simulink model "RB_KAIROS_ImpControl_OpSpace_quat_2020b_safety"  (R2020b)
(part 9 of 17)

C = reshape([0.0,0.0,-q6d.*(-t8850-t8864-t10622+t10627+t11928+t12142-t12808-t12904-t14301-t14305-t14353-t14354+t15516+t15519+t15537+t15539+t15543+t15568+t15569+t15587+t15625+t15626+t15634+t15736+t15867+t15870+t15882+t15885+t15909+t15910+t15967+t15969)-q3d.*(-t5516-t5522-t5589-t5597-t6249-t6602-t7763-t8161+t8844+t8878+t9078+t9084+t9425+t9485+t10324+t10356+t10401+t10512+t10538+t10559+t10594+t10651+t10900+t10919+t10934+t11254+t11258+t11359+t11365+t11539+t11540+t11578+t11596+t11706+t11713+t11715+t11812+t12043+t12084+t12309+t12313+t12340+t12555+t12845+t13109+t13116+t13277+t13286+t13318+t13710+t13918+t13933+t14059+t14102+t14109+t14118+t14133+t14236+t14356+t14358+t14378+t14551+t14817+t14826+t15052+t15058+t15246+t15261+t15399+t15423+t15425+t15433+t15438+t15509+t15510+t15514+t15524+t15613+t15947+t15954+t15988+t15990+t16002+t16003+t16022+t16024)-q4d.*(t5283+t5287+t7042+t7055+t9480+t9626+t10643+t10682+t10838+t10843+t11138+t11325-t12230+t12246+t12314-t12541+t12547-t12593-t12625+t12700+t12876+t12880+t13094+t13095+t13193-t13254-t13453-t13465+t13655+t13721+t13739-t13754-t13765+t13953+t14036+t14149+t14306+t14630+t14634+t14834+t14836-t15211-t15339-t15390-t15410-t15412-t15492-t15493-t15497+t15901+t15949+(t5598.*(t4540+t5.*(t2425-t2468)))./4.0+(t13380.*(t10158+t16.*(t4542-t6448)))./4.0+(t14541.*(t10403+t9.*(t10158+t16.*(t4542-t6448)).*7.35522e-1))./4.0+(t12689.*(t3418-t3879+t4324+t11855+t9.*(t71-t391).*4.5305948634e-2+t17.*(t426-t581).*7.35522e-1+t9.*(t9166-t11658).*7.35522e-1))./4.0+(t2701.*(t5122+t5.*(t2425-t2468).*3.587895))./4.0+(t9830.*(t5124-t6795))./4.0+(t9884.*(t5110-t6808))./4.0+(t10964.*(t4542-t6448))./4.0+(t10936.*(t1589-t2213-t4346+t4355+t9454+t11863+t2772.*(t71-t391)+t2775.*(t71-t391)))./4.0+(t12705.*(t3423+t3845+t3888+t3925+t4339+t9.*(t210+t2107+t7423+t9121).*7.35522e-1+t17.*(t9166-t11658).*7.35522e-1))./4.0+(t12867.*(t10384+t16.*(t4542-t6448).*1.666555))./4.0+(t11340.*(t249-t391.*(1.1e+1./1.25e+2)-t1912.*4.252e-3+t3505+t13496+t693.*(t71-t391)+t784.*(t71-t391)))./4.0+(t14918.*(t10174+t9.*(t10158+t16.*(t4542-t6448))))./4.0+(t12953.*(t2091+t2497+t2579+t2680+t3516+t9.*(t210+t2107+t7423+t9121)+t17.*(t9166-t11658)))./4.0+(t12945.*(t1987-t2621+t3452+t11654+t9.*(t71-t391).*6.1597e-2+t17.*(t426-t581)+t9.*(t9166-t11658)))./4.0+t15.*t12396.*(t4542-t6448).*3.064865e-1+(t15.*t13140.*(t4542-t6448))./4.0)-q2d.*t16467-q1d.*t16482+q7d.*(t10657+t10678+t12523+t12525-t13534-t13699-t16028+t16029+t16034-t16035+t16042+t16061+(t14185.*(t3418-t3879+t4324+t11855+t9.*(t71-t391).*4.5305948634e-2+t17.*(t426-t581).*7.35522e-1+t9.*(t9166-t11658).*7.35522e-1))./4.0+(t14280.*(t1987-t2621+t3452+t11654+t9.*(t71-t391).*6.1597e-2+t17.*(t426-t581)+t9.*(t9166-t11658)))./4.0)-q5d.*(t7290+t7292+t8876+t8913+t10169+t10541+t11057+t11063+t12519+t12522+t12610+t12611+t12793+t12805+t14199+t14202+t14263+t14316+t14319+t14331+t14336+t14432+t14466+t14469+t14484+t14516+t14520+t14593+t14594+t14746+t14978+t14983+t15086+t15091+t15198+t15203+t15213+t15382+t15404+t15405+t15408+t15528+t15929+t15930+t15977+t15979+t15995+t15996+t16015+t16016),q7d.*(t10657+t10678+t12523+t12525-t13534-t13699+t15165+t15166+t15271+t15273+(t10149.*(t10403+t9.*(t10158+t16.*(t4542-t6448)).*7.35522e-1))./4.0+(t14185.*(t3418-t3879+t4324-t5228+t5802+t9.*(t71-t391).*4.5305948634e-2+t17.*(t426-t581).*7.35522e-1))./4.0+(t14280.*(t1987-t2621+t3452-t4730+t5359+t9.*(t71-t391).*6.1597e-2+t17.*(t426-t581)))./4.0+(t11470.*(t10174+t9.*(t10158+t16.*(t4542-t6448))))./4.0)-q6d.*(-t8850-t8864-t10622+t10627+t11928+t12142-t12808-t12904+t13461+t13472+t13649+t13660+t13669+t13797+t13799+t13856+t14045+t14051+t14065+t14233+t14240-t14301-t14305-t14353-t14354+t14371+t14563+t14564+t15034+t15048+t15185+t15192)+phid.*t16482-q5d.*t16367-q2d.*t16419-q3d.*(-t5516-t5522-t5589-t5597-t6249-t6602-t7400-t7763-t7840-t7965-t8161+t8352+t8368+t8386+t8403+t8419+t8474+t8513+t8534+t8844+t8878+t9078+t9084+t9307+t9425+t9449+t9474+t9482+t9485+t9510+t9514+t9905+t9906+t10318+t10531+t11150+t11254+t11258+t11546+t11570+t11578+t11596+t11812+t11825+t11841+t11926+t12132+t12286+t12288+t12303+t12338+t12340+t12586+t12811+t12983+t12985+t13109+t13116+t13277+t13286+t13318+t13370+t13383+t13394+t13601+t13611+t13710+t13890+t13979+t13984+t13992+t14241+t14733+t14737+t14817+t14826+t14987+t14994+t15052+t15058+t15149+t15158+t15380+t15388+t5.*t12.*t6431.*2.01382560198e-1+t5.*t12.*t7224.*6.23745e-2)-q4d.*(t5283+t5287+t7042+t7055+t9480-t9620+t9626+t9629+t9718-t10012+t10034-t10138+t10317-t10448+t10621+t10643+t10682+t10838+t10843+t10972+t11138-t11241+t11325+t11687-t11873-t11885+t12119+t12184-t12231-t12255+t12605+t12876+t12880-t12966+t12968+t13094+t13095+t13193+t13342-t13359-t13425+t13655-t13727-t13850-t14140+t14508+t14630+t14634+t14771+t14834+t14836+t15143+t15378+(t5598.*(t4540+t5.*(t2425-t2468)))./4.0+(t8713.*(t10158+t16.*(t4542-t6448)))./4.0+(t9187.*(t10403+t9.*(t10158+t16.*(t4542-t6448)).*7.35522e-1))./4.0+(t12689.*(t3418-t3879+t4324-t5228+t5802+t9.*(t71-t391).*4.5305948634e-2+t17.*(t426-t581).*7.35522e-1))./4.0+(t12945.*(t1987-t2621+t3452-t4730+t5359+t9.*(t71-t391).*6.1597e-2+t17.*(t426-t581)))./4.0+(t10936.*(t1589-t2213+t3195-t4346+t4355+t4748.*7.35522e-1+t2772.*(t71-t391)+t2775.*(t71-t391)))./4.0+(t2701.*(t5122+t5.*(t2425-t2468).*3.587895))./4.0+(t4557.*(t5124-t6795))./4.0+(t4774.*(t5110-t6808))./4.0+(t6750.*(t4542-t6448))./4.0+(t6744.*(t10384+t16.*(t4542-t6448).*1.666555))./4.0+(t11340.*(t249-t391.*(1.1e+1./1.25e+2)-t1912.*4.252e-3+t3505+t5357+t693.*(t71-t391)+t784.*(t71-t391)))./4.0+(t10753.*(t10174+t9.*(t10158+t16.*(t4542-t6448))))./4.0+t15.*t7039.*(t4542-t6448).*3.064865e-1+(t15.*t9236.*(t4542-t6448))./4.0),phid.*t16467+q7d.*t16209+q6d.*t16303-q4d.*t16360+q1d.*t16419-q5d.*(-t5605-t5612+t7342+t7377+t9411+t9440+t10010+t10405+t10660+t10693+t10828+t10837+t11089+t11096-t11471+t11485+t11690+t11728-t11733-t11939+t11954+t12055-t12061-t12070+t12238-t12244+t12259-t12412-t12612-t12613+t12713+t12851+t12868+t12950+t12967-t13153-t13222-t13424-t13598-t14014+t14410+t14412+t14699+t14703+t14910+t15116+(t7646.*(t10158+t16.*(t4542-t6448)))./4.0+(t7799.*(t10403+t9.*(t10158+t16.*(t4542-t6448)).*7.35522e-1))./4.0+(t6014.*(t10384+t16.*(t4542-t6448).*1.666555))./4.0+(t9537.*(t10174+t9.*(t10158+t16.*(t4542-t6448))))./4.0)+q3d.*(t5536+t5542+t5619+t6200-t6503+t6570+t7339+t7363+t7803+t7804+t7891+t7897+t7957+t7958+t8295+t8304+t8381+t8421+t8977+t8987+t9092+t9339+t9388+t9674+t9678+t9826+t9865+t10056+t10076+t10237+t10273+t10319+t10981+t10986+t11015+t11071+t11440+t11553+t11563+t11669+t11673+t11711+t11741+t11906+t11913+t11989+t12082+t12234+t12245+t12320+t12463+t12632+t12641+t12745+t12977+t13131+t13133+t13480+t13493+t13499+t13528+t13587+t13744+t13889+t13898+t13986+t13989+t14143+t14426+t14427+t14716+t14720+t15084+t15085+t15283+t15284),phid.*(-t5516-t5522-t5589-t5597-t6249-t6602-t7763-t8161+t8844+t8878+t9078+t9084+t9425+t9485+t10324+t10356+t10401+t10512+t10538+t10559+t10594+t10651+t10900+t10919+t10934+t11254+t11258+t11359+t11365+t11539+t11540+t11578+t11596+t11706+t11713+t11715+t11812+t12043+t12084+t12309+t12313+t12340+t12555+t12845+t13109+t13116+t13277+t13286+t13318+t13710+t13918+t13933+t14059+t14102+t14109+t14118+t14133+t14236+t14356+t14358+t14378+t14551+t14817+t14826+t15052+t15058+t15246+t15261+t15399+t15423+t15425+t15433+t15438+t15509+t15510+t15514+t15524+t15613+t15947+t15954+t15988+t15990+t16002+t16003+t16022+t16024)+q7d.*t16201-q6d.*(-t7373-t7381+t9796+t9808+t11549+t11891+t11904+t11999+t12921+t12933+t13020+t13043+t13051+t13087+t13088+t13128+t13247+t13252+t13310+t13330+t13336+t13395+t13403+t13510+t13524+t13701+t13957+t13961+t14653+t14659+t14828+t14833)+q1d.*(-t5516-t5522-t5589-t5597-t6249-t6602-t7400-t7763-t7840-t7965-t8161+t8352+t8368+t8386+t8403+t8419+t8474+t8513+t8534+t8844+t8878+t9078+t9084+t9307+t9425+t9449+t9474+t9482+t9485+t9510+t9514+t9905+t9906+t10318+t10531+t11150+t11254+t11258+t11546+t11570+t11578+t11596+t11812+t11825+t11841+t11926+t12132+t12286+t12288+t12303+t12338+t12340+t12586+t12811+t12983+t12985+t13109+t13116+t13277+t13286+t13318+t13370+t13383+t13394+t13601+t13611+t13710+t13890+t13979+t13984+t13992+t14241+t14733+t14737+t14817+t14826+t14987+t14994+t15052+t15058+t15149+t15158+t15380+t15388+t5.*t12.*t6431.*2.01382560198e-1+t5.*t12.*t7224.*6.23745e-2)-q4d.*(t7036+t7056-t7658+t8022+t8678-t9347+t9360-t9412+t9775+t9813+t10020+t10022+t10025+t10043+t10371+t10528+t10968+t11177-t11186+t11351-t11367+t11698+t11946+t11949+t12105-t12129-t12135+t12144+t12165+t12370-t12408-t12416-t12471+t12830-t12870-t13041-t13200-t13283-t13653-t13873+t13877+t13950+t13951+t14135+t14141+t14176-t14177+t14738+t14995+(t6677.*(t10158+t16.*(t4542-t6448)))./4.0+(t6540.*(t10403+t9.*(t10158+t16.*(t4542-t6448)).*7.35522e-1))./4.0+(t536.*(t5122+t5.*(t2425-t2468).*3.587895))./4.0+((t923-t1076).*(t5110-t6808))./4.0+((t2812-t2860).*(t4542-t6448))./4.0+(t5050.*(t10384+t16.*(t4542-t6448).*1.666555))./4.0+(t9048.*(t10174+t9.*(t10158+t16.*(t4542-t6448))))./4.0+t15.*t4286.*(t4542-t6448).*3.064865e-1+(t15.*t6196.*(t4542-t6448))./4.0)-q5d.*(-t7281-t7284+t7345+t9363+t9413+t10264+t10290+t11012+t11019+t11131+t11145+t11222+t11225+t11291+t11368+t11375-t11412-t11428+t11541+t11545-t11581-t11591+t11641+t11768+t11831-t11869-t11883+t11900+t11903+t12300+t12449+t12918+t12930+t13044+t13050+t13267+t13646+t13677+t13681+t13763+t13777+t14111+t14115+t14370+t14386+t14691+t14693+t14886+t14890+t6.*t15.*(t4540+t5.*(t2425-t2468)).*7.326866269e-3)-q2d.*(t5536+t5542+t5619+t6200-t6503+t6570+t7339+t7363+t7803+t7804+t7891+t7897+t7957+t7958+t8295+t8304+t8381+t8421+t8977+t8987+t9092+t9339+t9388+t9674+t9678+t9826+t9865+t10056+t10076+t10237+t10273+t10319+t10981+t10986+t11015+t11071+t11440+t11553+t11563+t11669+t11673+t11711+t11741+t11906+t11913+t11989+t12082+t12234+t12245+t12320+t12463+t12632+t12641+t12745+t12977+t13131+t13133+t13480+t13493+t13499+t13528+t13587+t13744+t13889+t13898+t13986+t13989+t14143+t14426+t14427+t14716+t14720+t15084+t15085+t15283+t15284),q5d.*(t8808+t8820+t9138+t9343-t10997-t10998+t11097+t11101+t11270+t11284+t11360+t11384-t11511-t11517+t11528+t11542-t11550+t11840+t11853-t12393-t12803-t12903-t13160+t13238+t13251+t13324+t13334-t13538+t13926+t13928+t14116+t14121+t14584+t14754+(t5441.*(t10158+t16.*(t4542-t6448)))./4.0+(t5213.*(t10403+t9.*(t10158+t16.*(t4542-t6448)).*7.35522e-1))./4.0+(t3266.*(t5110-t6808))./4.0+(t4879.*(t4542-t6448))./4.0+(t3780.*(t10384+t16.*(t4542-t6448).*1.666555))./4.0+(t7538.*(t10174+t9.*(t10158+t16.*(t4542-t6448))))./4.0)+phid.*(t5283+t5287+t7042+t7055+t9480+t9626+t10643+t10682+t10838+t10843+t11138+t11325-t12230+t12246+t12314-t12541+t12547-t12593-t12625+t12700+t12876+t12880+t13094+t13095+t13193-t13254-t13453-t13465+t13655+t13721+t13739-t13754-t13765+t13953+t14036+t14149+t14306+t14630+t14634+t14834+t14836-t15211-t15339-t15390-t15410-t15412-t15492-t15493-t15497+t15901+t15949+(t5598.*(t4540+t5.*(t2425-t2468)))./4.0+(t13380.*(t10158+t16.*(t4542-t6448)))./4.0+(t14541.*(t10403+t9.*(t10158+t16.*(t4542-t6448)).*7.35522e-1))./4.0+(t12689.*(t3418-t3879+t4324+t11855+t9.*(t71-t391).*4.5305948634e-2+t17.*(t426-t581).*7.35522e-1+t9.*(t9166-t11658).*7.35522e-1))./4.0+(t2701.*(t5122+t5.*(t2425-t2468).*3.587895))./4.0+(t9830.*(t5124-t6795))./4.0+(t9884.*(t5110-t6808))./4.0+(t10964.*(t4542-t6448))./4.0+(t10936.*(t1589-t2213-t4346+t4355+t9454+t11863+t2772.*(t71-t391)+t2775.*(t71-t391)))./4.0+(t12705.*(t3423+t3845+t3888+t3925+t4339+t9.*(t210+t2107+t7423+t9121).*7.35522e-1+t17.*(t9166-t11658).*7.35522e-1))./4.0+(t12867.*(t10384+t16.*(t4542-t6448).*1.666555))./4.0+(t11340.*(t249-t391.*(1.1e+1./1.25e+2)-t1912.*4.252e-3+t3505+t13496+t693.*(t71-t391)+t784.*(t71-t391)))./4.0+(t14918.*(t10174+t9.*(t10158+t16.*(t4542-t6448))))./4.0+(t12953.*(t2091+t2497+t2579+t2680+t3516+t9.*(t210+t2107+t7423+t9121)+t17.*(t9166-t11658)))./4.0+(t12945.*(t1987-t2621+t3452+t11654+t9.*(t71-t391).*6.1597e-2+t17.*(t426-t581)+t9.*(t9166-t11658)))./4.0+t15.*t12396.*(t4542-t6448).*3.064865e-1+(t15.*t13140.*(t4542-t6448))./4.0)+q7d.*t16192+q2d.*t16360+q6d.*(-t8786-t8793+t8848+t11052+t11062-t11847-t11974+t12684+t12708+t12795+t12810+t12855+t12863+t12875-t12969-t12975+t13003+t13004+t13061+t13075+t13076-t13096-t13100+t13188+t13469+t13473+t13648+t14509+t14510+t14618+t14625+t7.*t8.*(t4542-t6448).*1.17633784675e-2)+q1d.*(t5283+t5287+t7042+t7055+t9480-t9620+t9626+t9629+t9718-t10012+t10034-t10138+t10317-t10448+t10621+t10643+t10682+t10838+t10843+t10972+t11138-t11241+t11325+t11687-t11873-t11885+t12119+t12184-t12231-t12255+t12605+t12876+t12880-t12966+t12968+t13094+t13095+t13193+t13342-t13359-t13425+t13655-t13727-t13850-t14140+t14508+t14630+t14634+t14771+t14834+t14836+t15143+t15378+(t5598.*(t4540+t5.*(t2425-t2468)))./4.0+(t8713.*(t10158+t16.*(t4542-t6448)))./4.0+(t9187.*(t10403+t9.*(t10158+t16.*(t4542-t6448)).*7.35522e-1))./4.0+(t12689.*(t3418-t3879+t4324-t5228+t5802+t9.*(t71-t391).*4.5305948634e-2+t17.*(t426-t581).*7.35522e-1))./4.0+(t12945.*(t1987-t2621+t3452-t4730+t5359+t9.*(t71-t391).*6.1597e-2+t17.*(t426-t581)))./4.0+(t10936.*(t1589-t2213+t3195-t4346+t4355+t4748.*7.35522e-1+t2772.*(t71-t391)+t2775.*(t71-t391)))./4.0+(t2701.*(t5122+t5.*(t2425-t2468).*3.587895))./4.0+(t4557.*(t5124-t6795))./4.0+(t4774.*(t5110-t6808))./4.0+(t6750.*(t4542-t6448))./4.0+(t6744.*(t10384+t16.*(t4542-t6448).*1.666555))./4.0+(t11340.*(t249-t391.*(1.1e+1./1.25e+2)-t1912.*4.252e-3+t3505+t5357+t693.*(t71-t391)+t784.*(t71-t391)))./4.0+(t10753.*(t10174+t9.*(t10158+t16.*(t4542-t6448))))./4.0+t15.*t7039.*(t4542-t6448).*3.064865e-1+(t15.*t9236.*(t4542-t6448))./4.0)+q3d.*(t7036+t7056-t7658+t8022+t8678-t9347+t9360-t9412+t9775+t9813+t10020+t10022+t10025+t10043+t10371+t10528+t10968+t11177-t11186+t11351-t11367+t11698+t11946+t11949+t12105-t12129-t12135+t12144+t12165+t12370-t12408-t12416-t12471+t12830-t12870-t13041-t13200-t13283-t13653-t13873+t13877+t13950+t13951+t14135+t14141+t14176-t14177+t14738+t14995+(t6677.*(t10158+t16.*(t4542-t6448)))./4.0+(t6540.*(t10403+t9.*(t10158+t16.*(t4542-t6448)).*7.35522e-1))./4.0+(t536.*(t5122+t5.*(t2425-t2468).*3.587895))./4.0+((t923-t1076).*(t5110-t6808))./4.0+((t2812-t2860).*(t4542-t6448))./4.0+(t5050.*(t10384+t16.*(t4542-t6448).*1.666555))./4.0+(t9048.*(t10174+t9.*(t10158+t16.*(t4542-t6448))))./4.0+t15.*t4286.*(t4542-t6448).*3.064865e-1+(t15.*t6196.*(t4542-t6448))./4.0),-q4d.*(t8808+t8820+t9138+t9343-t10997-t10998+t11097+t11101+t11270+t11284+t11360+t11384-t11511-t11517+t11528+t11542-t11550+t11840+t11853-t12393-t12803-t12903-t13160+t13238+t13251+t13324+t13334-t13538+t13926+t13928+t14116+t14121+t14584+t14754+(t5441.*(t10158+t16.*(t4542-t6448)))./4.0+(t5213.*(t10403+t9.*(t10158+t16.*(t4542-t6448)).*7.35522e-1))./4.0+(t3266.*(t5110-t6808))./4.0+(t4879.*(t4542-t6448))./4.0+(t3780.*(t10384+t16.*(t4542-t6448).*1.666555))./4.0+(t7538.*(t10174+t9.*(t10158+t16.*(t4542-t6448))))./4.0)+q7d.*t16184+q6d.*t16230+q1d.*t16367+q2d.*(-t5605-t5612+t7342+t7377+t9411+t9440+t10010+t10405+t10660+t10693+t10828+t10837+t11089+t11096-t11471+t11485+t11690+t11728-t11733-t11939+t11954+t12055-t12061-t12070+t12238-t12244+t12259-t12412-t12612-t12613+t12713+t12851+t12868+t12950+t12967-t13153-t13222-t13424-t13598-t14014+t14410+t14412+t14699+t14703+t14910+t15116+(t7646.*(t10158+t16.*(t4542-t6448)))./4.0+(t7799.*(t10403+t9.*(t10158+t16.*(t4542-t6448)).*7.35522e-1))./4.0+(t6014.*(t10384+t16.*(t4542-t6448).*1.666555))./4.0+(t9537.*(t10174+t9.*(t10158+t16.*(t4542-t6448))))./4.0)+phid.*(t7290+t7292+t8876+t8913+t10169+t10541+t11057+t11063+t12519+t12522+t12610+t12611+t12793+t12805+t14199+t14202+t14263+t14316+t14319+t14331+t14336+t14432+t14466+t14469+t14484+t14516+t14520+t14593+t14594+t14746+t14978+t14983+t15086+t15091+t15198+t15203+t15213+t15382+t15404+t15405+t15408+t15528+t15929+t15930+t15977+t15979+t15995+t15996+t16015+t16016)+q3d.*(-t7281-t7284+t7345+t9363+t9413+t10264+t10290+t11012+t11019+t11131+t11145+t11222+t11225+t11291+t11368+t11375-t11412-t11428+t11541+t11545-t11581-t11591+t11641+t11768+t11831-t11869-t11883+t11900+t11903+t12300+t12449+t12918+t12930+t13044+t13050+t13267+t13646+t13677+t13681+t13763+t13777+t14111+t14115+t14370+t14386+t14691+t14693+t14886+t14890+t6.*t15.*(t4540+t5.*(t2425-t2468)).*7.326866269e-3),phid.*(-t8850-t8864-t10622+t10627+t11928+t12142-t12808-t12904-t14301-t14305-t14353-t14354+t15516+t15519+t15537+t15539+t15543+t15568+t15569+t15587+t15625+t15626+t15634+t15736+t15867+t15870+t15882+t15885+t15909+t15910+t15967+t15969)+q1d.*(-t8850-t8864-t10622+t10627+t11928+t12142-t12808-t12904+t13461+t13472+t13649+t13660+t13669+t13797+t13799+t13856+t14045+t14051+t14065+t14233+t14240-t14301-t14305-t14353-t14354+t14371+t14563+t14564+t15034+t15048+t15185+t15192)+q7d.*t16070-q5d.*t16230-q2d.*t16303+q3d.*(-t7373-t7381+t9796+t9808+t11549+t11891+t11904+t11999+t12921+t12933+t13020+t13043+t13051+t13087+t13088+t13128+t13247+t13252+t13310+t13330+t13336+t13395+t13403+t13510+t13524+t13701+t13957+t13961+t14653+t14659+t14828+t14833)-q4d.*(-t8786-t8793+t8848+t11052+t11062-t11847-t11974+t12684+t12708+t12795+t12810+t12855+t12863+t12875-t12969-t12975+t13003+t13004+t13061+t13075+t13076-t13096-t13100+t13188+t13469+t13473+t13648+t14509+t14510+t14618+t14625+t7.*t8.*(t4542-t6448).*1.17633784675e-2),-q1d.*(t10657+t10678+t12523+t12525-t13534-t13699+t15165+t15166+t15271+t15273+(t10149.*(t10403+t9.*(t10158+t16.*(t4542-t6448)).*7.35522e-1))./4.0+(t14185.*(t3418-t3879+t4324-t5228+t5802+t9.*(t71-t391).*4.5305948634e-2+t17.*(t426-t581).*7.35522e-1))./4.0+(t14280.*(t1987-t2621+t3452-t4730+t5359+t9.*(t71-t391).*6.1597e-2+t17.*(t426-t581)))./4.0+(t11470.*(t10174+t9.*(t10158+t16.*(t4542-t6448))))./4.0)-q6d.*t16070-q5d.*t16184-q4d.*t16192-q3d.*t16201-q2d.*t16209-phid.*(t10657+t10678+t12523+t12525-t13534-t13699-t16028+t16029+t16034-t16035+t16042+t16061+(t14185.*(t3418-t3879+t4324+t11855+t9.*(t71-t391).*4.5305948634e-2+t17.*(t426-t581).*7.35522e-1+t9.*(t9166-t11658).*7.35522e-1))./4.0+(t14280.*(t1987-t2621+t3452+t11654+t9.*(t71-t391).*6.1597e-2+t17.*(t426-t581)+t9.*(t9166-t11658)))./4.0),0.0,0.0,q4d.*t16453+q2d.*t16470+q6d.*(-t10580+t10587+t11945+t12174-t12785-t12888-t14289-t14345+t15521+t15522+t15544+t15546+t15547+t15578+t15583+t15594+t15632+t15639+t15644+t15740+t15872+t15873+t15887+t15888+t15911+t15912+t15970+t15972+t9.*(t10403+t9.*(t10158+t16.*(t4542-t6448)).*7.35522e-1).*1.539925e-2+t8.*(t4542-t6448).*5.01208083475e-2+t16.*(t4542-t6448).*1.17633784675e-2+t9.*(t10174+t9.*(t10158+t16.*(t4542-t6448))).*1.13264871585e-2)+q7d.*(t10600+t10609+t12501+t12510-t13551-t13712+t16032+t16037+t16049+t16067+(t14299.*(t2497+t2680+t3516+t9.*(t210+t2107+t7423+t9121)+t17.*(t9166-t11658)))./4.0+(t14209.*(t3418-t3879+t4324+t11855+t9.*(t71-t391).*4.5305948634e-2+t17.*(t426-t581).*7.35522e-1+t9.*(t9166-t11658).*7.35522e-1))./4.0+(t14213.*(t3845+t3925+t4339+t9.*(t210+t2107+t7423+t9121).*7.35522e-1+t17.*(t9166-t11658).*7.35522e-1))./4.0+(t14297.*(t1987-t2621+t3452+t11654+t9.*(t71-t391).*6.1597e-2+t17.*(t426-t581)+t9.*(t9166-t11658)))./4.0)+q1d.*(-t3860+t3958-t4535-t4632-t5577-t5579-t6236-t6371-t6593+t7145+t7153+t7436+t7437+t7459+t7492+t7504+t7532+t7602+t7632+t7637+t7966+t8007+t8125+t8130+t8211+t8293+t8337-t8357+t8363-t8393+t8401+t8472+t8811+t8824+t9464+t9699+t9730+t10082+t10083+t10088+t10097+t10099+t10102+t10311+t10334+t10571+t10575+t10670+t10909+t10913+t11730+t11801+t11803+t11804+t11813+t11814+t11815-t12134+t12158+t12324+t12330-t12430+t12629-t12657+t12685+t12706+t12715-t13065+t13264-t13790+t13792+t13793+t13800+t13801+t13804+t13805+t13806-t14043+t14054+t14313+t14325+t14433+t14587+t14606+t14748+t15252+t15253+t15254+t15255+t15259+t15260+t15327-t15331+t15465-t15467+t15565+t15570+t15622+t15627+t15630+t15734+t15931+t15932+t15940+t15941+t16040+t16044+t16058+t16062+(t12279.*(t1589-t2213+t3195-t4346+t4355+t4748.*7.35522e-1+t2772.*(t71-t391)+t2775.*(t71-t391)))./4.0+(t4356.*(t2425-t2468))./4.0+(t6190.*(t5110-t6808))./4.0+(t8711.*(t4542-t6448))./4.0+(t12484.*(t249-t391.*(1.1e+1./1.25e+2)-t1912.*4.252e-3+t3505+t5357+t693.*(t71-t391)+t784.*(t71-t391)))./4.0)+q5d.*(t7328+t7338+t8774+t8795+t10202+t10562+t11039+t11047+t12499+t12504+t12595+t12596+t12771+t12783+t14211+t14214+t14269+t14328+t14335+t14342+t14344+t14437+t14448+t14451+t14490+t14494+t14498+t14614+t14615+t14751+t14988+t14991+t15105+t15110+t15207+t15208+t15224+t15392+t15413+t15415+t15416+t15532+t15942+t15943+t15981+t15986+t16004+t16007+t16023+t16027)+q3d.*(t5538+t5554+t5559+t5562-t6622+t7789+t8207+t8776+t8806+t9051+t9058+t9390+t9445-t10331+t10339+t10373+t10519-t10526+t10558+t10574+t10650+t10898+t10905+t10908+t11226+t11229-t11392-t11526-t11527+t11537+t11557+t11722-t11732+t11777+t12051+t12072-t12297-t12302+t12310+t12559+t12832+t13086+t13093+t13246+t13261+t13309+t13696-t13936-t14110-t14129+t14231-t14357-t14359+t14548+t14778+t14788+t15029+t15035-t15264+t15265-t15402+t15420-t15441+t15442+t15503-t15513-t15527-t15612-t15956+t15959-t15991+t15992+t15998+t16017+(t8794.*(t263+t1265-t7252-t5.*t12.*1.0442e-1))./4.0+(t13178.*(t3418-t3879+t4324+t11855+t9.*(t71-t391).*4.5305948634e-2+t17.*(t426-t581).*7.35522e-1+t9.*(t9166-t11658).*7.35522e-1))./4.0+(t12385.*(t6853-t6864))./4.0+(t11247.*(t6806-t8574))./4.0+(t12185.*(t6452-t8229))./4.0+(t11720.*(t6801-t8594))./4.0+(t12669.*(t6452-t8229))./4.0+(t14380.*(t6472-t9256))./4.0+(t14057.*(t6847-t9563))./4.0+(t8166.*(t1786+t2973-t7703-t5.*t12.*3.746479959e-1))./4.0+(t13377.*(t1987-t2621+t3452+t11654+t9.*(t71-t391).*6.1597e-2+t17.*(t426-t581)+t9.*(t9166-t11658)))./4.0+t12.*(t881-t912).*(t2425-t2468).*8.07151e-1),q3d.*(t5538+t5554+t5559+t5562-t6622+t7372+t7789+t7820+t7954+t8207+t8336+t8356+t8364+t8391+t8402+t8473-t8490-t8514+t8776+t8806+t9051+t9058+t9281+t9390+t9445+t9465-t9494-t9503-t9504-t9911-t9921+t10336+t10508+t11155+t11226+t11229+t11537+t11557-t11571+t11777-t11838+t11920-t12287-t12289+t12310-t12334+t12577+t13086+t13093+t13246+t13261+t13309-t13388-t13612+t13626+t13696-t13914-t13973-t13999+t14000-t14248-t14732+t14778+t14788-t14984+t15029+t15035-t15169+t15172-t15393+t15395+((t6853-t6864).*(t921+t1317-t5853))./4.0+(t11356.*(-t1476-t1540+t2091+t2165+t2579+t8.*(t260+t468+t570+t2298)))./4.0+(t13178.*(t3418-t3879+t4324-t5228+t5802+t9.*(t71-t391).*4.5305948634e-2+t17.*(t426-t581).*7.35522e-1))./4.0+(t13377.*(t1987-t2621+t3452-t4730+t5359+t9.*(t71-t391).*6.1597e-2+t17.*(t426-t581)))./4.0+(t5860.*(t6806-t8574))./4.0+(t6970.*(t6801-t8594))./4.0+(t8310.*(t6452-t8229))./4.0+(t9525.*(t6452-t8229))./4.0+(t8227.*(t6847-t9563))./4.0+(t9744.*(t6472-t9256))./4.0+(t8794.*(t263-t283-t310+t1265))./4.0+(t10942.*(-t3045-t3218+t3458+t3539+t3878+t8.*(t260+t468+t570+t2298).*1.666555))./4.0+t12.*(t881-t912).*(t2425-t2468).*8.07151e-1-t5.*t12.*t6447.*2.01382560198e-1-t5.*t12.*t7236.*6.23745e-2)+q4d.*t16411+q6d.*(-t10580+t10587+t11945+t12174-t12785-t12888+t13485+t13494+t13662+t13685+t13690+t13830+t13831+t13870+t14072+t14081+t14093+t14243+t14245-t14289-t14345+t14393+t14575+t14579+t15059+t15062+t15204+t15206+t9.*(t10403+t9.*(t10158+t16.*(t4542-t6448)).*7.35522e-1).*1.539925e-2+t8.*(t4542-t6448).*5.01208083475e-2+t16.*(t4542-t6448).*1.17633784675e-2+t9.*(t10174+t9.*(t10158+t16.*(t4542-t6448))).*1.13264871585e-2)+q5d.*(t7328+t7338+t8774+t8795+t10202+t10562+t11039+t11047-t12176-t12438+t12441+t12499+t12504+t12595+t12596-t12703+t12771+t12783-t12852-t12972+t13074+t13505-t13584+t13693+t13958+t14215+t14448+t14451+t14494+t14498-t14736-t14992+t15150+t15312+((t6806-t8574).*(t921+t1317-t5853))./4.0+((t6452-t8229).*(t2810+t2988-t7937))./4.0+(t14213.*(t2740+t3849+t3968+t3972-t5255+t17.*(t260+t468+t570+t2298).*7.35522e-1))./4.0+(t13189.*(t3418-t3879+t4324-t5228+t5802+t9.*(t71-t391).*4.5305948634e-2+t17.*(t426-t581).*7.35522e-1))./4.0+(t13391.*(t1987-t2621+t3452-t4730+t5359+t9.*(t71-t391).*6.1597e-2+t17.*(t426-t581)))./4.0+(t12508.*(t1492+t2158+t2696-t4727))./4.0+(t12307.*(t3063+t3528+t3966-t5230))./4.0+(t10577.*(t495+t572+t1838+t2069+t2107))./4.0+(t10164.*(t2437+t2648+t3129+t3384+t3574))./4.0+(t5853.*(t6806-t8574))./4.0+(t6535.*(t6801-t8594))./4.0+(t7937.*(t6452-t8229))./4.0+(t8791.*(t6452-t8229))./4.0+(t14299.*(t824+t2543+t2699+t2707-t4767+t17.*(t260+t468+t570+t2298)))./4.0+t16.*t8227.*(t6452-t8229).*4.1663875e-1+(t16.*t9744.*(t6452-t8229))./4.0)+q7d.*(t10600+t10609+t12501+t12510-t13551-t13712+t15181+t15182+t15289+t15293-t15358-t15476+(t14209.*(t3418-t3879+t4324-t5228+t5802+t9.*(t71-t391).*4.5305948634e-2+t17.*(t426-t581).*7.35522e-1))./4.0+(t14297.*(t1987-t2621+t3452-t4730+t5359+t9.*(t71-t391).*6.1597e-2+t17.*(t426-t581)))./4.0)-phid.*(-t3860+t3958-t4535-t4632-t5577-t5579-t6236-t6371-t6593+t7145+t7153+t7436+t7437+t7459+t7492+t7504+t7532+t7602+t7632+t7637+t7966+t8007+t8125+t8130+t8211+t8293+t8337-t8357+t8363-t8393+t8401+t8472+t8811+t8824+t9464+t9699+t9730+t10082+t10083+t10088+t10097+t10099+t10102+t10311+t10334+t10571+t10575+t10670+t10909+t10913+t11730+t11801+t11803+t11804+t11813+t11814+t11815-t12134+t12158+t12324+t12330-t12430+t12629-t12657+t12685+t12706+t12715-t13065+t13264-t13790+t13792+t13793+t13800+t13801+t13804+t13805+t13806-t14043+t14054+t14313+t14325+t14433+t14587+t14606+t14748+t15252+t15253+t15254+t15255+t15259+t15260+t15327-t15331+t15465-t15467+t15565+t15570+t15622+t15627+t15630+t15734+t15931+t15932+t15940+t15941+t16040+t16044+t16058+t16062+(t12279.*(t1589-t2213+t3195-t4346+t4355+t4748.*7.35522e-1+t2772.*(t71-t391)+t2775.*(t71-t391)))./4.0+(t4356.*(t2425-t2468))./4.0+(t6190.*(t5110-t6808))./4.0+(t8711.*(t4542-t6448))./4.0+(t12484.*(t249-t391.*(1.1e+1./1.25e+2)-t1912.*4.252e-3+t3505+t5357+t693.*(t71-t391)+t784.*(t71-t391)))./4.0)+q2d.*(t5229+t5533+t6212+t6293+t6300+t6319+t6357+t6437+t6577+t6643+t6647+t7330+t7388+t7791+t7823+t7908+t8313+t8353-t8367-t8392+t8400+t8447-t8452+t8849+t9346+t9356-t9417+t9526+t9623-t9756+t9757+t9836+t9846+t10236+t10350-t10364+t10451+t10535+t10867+t11076-t11235+t11244+t11724+t11736+t11784+t12057-t12155+t12235+t12247-t12544+t12545-t12679+t12721-t12996+t13010+t13024+t13506+t13542+t13603+t13776-t13814-t13836+t13892+t13906-t14052-t14060-t14075+t14163-t14310+t14312-t14365+t14604+t15072+t15080+t15275+t15281+t15368-t15371-t15479+t15483+((t7.*(t4650+t34.*(t2425-t2468)).*1.225946+t47.*(t2425-t2468).*1.225946).*(t921+t1317-t5853))./4.0+(t6767.*(t30.*(t2425-t2468)+t68.*(t2425-t2468)))./4.0+((t7.*(t4650+t34.*(t2425-t2468))+t47.*(t2425-t2468)).*(t2810+t2988-t7937))./4.0+(t6988.*(t6806-t8574))./4.0+(t7875.*(t6801-t8594))./4.0+(t9216.*(t6452-t8229))./4.0+(t9992.*(t6452-t8229))./4.0+(t4611.*(t30.*(t2425-t2468).*3.587895+t68.*(t2425-t2468).*3.587895))./4.0+(t9967.*(t4654+t15.*(t4650+t34.*(t2425-t2468))))./4.0+(t11470.*(t8329+t17.*(t16.*(t30.*(t2425-t2468)+t68.*(t2425-t2468))+t8.*(t7.*(t4650+t34.*(t2425-t2468))+t47.*(t2425-t2468)))))./4.0+t4.*t3318.*(t2425-t2468).*8.07151e-1+t12.*t3316.*(t2425-t2468).*8.07151e-1+(t4.*t4908.*(t2425-t2468))./4.0+(t12.*t4906.*(t2425-t2468))./4.0),q7d.*(t8350.*3.867742437e-3+t10735+t13315+t13529+t14946+t14951+t15092+t15097+t15102+t15107+t15300+t15306+t9.*(t16.*(t30.*(t2425-t2468)+t68.*(t2425-t2468))+t8.*(t7.*(t4650+t34.*(t2425-t2468))+t47.*(t2425-t2468))).*1.563719772e-3+t17.*(t4654+t15.*(t4650+t34.*(t2425-t2468))).*1.563719772e-3)-phid.*t16470-q4d.*(t5297+t7666+t7719-t9159+t9267+t9274+t9418+t9421+t9542+t9551-t9573+t9651+t9886+t9889+t9988+t10000+t10002+t10262+t10479+t10891+t10902+t11093+t11279+t11443+t11446+t11620+t11771+t11776+t11790+t11851+t11931+t12439+t12445+t12639+t12649+t12982+t13139+t13141+t13190+t13253+t13260+t13552+t13575+t13583+t13592+t13596+t14002+t14232+t14234+t14487+t14489+t14956+t14958+t15189+t15193+(t7796.*(t9.*(t16.*(t30.*(t2425-t2468)+t68.*(t2425-t2468))+t8.*(t7.*(t4650+t34.*(t2425-t2468))+t47.*(t2425-t2468)))+t17.*(t4654+t15.*(t4650+t34.*(t2425-t2468)))))./4.0+(t5331.*(t30.*(t2425-t2468)+t68.*(t2425-t2468)))./4.0+(t6046.*(t16.*(t30.*(t2425-t2468)+t68.*(t2425-t2468))+t8.*(t7.*(t4650+t34.*(t2425-t2468))+t47.*(t2425-t2468))))./4.0+(t4024.*(t16.*(t30.*(t2425-t2468)+t68.*(t2425-t2468)).*1.666555+t8.*(t7.*(t4650+t34.*(t2425-t2468))+t47.*(t2425-t2468)).*1.666555))./4.0+t7.*(t7.*(t4650+t34.*(t2425-t2468)).*1.225946+t47.*(t2425-t2468).*1.225946).*8.639075e-2+t30.*(t2425-t2468).*9.5384188575e-2+t34.*(t2425-t2468).*1.8732399795e-1+t68.*(t2425-t2468).*9.5384188575e-2+(t3424.*(t30.*(t2425-t2468).*1.225946+t68.*(t2425-t2468).*1.225946))./4.0+t15.*(t4654+t15.*(t4650+t34.*(t2425-t2468))).*1.059103943995e-1+(t5443.*(t4654+t15.*(t4650+t34.*(t2425-t2468))))./4.0+t7.*(t7.*(t4650+t34.*(t2425-t2468))+t47.*(t2425-t2468)).*1.059103943995e-1+(t5329.*(t9.*(t16.*(t30.*(t2425-t2468)+t68.*(t2425-t2468))+t8.*(t7.*(t4650+t34.*(t2425-t2468))+t47.*(t2425-t2468))).*7.35522e-1+t17.*(t4654+t15.*(t4650+t34.*(t2425-t2468))).*7.35522e-1))./4.0)-q3d.*(t5572+t5576+t5657+t6529+t7405+t7415+t7864+t7865-t7874+t7896+t7917+t7918-t8279+t8307+t8423+t8444+t8946+t8954-t9082-t9403+t9422+t9690+t9693+t9876-t9888+t10114+t10123+t10245+t10304-t10308+t10970+t11046+t11077+t11435+t11624+t11627+t11664-t11670-t11743+t11943+t11956+t12030+t12091-t12258+t12312+t12473-t12633+t12760-t13122-t13540-t13550+t13560+t13571-t13762-t13912-t13921+t14005+t14007-t14158+t14416+t14418+t14711+t14713-t15113-t15114-t15308-t15310+(t5634.*(t6853-t6864))./4.0+(t5648.*(t6806-t8574))./4.0+(t8053.*(t6452-t8229))./4.0+(t7079.*(t6847-t9563))./4.0+(t8191.*(t6834-t9565))./4.0+(t9110.*(t6472-t9256))./4.0+(t10141.*(t6472-t9256))./4.0+t12.*t3243.*(t2425-t2468).*8.07151e-1+(t12.*t4860.*(t2425-t2468))./4.0)-q1d.*(t5229+t5533+t6212+t6293+t6300+t6319+t6357+t6437+t6577+t6643+t6647+t7330+t7388+t7791+t7823+t7908+t8313+t8353-t8367-t8392+t8400+t8447-t8452+t8849+t9346+t9356-t9417+t9526+t9623-t9756+t9757+t9836+t9846+t10236+t10350-t10364+t10451+t10535+t10867+t11076-t11235+t11244+t11724+t11736+t11784+t12057-t12155+t12235+t12247-t12544+t12545-t12679+t12721-t12996+t13010+t13024+t13506+t13542+t13603+t13776-t13814-t13836+t13892+t13906-t14052-t14060-t14075+t14163-t14310+t14312-t14365+t14604+t15072+t15080+t15275+t15281+t15368-t15371-t15479+t15483+((t7.*(t4650+t34.*(t2425-t2468)).*1.225946+t47.*(t2425-t2468).*1.225946).*(t921+t1317-t5853))./4.0+(t6767.*(t30.*(t2425-t2468)+t68.*(t2425-t2468)))./4.0+((t7.*(t4650+t34.*(t2425-t2468))+t47.*(t2425-t2468)).*(t2810+t2988-t7937))./4.0+(t6988.*(t6806-t8574))./4.0+(t7875.*(t6801-t8594))./4.0+(t9216.*(t6452-t8229))./4.0+(t9992.*(t6452-t8229))./4.0+(t4611.*(t30.*(t2425-t2468).*3.587895+t68.*(t2425-t2468).*3.587895))./4.0+(t9967.*(t4654+t15.*(t4650+t34.*(t2425-t2468))))./4.0+(t11470.*(t8329+t17.*(t16.*(t30.*(t2425-t2468)+t68.*(t2425-t2468))+t8.*(t7.*(t4650+t34.*(t2425-t2468))+t47.*(t2425-t2468)))))./4.0+t4.*t3318.*(t2425-t2468).*8.07151e-1+t12.*t3316.*(t2425-t2468).*8.07151e-1+(t4.*t4908.*(t2425-t2468))./4.0+(t12.*t4906.*(t2425-t2468))./4.0)+q6d.*(t8952-t11170+t11723+t12027-t12690+t13257+t13258+t13361+t13443+t13450+t13547+t13549+t13581+t13820+t13917+t13922+t13929+t13938+t14183+t14256+t14259+t14875+t14876+t15011+t15015+t9.*(t9.*(t16.*(t30.*(t2425-t2468)+t68.*(t2425-t2468))+t8.*(t7.*(t4650+t34.*(t2425-t2468))+t47.*(t2425-t2468)))+t17.*(t4654+t15.*(t4650+t34.*(t2425-t2468)))).*1.13264871585e-2+t8.*(t30.*(t2425-t2468)+t68.*(t2425-t2468)).*5.01208083475e-2+t16.*(t30.*(t2425-t2468)+t68.*(t2425-t2468)).*1.17633784675e-2+t8.*(t7.*(t4650+t34.*(t2425-t2468))+t47.*(t2425-t2468)).*1.17633784675e-2+(t5365.*(t8315+t8.*(t30.*(t2425-t2468)+t68.*(t2425-t2468))))./4.0+t17.*(t8329+t17.*(t16.*(t30.*(t2425-t2468)+t68.*(t2425-t2468))+t8.*(t7.*(t4650+t34.*(t2425-t2468))+t47.*(t2425-t2468)))).*1.13264871585e-2+t9.*(t9.*(t16.*(t30.*(t2425-t2468)+t68.*(t2425-t2468))+t8.*(t7.*(t4650+t34.*(t2425-t2468))+t47.*(t2425-t2468))).*7.35522e-1+t17.*(t4654+t15.*(t4650+t34.*(t2425-t2468))).*7.35522e-1).*1.539925e-2)-q5d.*(t5642+t5652+t7414+t7417+t9495+t9508+t10037+t10422+t10746+t10750+t10869+t10870+t11140+t11154-t11488+t11503+t11719+t11754-t11960+t11981+t12064+t12263+t12280+t12728+t12910+t12911+t13017+t13022-t13245-t13272-t13439-t13452-t13602-t14026+t14428+t14430+t14717+t14721+t14931-t14936+t15125-t15129+(t5634.*(t6806-t8574))./4.0+(t8050.*(t6452-t8229))./4.0+t16.*t7079.*(t6452-t8229).*4.1663875e-1+t8.*t7116.*(t6452-t8229).*4.1663875e-1+t16.*t8191.*(t6452-t8229).*1.838805e-1+(t8.*t9112.*(t6452-t8229))./4.0+(t16.*t9110.*(t6452-t8229))./4.0+(t16.*t10141.*(t6452-t8229))./4.0),-q4d.*(t6999+t7020-t7671+t7995+t8667+t9389-t9402-t9415-t9444-t9473-t9484+t9776+t9814+t10023+t10040+t10044+t10049-t10060+t10372+t10529+t10992+t11198+t11379+t11729+t11936+t11940+t12114+t12131+t12154-t12180+t12363-t12436+t12822-t13053-t13066-t13220-t13227-t13301-t13678+t13900+t13944+t13946+t14128+t14134+t14194+t14745-t14749+t15007-t15014+(t6430.*(t1748-t1821))./4.0+(t4064.*(t6806-t8574))./4.0+(t5646.*(t6452-t8229))./4.0+(t5234.*(t8589-t8592))./4.0+(t6884.*(t8219-t8226))./4.0+(t6302.*(t8582-t8586))./4.0+(t8640.*(t8219-t8226))./4.0+(t6761.*(t8583-t11188))./4.0+(t9185.*(t8221-t11008))./4.0)-q1d.*(t5538+t5554+t5559+t5562-t6622+t7372+t7789+t7820+t7954+t8207+t8336+t8356+t8364+t8391+t8402+t8473-t8490-t8514+t8776+t8806+t9051+t9058+t9281+t9390+t9445+t9465-t9494-t9503-t9504-t9911-t9921+t10336+t10508+t11155+t11226+t11229+t11537+t11557-t11571+t11777-t11838+t11920-t12287-t12289+t12310-t12334+t12577+t13086+t13093+t13246+t13261+t13309-t13388-t13612+t13626+t13696-t13914-t13973-t13999+t14000-t14248-t14732+t14778+t14788-t14984+t15029+t15035-t15169+t15172-t15393+t15395+((t6853-t6864).*(t921+t1317-t5853))./4.0+(t11356.*(-t1476-t1540+t2091+t2165+t2579+t8.*(t260+t468+t570+t2298)))./4.0+(t13178.*(t3418-t3879+t4324-t5228+t5802+t9.*(t71-t391).*4.5305948634e-2+t17.*(t426-t581).*7.35522e-1))./4.0+(t13377.*(t1987-t2621+t3452-t4730+t5359+t9.*(t71-t391).*6.1597e-2+t17.*(t426-t581)))./4.0+(t5860.*(t6806-t8574))./4.0+(t6970.*(t6801-t8594))./4.0+(t8310.*(t6452-t8229))./4.0+(t9525.*(t6452-t8229))./4.0+(t8227.*(t6847-t9563))./4.0+(t9744.*(t6472-t9256))./4.0+(t8794.*(t263-t283-t310+t1265))./4.0+(t10942.*(-t3045-t3218+t3458+t3539+t3878+t8.*(t260+t468+t570+t2298).*1.666555))./4.0+t12.*(t881-t912).*(t2425-t2468).*8.07151e-1-t5.*t12.*t6447.*2.01382560198e-1-t5.*t12.*t7236.*6.23745e-2)+q7d.*t16204-q6d.*t16291+q5d.*t16335+q2d.*(t5572+t5576+t5657+t6529+t7405+t7415+t7864+t7865-t7874+t7896+t7917+t7918-t8279+t8307+t8423+t8444+t8946+t8954-t9082-t9403+t9422+t9690+t9693+t9876-t9888+t10114+t10123+t10245+t10304-t10308+t10970+t11046+t11077+t11435+t11624+t11627+t11664-t11670-t11743+t11943+t11956+t12030+t12091-t12258+t12312+t12473-t12633+t12760-t13122-t13540-t13550+t13560+t13571-t13762-t13912-t13921+t14005+t14007-t14158+t14416+t14418+t14711+t14713-t15113-t15114-t15308-t15310+(t5634.*(t6853-t6864))./4.0+(t5648.*(t6806-t8574))./4.0+(t8053.*(t6452-t8229))./4.0+(t7079.*(t6847-t9563))./4.0+(t8191.*(t6834-t9565))./4.0+(t9110.*(t6472-t9256))./4.0+(t10141.*(t6472-t9256))./4.0+t12.*t3243.*(t2425-t2468).*8.07151e-1+(t12.*t4860.*(t2425-t2468))./4.0)-phid.*(t5538+t5554+t5559+t5562-t6622+t7789+t8207+t8776+t8806+t9051+t9058+t9390+t9445-t10331+t10339+t10373+t10519-t10526+t10558+t10574+t10650+t10898+t10905+t10908+t11226+t11229-t11392-t11526-t11527+t11537+t11557+t11722-t11732+t11777+t12051+t12072-t12297-t12302+t12310+t12559+t12832+t13086+t13093+t13246+t13261+t13309+t13696-t13936-t14110-t14129+t14231-t14357-t14359+t14548+t14778+t14788+t15029+t15035-t15264+t15265-t15402+t15420-t15441+t15442+t15503-t15513-t15527-t15612-t15956+t15959-t15991+t15992+t15998+t16017+(t8794.*(t263+t1265-t7252-t5.*t12.*1.0442e-1))./4.0+(t13178.*(t3418-t3879+t4324+t11855+t9.*(t71-t391).*4.5305948634e-2+t17.*(t426-t581).*7.35522e-1+t9.*(t9166-t11658).*7.35522e-1))./4.0+(t12385.*(t6853-t6864))./4.0+(t11247.*(t6806-t8574))./4.0+(t12185.*(t6452-t8229))./4.0+(t11720.*(t6801-t8594))./4.0+(t12669.*(t6452-t8229))./4.0+(t14380.*(t6472-t9256))./4.0+(t14057.*(t6847-t9563))./4.0+(t8166.*(t1786+t2973-t7703-t5.*t12.*3.746479959e-1))./4.0+(t13377.*(t1987-t2621+t3452+t11654+t9.*(t71-t391).*6.1597e-2+t17.*(t426-t581)+t9.*(t9166-t11658)))./4.0+t12.*(t881-t912).*(t2425-t2468).*8.07151e-1),q3d.*(t6999+t7020-t7671+t7995+t8667+t9389-t9402-t9415-t9444-t9473-t9484+t9776+t9814+t10023+t10040+t10044+t10049-t10060+t10372+t10529+t10992+t11198+t11379+t11729+t11936+t11940+t12114+t12131+t12154-t12180+t12363-t12436+t12822-t13053-t13066-t13220-t13227-t13301-t13678+t13900+t13944+t13946+t14128+t14134+t14194+t14745-t14749+t15007-t15014+(t6430.*(t1748-t1821))./4.0+(t4064.*(t6806-t8574))./4.0+(t5646.*(t6452-t8229))./4.0+(t5234.*(t8589-t8592))./4.0+(t6884.*(t8219-t8226))./4.0+(t6302.*(t8582-t8586))./4.0+(t8640.*(t8219-t8226))./4.0+(t6761.*(t8583-t11188))./4.0+(t9185.*(t8221-t11008))./4.0)-phid.*t16453-q6d.*t16275-q1d.*t16411+q5d.*(t8846+t8856+t9151-t9348+t9369-t9396+t11122+t11125+t11303+t11314+t11427+t11445+t11598+t11610+t11880+t11894-t12825-t12840-t12922-t12932-t13174+t13287+t13295+t13366+t13378-t13555+t13962+t13965+t14139+t14145+t14595-t14596+t14780-t14787+t8.*t4024.*(t6452-t8229).*4.1663875e-1+t16.*t4021.*(t6452-t8229).*4.1663875e-1+t16.*t5696.*(t6452-t8229).*1.838805e-1+(t8.*t6046.*(t6452-t8229))./4.0+(t16.*t6069.*(t6452-t8229))./4.0+(t16.*t8477.*(t6452-t8229))./4.0)+q2d.*(t5297+t7666+t7719-t9159+t9267+t9274+t9418+t9421+t9542+t9551-t9573+t9651+t9886+t9889+t9988+t10000+t10002+t10262+t10479+t10891+t10902+t11093+t11279+t11443+t11446+t11620+t11771+t11776+t11790+t11851+t11931+t12439+t12445+t12639+t12649+t12982+t13139+t13141+t13190+t13253+t13260+t13552+t13575+t13583+t13592+t13596+t14002+t14232+t14234+t14487+t14489+t14956+t14958+t15189+t15193+(t7796.*(t9.*(t16.*(t30.*(t2425-t2468)+t68.*(t2425-t2468))+t8.*(t7.*(t4650+t34.*(t2425-t2468))+t47.*(t2425-t2468)))+t17.*(t4654+t15.*(t4650+t34.*(t2425-t2468)))))./4.0+(t5331.*(t30.*(t2425-t2468)+t68.*(t2425-t2468)))./4.0+(t6046.*(t16.*(t30.*(t2425-t2468)+t68.*(t2425-t2468))+t8.*(t7.*(t4650+t34.*(t2425-t2468))+t47.*(t2425-t2468))))./4.0+(t4024.*(t16.*(t30.*(t2425-t2468)+t68.*(t2425-t2468)).*1.666555+t8.*(t7.*(t4650+t34.*(t2425-t2468))+t47.*(t2425-t2468)).*1.666555))./4.0+t7.*(t7.*(t4650+t34.*(t2425-t2468)).*1.225946+t47.*(t2425-t2468).*1.225946).*8.639075e-2+t30.*(t2425-t2468).*9.5384188575e-2+t34.*(t2425-t2468).*1.8732399795e-1+t68.*(t2425-t2468).*9.5384188575e-2+(t3424.*(t30.*(t2425-t2468).*1.225946+t68.*(t2425-t2468).*1.225946))./4.0+t15.*(t4654+t15.*(t4650+t34.*(t2425-t2468))).*1.059103943995e-1+(t5443.*(t4654+t15.*(t4650+t34.*(t2425-t2468))))./4.0+t7.*(t7.*(t4650+t34.*(t2425-t2468))+t47.*(t2425-t2468)).*1.059103943995e-1+(t5329.*(t9.*(t16.*(t30.*(t2425-t2468)+t68.*(t2425-t2468))+t8.*(t7.*(t4650+t34.*(t2425-t2468))+t47.*(t2425-t2468))).*7.35522e-1+t17.*(t4654+t15.*(t4650+t34.*(t2425-t2468))).*7.35522e-1))./4.0)-q7d.*(t8886+t8907+t11429+t11431-t13130-t13291+t14545+t14550-t14627-t14633+t14697+t14700-t14831-t14837),q7d.*t16187-q3d.*t16335-q4d.*(t8846+t8856+t9151-t9348+t9369-t9396+t11122+t11125+t11303+t11314+t11427+t11445+t11598+t11610+t11880+t11894-t12825-t12840-t12922-t12932-t13174+t13287+t13295+t13366+t13378-t13555+t13962+t13965+t14139+t14145+t14595-t14596+t14780-t14787+t8.*t4024.*(t6452-t8229).*4.1663875e-1+t16.*t4021.*(t6452-t8229).*4.1663875e-1+t16.*t5696.*(t6452-t8229).*1.838805e-1+(t8.*t6046.*(t6452-t8229))./4.0+(t16.*t6069.*(t6452-t8229))./4.0+(t16.*t8477.*(t6452-t8229))./4.0)-q1d.*(t7328+t7338+t8774+t8795+t10202+t10562+t11039+t11047-t12176-t12438+t12441+t12499+t12504+t12595+t12596-t12703+t12771+t12783-t12852-t12972+t13074+t13505-t13584+t13693+t13958+t14215+t14448+t14451+t14494+t14498-t14736-t14992+t15150+t15312+((t6806-t8574).*(t921+t1317-t5853))./4.0+((t6452-t8229).*(t2810+t2988-t7937))./4.0+(t14213.*(t2740+t3849+t3968+t3972-t5255+t17.*(t260+t468+t570+t2298).*7.35522e-1))./4.0+(t13189.*(t3418-t3879+t4324-t5228+t5802+t9.*(t71-t391).*4.5305948634e-2+t17.*(t426-t581).*7.35522e-1))./4.0+(t13391.*(t1987-t2621+t3452-t4730+t5359+t9.*(t71-t391).*6.1597e-2+t17.*(t426-t581)))./4.0+(t12508.*(t1492+t2158+t2696-t4727))./4.0+(t12307.*(t3063+t3528+t3966-t5230))./4.0+(t10577.*(t495+t572+t1838+t2069+t2107))./4.0+(t10164.*(t2437+t2648+t3129+t3384+t3574))./4.0+(t5853.*(t6806-t8574))./4.0+(t6535.*(t6801-t8594))./4.0+(t7937.*(t6452-t8229))./4.0+(t8791.*(t6452-t8229))./4.0+(t14299.*(t824+t2543+t2699+t2707-t4767+t17.*(t260+t468+t570+t2298)))./4.0+t16.*t8227.*(t6452-t8229).*4.1663875e-1+(t16.*t9744.*(t6452-t8229))./4.0)-phid.*(t7328+t7338+t8774+t8795+t10202+t10562+t11039+t11047+t12499+t12504+t12595+t12596+t12771+t12783+t14211+t14214+t14269+t14328+t14335+t14342+t14344+t14437+t14448+t14451+t14490+t14494+t14498+t14614+t14615+t14751+t14988+t14991+t15105+t15110+t15207+t15208+t15224+t15392+t15413+t15415+t15416+t15532+t15942+t15943+t15981+t15986+t16004+t16007+t16023+t16027)-q6d.*(t10652+t11059+t11068+t12698+t12710+t12791+t12794+t12804+t12806+t12928+t12936+t13402-t13405+t13520-t13533+t14470+t14477+t14518+t14527+t16.*(t6452-t8229).*5.01208083475e-2+t16.*t3489.*(t6452-t8229).*1.838805e-1+(t16.*t5365.*(t6452-t8229))./4.0)+q2d.*(t5642+t5652+t7414+t7417+t9495+t9508+t10037+t10422+t10746+t10750+t10869+t10870+t11140+t11154-t11488+t11503+t11719+t11754-t11960+t11981+t12064+t12263+t12280+t12728+t12910+t12911+t13017+t13022-t13245-t13272-t13439-t13452-t13602-t14026+t14428+t14430+t14717+t14721+t14931-t14936+t15125-t15129+(t5634.*(t6806-t8574))./4.0+(t8050.*(t6452-t8229))./4.0+t16.*t7079.*(t6452-t8229).*4.1663875e-1+t8.*t7116.*(t6452-t8229).*4.1663875e-1+t16.*t8191.*(t6452-t8229).*1.838805e-1+(t8.*t9112.*(t6452-t8229))./4.0+(t16.*t9110.*(t6452-t8229))./4.0+(t16.*t10141.*(t6452-t8229))./4.0),q7d.*t16073+q4d.*t16275+q3d.*t16291-phid.*(-t10580+t10587+t11945+t12174-t12785-t12888-t14289-t14345+t15521+t15522+t15544+t15546+t15547+t15578+t15583+t15594+t15632+t15639+t15644+t15740+t15872+t15873+t15887+t15888+t15911+t15912+t15970+t15972+t9.*(t10403+t9.*(t10158+t16.*(t4542-t6448)).*7.35522e-1).*1.539925e-2+t8.*(t4542-t6448).*5.01208083475e-2+t16.*(t4542-t6448).*1.17633784675e-2+t9.*(t10174+t9.*(t10158+t16.*(t4542-t6448))).*1.13264871585e-2)-q1d.*(-t10580+t10587+t11945+t12174-t12785-t12888+t13485+t13494+t13662+t13685+t13690+t13830+t13831+t13870+t14072+t14081+t14093+t14243+t14245-t14289-t14345+t14393+t14575+t14579+t15059+t15062+t15204+t15206+t9.*(t10403+t9.*(t10158+t16.*(t4542-t6448)).*7.35522e-1).*1.539925e-2+t8.*(t4542-t6448).*5.01208083475e-2+t16.*(t4542-t6448).*1.17633784675e-2+t9.*(t10174+t9.*(t10158+t16.*(t4542-t6448))).*1.13264871585e-2)+q5d.*(t10652+t11059+t11068+t12698+t12710+t12791+t12794+t12804+t12806+t12928+t12936+t13402-t13405+t13520-t13533+t14470+t14477+t14518+t14527+t16.*(t6452-t8229).*5.01208083475e-2+t16.*t3489.*(t6452-t8229).*1.838805e-1+(t16.*t5365.*(t6452-t8229))./4.0)-q2d.*(t8952-t11170+t11723+t12027-t12690+t13257+t13258+t13361+t13443+t13450+t13547+t13549+t13581+t13820+t13917+t13922+t13929+t13938+t14183+t14256+t14259+t14875+t14876+t15011+t15015+t9.*(t9.*(t16.*(t30.*(t2425-t2468)+t68.*(t2425-t2468))+t8.*(t7.*(t4650+t34.*(t2425-t2468))+t47.*(t2425-t2468)))+t17.*(t4654+t15.*(t4650+t34.*(t2425-t2468)))).*1.13264871585e-2+t8.*(t30.*(t2425-t2468)+t68.*(t2425-t2468)).*5.01208083475e-2+t16.*(t30.*(t2425-t2468)+t68.*(t2425-t2468)).*1.17633784675e-2+t8.*(t7.*(t4650+t34.*(t2425-t2468))+t47.*(t2425-t2468)).*1.17633784675e-2+(t5365.*(t8315+t8.*(t30.*(t2425-t2468)+t68.*(t2425-t2468))))./4.0+t17.*(t8329+t17.*(t16.*(t30.*(t2425-t2468)+t68.*(t2425-t2468))+t8.*(t7.*(t4650+t34.*(t2425-t2468))+t47.*(t2425-t2468)))).*1.13264871585e-2+t9.*(t9.*(t16.*(t30.*(t2425-t2468)+t68.*(t2425-t2468))+t8.*(t7.*(t4650+t34.*(t2425-t2468))+t47.*(t2425-t2468))).*7.35522e-1+t17.*(t4654+t15.*(t4650+t34.*(t2425-t2468))).*7.35522e-1).*1.539925e-2),-q2d.*(t8350.*3.867742437e-3+t10735+t13315+t13529+t14946+t14951+t15092+t15097+t15102+t15107+t15300+t15306+t9.*(t16.*(t30.*(t2425-t2468)+t68.*(t2425-t2468))+t8.*(t7.*(t4650+t34.*(t2425-t2468))+t47.*(t2425-t2468))).*1.563719772e-3+t17.*(t4654+t15.*(t4650+t34.*(t2425-t2468))).*1.563719772e-3)-q6d.*t16073-q5d.*t16187-q3d.*t16204-phid.*(t10600+t10609+t12501+t12510-t13551-t13712+t16032+t16037+t16049+t16067+(t14299.*(t2497+t2680+t3516+t9.*(t210+t2107+t7423+t9121)+t17.*(t9166-t11658)))./4.0+(t14209.*(t3418-t3879+t4324+t11855+t9.*(t71-t391).*4.5305948634e-2+t17.*(t426-t581).*7.35522e-1+t9.*(t9166-t11658).*7.35522e-1))./4.0+(t14213.*(t3845+t3925+t4339+t9.*(t210+t2107+t7423+t9121).*7.35522e-1+t17.*(t9166-t11658).*7.35522e-1))./4.0+(t14297.*(t1987-t2621+t3452+t11654+t9.*(t71-t391).*6.1597e-2+t17.*(t426-t581)+t9.*(t9166-t11658)))./4.0)-q1d.*(t10600+t10609+t12501+t12510-t13551-t13712+t15181+t15182+t15289+t15293-t15358-t15476+(t14209.*(t3418-t3879+t4324-t5228+t5802+t9.*(t71-t391).*4.5305948634e-2+t17.*(t426-t581).*7.35522e-1))./4.0+(t14297.*(t1987-t2621+t3452-t4730+t5359+t9.*(t71-t391).*6.1597e-2+t17.*(t426-t581)))./4.0)+q4d.*(t8886+t8907+t11429+t11431-t13130-t13291+t14545+t14550-t14627-t14633+t14697+t14700-t14831-t14837),-q3d.*(-t5514-t5527-t5571-t5575-t6249+t6613+t7763+t8161+t8861+t8902+t9085+t9088+t9406+t9476+t10324+t10356+t10401+t10512+t10538+t10559+t10594+t10651+t10900+t10919+t10934+t11246+t11267+t11359+t11365+t11539+t11540+t11566+t11601+t11706+t11713+t11715+t11800+t12043+t12084+t12309+t12313+t12336+t12555+t12845+t13104+t13112+t13270+t13282+t13316+t13708+t13918+t13933+t14059+t14102+t14109+t14118+t14133+t14236+t14356+t14358+t14378+t14551+t14811+t14829+t15051+t15060+t15246+t15261+t15399+t15423+t15425+t15433+t15438+t15509+t15510+t15514+t15524+t15613+t15947+t15954+t15988+t15990+t16002+t16003+t16022+t16024)-q5d.*(t7280+t7283+t8889+t8899-t10176+t10541+t11053+t11058+t12514+t12526+t12607+t12615+t12787+t12801+t14199+t14202+t14263+t14316+t14319+t14331+t14336+t14432+t14465+t14471+t14484+t14514+t14524+t14593+t14594+t14746+t14978+t14983+t15086+t15091+t15198+t15203+t15213+t15382+t15404+t15405+t15408+t15528+t15929+t15930+t15977+t15979+t15995+t15996+t16015+t16016)-q4d.*(t5292+t5293+t7037+t7057+t9488+t9635+t10632+t10663+t10834+t10839+t11128+t11316-t12230+t12246+t12314-t12541+t12547-t12593-t12625+t12700+t12873+t12885+t13092+t13097+t13192-t13254-t13453-t13465+t13652+t13721+t13739-t13754-t13765+t13953+t14036+t14149+t14306+t14631+t14632+t14832+t14840-t15211-t15339-t15390-t15410-t15412-t15492-t15493-t15497+t15901+t15949+(t5598.*(t4540+t5.*(t2425-t2468)))./4.0+(t13380.*(t10158+t16.*(t4542-t6448)))./4.0+(t14541.*(t10403+t9.*(t10158+t16.*(t4542-t6448)).*7.35522e-1))./4.0+(t12689.*(t3418-t3879+t4324+t11855+t9.*(t71-t391).*4.5305948634e-2+t17.*(t426-t581).*7.35522e-1+t9.*(t9166-t11658).*7.35522e-1))./4.0+(t2701.*(t5122+t5.*(t2425-t2468).*3.587895))./4.0+(t9830.*(t5124-t6795))./4.0+(t9884.*(t5110-t6808))./4.0+(t10964.*(t4542-t6448))./4.0+(t10936.*(t1589-t2213-t4346+t4355+t9454+t11863+t2772.*(t71-t391)+t2775.*(t71-t391)))./4.0+(t12705.*(t3423+t3845+t3888+t3925+t4339+t9.*(t210+t2107+t7423+t9121).*7.35522e-1+t17.*(t9166-t11658).*7.35522e-1))./4.0+(t12867.*(t10384+t16.*(t4542-t6448).*1.666555))./4.0+(t11340.*(t249-t391.*(1.1e+1./1.25e+2)-t1912.*4.252e-3+t3505+t13496+t693.*(t71-t391)+t784.*(t71-t391)))./4.0+(t14918.*(t10174+t9.*(t10158+t16.*(t4542-t6448))))./4.0+(t12953.*(t2091+t2497+t2579+t2680+t3516+t9.*(t210+t2107+t7423+t9121)+t17.*(t9166-t11658)))./4.0+(t12945.*(t1987-t2621+t3452+t11654+t9.*(t71-t391).*6.1597e-2+t17.*(t426-t581)+t9.*(t9166-t11658)))./4.0+t15.*t12396.*(t4542-t6448).*3.064865e-1+(t15.*t13140.*(t4542-t6448))./4.0)-q7d.*t16296-q6d.*t16401-q2d.*t16469-q1d.*t16484+phid.*((t10966.*(t6460-t35.*(t2425-t2468)))./2.0-(t11907.*(t6460-t35.*(t2425-t2468)))./2.0+(t5062.*t5478)./2.0+(t4436.*t6338)./2.0+(t5450.*t5497)./2.0+(t5509.*t5681)./2.0+(t4436.*t7362)./2.0+(t7223.*t8156)./2.0+(t7226.*t8297)./2.0+(t6430.*t9218)./2.0+(t6430.*t10201)./2.0+(t8780.*t9828)./2.0+(t8794.*t9830)./2.0+(t8166.*t10964)./2.0-(t8779.*t10501)./2.0-(t10577.*t12385)./2.0-(t12503.*t14057)./2.0-(t12296.*t14380)./2.0+(t14213.*(t3418-t3879+t4324+t11855+t9.*(t71-t391).*4.5305948634e-2+t17.*(t426-t581).*7.35522e-1+t9.*(t9166-t11658).*7.35522e-1))./2.0-(t6646.*(t2425-t2468))./2.0-(t6447.*(t2720-t8734))./2.0-(t12396.*(t6806-t8574))./2.0-(t13140.*(t6452-t8229))./2.0+(t12564.*(t6801-t8594))./2.0+(t13416.*(t6452-t8229))./2.0+(t12296.*(t1589-t2213-t4346+t4355+t9454+t11863+t2772.*(t71-t391)+t2775.*(t71-t391)))./2.0+(t14209.*(t3423+t3845+t3888+t3925+t4339+t9.*(t210+t2107+t7423+t9121).*7.35522e-1+t17.*(t9166-t11658).*7.35522e-1))./2.0+(t12500.*(t249-t391.*(1.1e+1./1.25e+2)-t1912.*4.252e-3+t3505+t13496+t693.*(t71-t391)+t784.*(t71-t391)))./2.0+(t7236.*(-t3405+t4994+t5076))./2.0-(t10164.*(t2810+t2988-t12589))./2.0-(t12508.*(-t1476+t2165+t13876))./2.0-(t12307.*(-t3045+t3539+t14113))./2.0+(t14297.*(t2091+t2497+t2579+t2680+t3516+t9.*(t210+t2107+t7423+t9121)+t17.*(t9166-t11658)))./2.0+(t14299.*(t1987-t2621+t3452+t11654+t9.*(t71-t391).*6.1597e-2+t17.*(t426-t581)+t9.*(t9166-t11658)))./2.0-t4.*t5530.*(t2425-t2468).*3.23463e-1-t12.*t5535.*(t2425-t2468).*3.23463e-1-t12.*t6159.*(t2425-t2468).*1.614302-(t4.*t6481.*(t2425-t2468))./2.0-(t12.*t6483.*(t2425-t2468))./2.0-(t12.*t7389.*(t2425-t2468))./2.0),-q7d.*t16299+q6d.*t16406+q5d.*t16439+q4d.*t16452-q2d.*t16472+q1d.*t16479+q3d.*(-t5538-t5554-t5559-t5562-t6273-t6622-t7789+t8193+t8790+t8826+t9057+t9063+t9377+t9431-t10331+t10339+t10373+t10519-t10526+t10558+t10574+t10650+t10898+t10905+t10908+t11220+t11238-t11392-t11526-t11527+t11531+t11569+t11722-t11732+t11769+t12051+t12072-t12297-t12302+t12306+t12559+t12832+t13081+t13089+t13239+t13255+t13308+t13691-t13936-t14110-t14129+t14231-t14357-t14359+t14548+t14775+t14791+t15027+t15038-t15264+t15265-t15402+t15420-t15441+t15442+t15503-t15513-t15527-t15612-t15956+t15959-t15991+t15992+t15998+t16017+(t8794.*(t263+t1265-t7252-t5.*t12.*1.0442e-1))./4.0+(t13178.*(t3418-t3879+t4324+t11855+t9.*(t71-t391).*4.5305948634e-2+t17.*(t426-t581).*7.35522e-1+t9.*(t9166-t11658).*7.35522e-1))./4.0+(t12385.*(t6853-t6864))./4.0+(t11247.*(t6806-t8574))./4.0+(t12185.*(t6452-t8229))./4.0+(t11720.*(t6801-t8594))./4.0+(t12669.*(t6452-t8229))./4.0+(t14380.*(t6472-t9256))./4.0+(t14057.*(t6847-t9563))./4.0+(t8166.*(t1786+t2973-t7703-t5.*t12.*3.746479959e-1))./4.0+(t13377.*(t1987-t2621+t3452+t11654+t9.*(t71-t391).*6.1597e-2+t17.*(t426-t581)+t9.*(t9166-t11658)))./4.0)+phid.*((t9218.*(t4540+t5.*(t2425-t2468)))./2.0+(t10201.*(t4540+t5.*(t2425-t2468)))./2.0-(t5062.*t5497)./2.0+(t5450.*t5478)./2.0+(t4436.*t6646)./2.0-(t5515.*t5681)./2.0-(t8742.*t9830)./2.0-(t8077.*t10964)./2.0+(t10546.*t12385)./2.0-(t10554.*t12396)./2.0+(t10561.*t12564)./2.0-(t10153.*t13140)./2.0+(t10153.*t13416)./2.0+(t12487.*t14057)./2.0+(t12279.*t14380)./2.0+(t8156.*(t5117+t5.*(t2425-t2468).*3.228604))./2.0-((t10384+t16.*(t4542-t6448).*1.666555).*(-t1476+t2165+t13876))./2.0+(t8297.*(t5122+t5.*(t2425-t2468).*3.587895))./2.0+(t6338.*(t2425-t2468))./2.0+(t7362.*(t2425-t2468))./2.0+(t6431.*(t2720-t8734))./2.0+(t9828.*(t5124-t6795))./2.0+(t10966.*(t4542-t6448))./2.0-(t10501.*(t5110-t6808))./2.0-(t11907.*(t4542-t6448))./2.0-(t12279.*(t1589-t2213-t4346+t4355+t9454+t11863+t2772.*(t71-t391)+t2775.*(t71-t391)))./2.0-(t14185.*(t3423+t3845+t3888+t3925+t4339+t9.*(t210+t2107+t7423+t9121).*7.35522e-1+t17.*(t9166-t11658).*7.35522e-1))./2.0-(t12484.*(t249-t391.*(1.1e+1./1.25e+2)-t1912.*4.252e-3+t3505+t13496+t693.*(t71-t391)+t784.*(t71-t391)))./2.0-((t10158+t16.*(t4542-t6448)).*(-t3045+t3539+t14113))./2.0+((t10174+t9.*(t10158+t16.*(t4542-t6448))).*(t3418-t3879+t4324+t11855+t9.*(t71-t391).*4.5305948634e-2+t17.*(t426-t581).*7.35522e-1+t9.*(t9166-t11658).*7.35522e-1))./2.0+((t10403+t9.*(t10158+t16.*(t4542-t6448)).*7.35522e-1).*(t1987-t2621+t3452+t11654+t9.*(t71-t391).*6.1597e-2+t17.*(t426-t581)+t9.*(t9166-t11658)))./2.0-(t7224.*(-t3405+t4994+t5076))./2.0+(t10147.*(t2810+t2988-t12589))./2.0-(t14280.*(t2091+t2497+t2579+t2680+t3516+t9.*(t210+t2107+t7423+t9121)+t17.*(t9166-t11658)))./2.0+t4.*t4436.*t5530.*3.23463e-1+t12.*t4436.*t5535.*3.23463e-1+t12.*t4436.*t6159.*1.614302+(t4.*t4436.*t6481)./2.0+(t12.*t4436.*t6483)./2.0+(t12.*t4436.*t7389)./2.0),-q6d.*t16314+q5d.*t16352-q1d.*t16374-q4d.*t16372-q3d.*t16391-q2d.*t16393-q7d.*(t7842+t8174+t8286+t9182+t9210+t15012+t15215+t16106-t16107-t16109+t16110),t16375+t16481+t16483-q6d.*t16386-q5d.*t16432-q3d.*t16459-q2d.*t16473-q4d.*(t4831+t5358+t5377+t5506+t5611+t5616+t5767+t5926+t5959+t6083+t6861+t6962+t7012+t7072+t7107+t7324+t7380+t7648+t7675+t7709+t7725+t8074+t8098+t8629+t8815+t8961+t8990+t9054+t9089+t9864+t9975+t10146+t10701-t11268+t11269+t11391+t11393+t11458-t11461+t11463-t11474+t11575+t11583+t11655-t11657+t11895+t12016-t12317-t12454-t12597+t12609-t12828+t12844+t13221+t13420+t13568+t13573-t13633+t13637+t13720+t13728-t13845+t13848+t13864+t14078+t14136+t14188-t14296+t14298-t14347+t14348-t14847-t14849-t14878-t14880+t15161+t15162+t15314+t15323-t15605-t15606+t15849+t15850+(t6190.*(-t1053-t3327+t5081.*1.225946+t7731+t15.*t223.*1.4653732538e-2))./4.0+(t14541.*(t3418-t3879+t4324-t5228+t5802+t9.*(t71-t391).*4.5305948634e-2+t17.*(t426-t581).*7.35522e-1))./4.0+(t9187.*(t3418-t3879+t4324+t11855+t9.*(t71-t391).*4.5305948634e-2+t17.*(t426-t581).*7.35522e-1+t9.*(t9166-t11658).*7.35522e-1))./4.0+(t14918.*(t1987-t2621+t3452-t4730+t5359+t9.*(t71-t391).*6.1597e-2+t17.*(t426-t581)))./4.0+(t13273.*(t1589-t2213+t3195-t4346+t4355+t4748.*7.35522e-1+t2772.*(t71-t391)+t2775.*(t71-t391)))./4.0+(t10501.*(t985+t3399-t13.*t42.*1.01140545e-1-t7.*t223.*5.034347249e-2))./4.0+(t8433.*(t1589-t2213-t4346+t4355+t9454+t11863+t2772.*(t71-t391)+t2775.*(t71-t391)))./4.0+(t13974.*(t249-t391.*(1.1e+1./1.25e+2)-t1912.*4.252e-3+t3505+t5357+t693.*(t71-t391)+t784.*(t71-t391)))./4.0+(t10096.*(t249-t391.*(1.1e+1./1.25e+2)-t1912.*4.252e-3+t3505+t13496+t693.*(t71-t391)+t784.*(t71-t391)))./4.0+(t10753.*(t1987-t2621+t3452+t11654+t9.*(t71-t391).*6.1597e-2+t17.*(t426-t581)+t9.*(t9166-t11658)))./4.0)-q7d.*(t7842+t8174+t8286+t9182+t9210+t11968+t12456-t13211+t13214+t15013+t15216+t15822+t15824+t15826+t15829+t15860+t15862+t15864+t15865+t9.*(t8963+t7.*(t5026+t5.*(t2959-t2967))).*3.867742437e-3+t17.*(t8963+t7.*(t5026+t5.*(t2959-t2967))).*1.563719772e-3),t16394+t16468-t16471+q4d.*(t2261+t2304+t2384+t3146+t3288+t3303+t3305+t3351+t3740+t4007+t4025+t4048+t4164+t4320+t4571+t4863+t4946+t4985+t5104+t5114+t5279+t5328+t5355+t5375+t5406+t5629+t5632+t5645+t5747+t5771+t5790+t5808+t5825+t5907+t5980+t6061+t6136+t6292+t6454+t6571+t6648+t6666+t6668+t6700+t6760+t6829+t6891+t6895+t6922+t7006+t7013+t7091+t7110+t7291+t7340+t7554+t7564+t7566+t7626+t7664+t7825+t7850+t7986+t8001+t8122+t8346+t8375+t8385+t8598+t8639+t8649+t8684+t8718+t8737+t8827+t8959+t9105+t10453+t10686-t10825-t10829-t10978+t10993-t11184+t11191+t11263+t11287-t11408-t11418+t11513-t11868+t11980+t12150+t12196+t12202+t12209-t12308-t12319-t12380-t12390-t12406+t12759+t12934+t13157-t13262-t13275+t13449+t13471-t13579-t13588+t13670+t13684+t13978+t14042-t14159+t14166+t14221-t14225+t14226+t14262-t14635-t14682-t14726-t14727-t14762-t14764+t15126+t15130+t15176+t15180+t15488+t15489+t15494+t15495+(t7987.*(t3418-t3879+t4324+t11855+t9.*(t71-t391).*4.5305948634e-2+t17.*(t426-t581).*7.35522e-1+t9.*(t9166-t11658).*7.35522e-1))./4.0+(t7130.*(t1589-t2213-t4346+t4355+t9454+t11863+t2772.*(t71-t391)+t2775.*(t71-t391)))./4.0+(t7982.*(t3423+t3845+t3888+t3925+t4339+t9.*(t210+t2107+t7423+t9121).*7.35522e-1+t17.*(t9166-t11658).*7.35522e-1))./4.0+(t9310.*(t249-t391.*(1.1e+1./1.25e+2)-t1912.*4.252e-3+t3505+t13496+t693.*(t71-t391)+t784.*(t71-t391)))./4.0+(t9887.*(t2091+t2497+t2579+t2680+t3516+t9.*(t210+t2107+t7423+t9121)+t17.*(t9166-t11658)))./4.0+(t9896.*(t1987-t2621+t3452+t11654+t9.*(t71-t391).*6.1597e-2+t17.*(t426-t581)+t9.*(t9166-t11658)))./4.0)+q6d.*t16395+q5d.*t16441+q1d.*t16473+q3d.*t16476-q7d.*(t4484+t4576+t4580+t4749+t4773+t4786+t5002+t5030-t6965+t7258-t7472-t7744-t8540-t8593+t9003+t10285+t10292-t11218-t11933+t12219+t12221+t14924+t15122+t15777+t15779+t15794+t15796+(t6276.*(t1918+t9.*(t71-t391)))./4.0+(t8622.*(t395+t9.*(t48-t349)))./4.0+(t7949.*(t3418-t3879+t4324+t11855+t9.*(t71-t391).*4.5305948634e-2+t17.*(t426-t581).*7.35522e-1+t9.*(t9166-t11658).*7.35522e-1))./4.0+(t1907.*(t1912.*(-1.0027e-2)+t2709+t3492+t751.*(t71-t391)))./4.0+(t7940.*(t3423+t3845+t3888+t3925+t4339+t9.*(t210+t2107+t7423+t9121).*7.35522e-1+t17.*(t9166-t11658).*7.35522e-1))./4.0+(t9362.*(t2091+t2497+t2579+t2680+t3516+t9.*(t210+t2107+t7423+t9121)+t17.*(t9166-t11658)))./4.0+(t9361.*(t1987-t2621+t3452+t11654+t9.*(t71-t391).*6.1597e-2+t17.*(t426-t581)+t9.*(t9166-t11658)))./4.0),t16392+t16462+t16466-q7d.*t16269-q6d.*t16380+q5d.*t16429+q4d.*t16447+q1d.*t16459-q2d.*t16476,t16373-t16454-q2d.*(t2261+t2304+t2384+t3146+t3288+t3303+t3305+t3351+t3740+t4007+t4025+t4048+t4164+t4320+t4571+t4863+t4946+t4985+t5104+t5114+t5279+t5328+t5355+t5375+t5406+t5629+t5632+t5645+t5747+t5771+t5790+t5808+t5825+t5907+t5980+t6061+t6136+t6292+t6454+t6571+t6648+t6666+t6668+t6700+t6760+t6829+t6891+t6895+t6922+t7006+t7013+t7091+t7110+t7291+t7340+t7554+t7564+t7566+t7626+t7664+t7825+t7850+t7986+t8001+t8122+t8346+t8375+t8385+t8598+t8639+t8649+t8684+t8718+t8737+t8827+t8959+t9105+t10453+t10686-t10825-t10829-t10978+t10993-t11184+t11191+t11263+t11287-t11408-t11418+t11513-t11868+t11980+t12150+t12196+t12202+t12209-t12308-t12319-t12380-t12390-t12406+t12759+t12934+t13157-t13262-t13275+t13449+t13471-t13579-t13588+t13670+t13684+t13978+t14042-t14159+t14166+t14221-t14225+t14226+t14262-t14635-t14682-t14726-t14727-t14762-t14764+t15126+t15130+t15176+t15180+t15488+t15489+t15494+t15495+(t7987.*(t3418-t3879+t4324+t11855+t9.*(t71-t391).*4.5305948634e-2+t17.*(t426-t581).*7.35522e-1+t9.*(t9166-t11658).*7.35522e-1))./4.0+(t7130.*(t1589-t2213-t4346+t4355+t9454+t11863+t2772.*(t71-t391)+t2775.*(t71-t391)))./4.0+(t7982.*(t3423+t3845+t3888+t3925+t4339+t9.*(t210+t2107+t7423+t9121).*7.35522e-1+t17.*(t9166-t11658).*7.35522e-1))./4.0+(t9310.*(t249-t391.*(1.1e+1./1.25e+2)-t1912.*4.252e-3+t3505+t13496+t693.*(t71-t391)+t784.*(t71-t391)))./4.0+(t9887.*(t2091+t2497+t2579+t2680+t3516+t9.*(t210+t2107+t7423+t9121)+t17.*(t9166-t11658)))./4.0+(t9896.*(t1987-t2621+t3452+t11654+t9.*(t71-t391).*6.1597e-2+t17.*(t426-t581)+t9.*(t9166-t11658)))./4.0)-q7d.*t16263-q6d.*t16376+q5d.*t16426-q3d.*t16447+xd.*(t5283+t5287+t7042+t7055+t9480+t9626+t10643+t10682+t10838+t10843+t11138+t11325-t12230+t12246+t12314-t12541+t12547-t12593-t12625+t12700+t12876+t12880+t13094+t13095+t13193-t13254-t13453-t13465+t13655+t13721+t13739-t13754-t13765+t13953+t14036+t14149+t14306+t14630+t14634+t14834+t14836-t15211-t15339-t15390-t15410-t15412-t15492-t15493-t15497+t15901+t15949+(t5598.*(t4540+t5.*(t2425-t2468)))./4.0+(t13380.*(t10158+t16.*(t4542-t6448)))./4.0+(t14541.*(t10403+t9.*(t10158+t16.*(t4542-t6448)).*7.35522e-1))./4.0+(t12689.*(t3418-t3879+t4324+t11855+t9.*(t71-t391).*4.5305948634e-2+t17.*(t426-t581).*7.35522e-1+t9.*(t9166-t11658).*7.35522e-1))./4.0+(t2701.*(t5122+t5.*(t2425-t2468).*3.587895))./4.0+(t9830.*(t5124-t6795))./4.0+(t9884.*(t5110-t6808))./4.0+(t10964.*(t4542-t6448))./4.0+(t10936.*(t1589-t2213-t4346+t4355+t9454+t11863+t2772.*(t71-t391)+t2775.*(t71-t391)))./4.0+(t12705.*(t3423+t3845+t3888+t3925+t4339+t9.*(t210+t2107+t7423+t9121).*7.35522e-1+t17.*(t9166-t11658).*7.35522e-1))./4.0+(t12867.*(t10384+t16.*(t4542-t6448).*1.666555))./4.0+(t11340.*(t249-t391.*(1.1e+1./1.25e+2)-t1912.*4.252e-3+t3505+t13496+t693.*(t71-t391)+t784.*(t71-t391)))./4.0+(t14918.*(t10174+t9.*(t10158+t16.*(t4542-t6448))))./4.0+(t12953.*(t2091+t2497+t2579+t2680+t3516+t9.*(t210+t2107+t7423+t9121)+t17.*(t9166-t11658)))./4.0+(t12945.*(t1987-t2621+t3452+t11654+t9.*(t71-t391).*6.1597e-2+t17.*(t426-t581)+t9.*(t9166-t11658)))./4.0+t15.*t12396.*(t4542-t6448).*3.064865e-1+(t15.*t13140.*(t4542-t6448))./4.0)+q1d.*(t4831+t5358+t5377+t5506+t5611+t5616+t5767+t5926+t5959+t6083+t6861+t6962+t7012+t7072+t7107+t7324+t7380+t7648+t7675+t7709+t7725+t8074+t8098+t8629+t8815+t8961+t8990+t9054+t9089+t9864+t9975+t10146+t10701-t11268+t11269+t11391+t11393+t11458-t11461+t11463-t11474+t11575+t11583+t11655-t11657+t11895+t12016-t12317-t12454-t12597+t12609-t12828+t12844+t13221+t13420+t13568+t13573-t13633+t13637+t13720+t13728-t13845+t13848+t13864+t14078+t14136+t14188-t14296+t14298-t14347+t14348-t14847-t14849-t14878-t14880+t15161+t15162+t15314+t15323-t15605-t15606+t15849+t15850+(t6190.*(-t1053-t3327+t5081.*1.225946+t7731+t15.*t223.*1.4653732538e-2))./4.0+(t14541.*(t3418-t3879+t4324-t5228+t5802+t9.*(t71-t391).*4.5305948634e-2+t17.*(t426-t581).*7.35522e-1))./4.0+(t9187.*(t3418-t3879+t4324+t11855+t9.*(t71-t391).*4.5305948634e-2+t17.*(t426-t581).*7.35522e-1+t9.*(t9166-t11658).*7.35522e-1))./4.0+(t14918.*(t1987-t2621+t3452-t4730+t5359+t9.*(t71-t391).*6.1597e-2+t17.*(t426-t581)))./4.0+(t13273.*(t1589-t2213+t3195-t4346+t4355+t4748.*7.35522e-1+t2772.*(t71-t391)+t2775.*(t71-t391)))./4.0+(t10501.*(t985+t3399-t13.*t42.*1.01140545e-1-t7.*t223.*5.034347249e-2))./4.0+(t8433.*(t1589-t2213-t4346+t4355+t9454+t11863+t2772.*(t71-t391)+t2775.*(t71-t391)))./4.0+(t13974.*(t249-t391.*(1.1e+1./1.25e+2)-t1912.*4.252e-3+t3505+t5357+t693.*(t71-t391)+t784.*(t71-t391)))./4.0+(t10096.*(t249-t391.*(1.1e+1./1.25e+2)-t1912.*4.252e-3+t3505+t13496+t693.*(t71-t391)+t784.*(t71-t391)))./4.0+(t10753.*(t1987-t2621+t3452+t11654+t9.*(t71-t391).*6.1597e-2+t17.*(t426-t581)+t9.*(t9166-t11658)))./4.0),-t16353+t16438-q4d.*t16426-q3d.*t16429+q1d.*t16432-q2d.*t16441-q7d.*(-t4652-t4658+t4757+t4840+t5267+t5296+t5773+t5803+t7148+t7195+t7207+t8626+t8682+t8881+t9257+t12008+t12014+t12018+t14549+t14869+t15554+t15558+t15597+t15601+t15608+t15610+t15669+t15670+t8.*t11672.*3.867742437e-3+t2963.*(t71-t391)+t3167.*(t71-t391)+t4080.*(t71-t391)+t4130.*(t71-t391))+q6d.*(-t4238+t4295-t4456+t4713+t4744+t4783+t4797+t4947+t5325+t5330+t5336+t5390+t5749+t5814+t6360+t6396+t7007+t7031+t7103+t7491+t7572+t7583+t8090+t8624+t8648+t8676+t8721+t11997+t13108-t13433+t13688-t13853+t14033+t14034+t14196+t14197+t14200+t14205+t14255+t14351+t14460+t14461+t14479+t14483+t14554+t14591+t14592+t14871-t14895-t15140+t15619+t15620+t15689+t15690+(t9.*(t578.*4.28e-4+t2566-t2597+t905.*(t71-t391)+t1021.*(t71-t391)))./4.0+t8.*(t210+t2107+t7423+t9121).*1.17633784675e-2+t17.*(-t2550+t2696+t2698+t11659+t8.*t11672+t147.*(t71-t391)).*1.13264871585e-2+t17.*(-t3823+t3970+t11861+t8.*t11864+t972.*(t71-t391)+t2777.*(t71-t391)).*1.539925e-2+t8.*(t71-t391).*5.187945860934245e-5+t16.*(t71-t391).*4.67845486573025e-5+(t2522.*(t689-t740))./4.0+(t16.*t3286.*(t71-t391))./4.0)+xd.*(t7290+t7292+t8876+t8913+t10169+t10541+t11057+t11063+t12519+t12522+t12610+t12611+t12793+t12805+t14199+t14202+t14263+t14316+t14319+t14331+t14336+t14432+t14466+t14469+t14484+t14516+t14520+t14593+t14594+t14746+t14978+t14983+t15086+t15091+t15198+t15203+t15213+t15382+t15404+t15405+t15408+t15528+t15929+t15930+t15977+t15979+t15995+t15996+t16015+t16016),t16315+t16405+xd.*(-t8850-t8864-t10622+t10627+t11928+t12142-t12808-t12904-t14301-t14305-t14353-t14354+t15516+t15519+t15537+t15539+t15543+t15568+t15569+t15587+t15625+t15626+t15634+t15736+t15867+t15870+t15882+t15885+t15909+t15910+t15967+t15969)+q4d.*t16376+q3d.*t16380+q1d.*t16386-q2d.*t16395-q5d.*(-t4238+t4295-t4456+t4713+t4744+t4783+t4797+t4947+t5325+t5330+t5336+t5390+t5749+t5814+t6360+t6396+t7007+t7031+t7103+t7491+t7572+t7583+t8090+t8624+t8648+t8676+t8721+t11997+t13108-t13433+t13688-t13853+t14033+t14034+t14196+t14197+t14200+t14205+t14255+t14351+t14460+t14461+t14479+t14483+t14554+t14591+t14592+t14871-t14895-t15140+t15619+t15620+t15689+t15690+(t9.*(t578.*4.28e-4+t2566-t2597+t905.*(t71-t391)+t1021.*(t71-t391)))./4.0+t8.*(t210+t2107+t7423+t9121).*1.17633784675e-2+t17.*(-t2550+t2696+t2698+t11659+t8.*t11672+t147.*(t71-t391)).*1.13264871585e-2+t17.*(-t3823+t3970+t11861+t8.*t11864+t972.*(t71-t391)+t2777.*(t71-t391)).*1.539925e-2+t8.*(t71-t391).*5.187945860934245e-5+t16.*(t71-t391).*4.67845486573025e-5+(t2522.*(t689-t740))./4.0+(t16.*t3286.*(t71-t391))./4.0)+q7d.*(-t4446-t4631-t4668-t4758+t4796+t5014+t5186+t5242+t5249+t5260+t7125+t7190+t8614+t8666+t9074+t9268-t13711+t13715+t14543+t14862+t15500+t15501+t15556+t15560+t15562+t15563+t15662+t15665+t9.*(t348-t525).*8.36241330891889e-4),t16295+t16301+q4d.*t16263+q3d.*t16269+q5d.*(-t4652-t4658+t4757+t4840+t5267+t5296+t5773+t5803+t7148+t7195+t7207+t8626+t8682+t8881+t9257+t12008+t12014+t12018+t14549+t14869+t15554+t15558+t15597+t15601+t15608+t15610+t15669+t15670+t8.*t11672.*3.867742437e-3+t2963.*(t71-t391)+t3167.*(t71-t391)+t4080.*(t71-t391)+t4130.*(t71-t391))-q6d.*(-t4446-t4631-t4668-t4758+t4796+t5014+t5186+t5242+t5249+t5260+t7125+t7190+t8614+t8666+t9074+t9268-t13711+t13715+t14543+t14862+t15500+t15501+t15556+t15560+t15562+t15563+t15662+t15665+t9.*(t348-t525).*8.36241330891889e-4)+q1d.*(t7842+t8174+t8286+t9182+t9210+t11968+t12456-t13211+t13214+t15013+t15216+t15822+t15824+t15826+t15829+t15860+t15862+t15864+t15865+t9.*(t8963+t7.*(t5026+t5.*(t2959-t2967))).*3.867742437e-3+t17.*(t8963+t7.*(t5026+t5.*(t2959-t2967))).*1.563719772e-3)+q2d.*(t4484+t4576+t4580+t4749+t4773+t4786+t5002+t5030-t6965+t7258-t7472-t7744-t8540-t8593+t9003+t10285+t10292-t11218-t11933+t12219+t12221+t14924+t15122+t15777+t15779+t15794+t15796+(t6276.*(t1918+t9.*(t71-t391)))./4.0+(t8622.*(t395+t9.*(t48-t349)))./4.0+(t7949.*(t3418-t3879+t4324+t11855+t9.*(t71-t391).*4.5305948634e-2+t17.*(t426-t581).*7.35522e-1+t9.*(t9166-t11658).*7.35522e-1))./4.0+(t1907.*(t1912.*(-1.0027e-2)+t2709+t3492+t751.*(t71-t391)))./4.0+(t7940.*(t3423+t3845+t3888+t3925+t4339+t9.*(t210+t2107+t7423+t9121).*7.35522e-1+t17.*(t9166-t11658).*7.35522e-1))./4.0+(t9362.*(t2091+t2497+t2579+t2680+t3516+t9.*(t210+t2107+t7423+t9121)+t17.*(t9166-t11658)))./4.0+(t9361.*(t1987-t2621+t3452+t11654+t9.*(t71-t391).*6.1597e-2+t17.*(t426-t581)+t9.*(t9166-t11658)))./4.0)+phid.*(t7842+t8174+t8286+t9182+t9210+t15012+t15215+t16106-t16107-t16109+t16110),-q5d.*(t7280+t7283+t8889+t8899-t10176+t10541+t11053+t11058+t11833+t11839+t12036+t12141+t12153+t12179+t12192+t12420+t12423+t12429+t12492+t12514+t12526+t12607+t12615+t12676+t12677+t12787+t12801+t12835+t12947+t12951+t13058+t13477+t13488+t13574+t13671+t13683+t13940+t14207+t14465+t14471+t14514+t14524+t14728+t14729+t14979+t14982+t15133+t15135+t15288+t15290)-phid.*t16484-q7d.*t16221-q6d.*t16319-q3d.*t16416-q2d.*t16421+q4d.*(-t5292-t5293-t7037-t7057+t8240+t8799+t9480+t9620+t9626+t9636+t9708+t9729+t9780+t10012+t10046+t10138+t10325+t10326+t10448+t10631+t10643+t10668+t10682+t10838+t10843+t10983+t11138+t11241+t11325+t11692+t11701+t11873+t11885+t12122+t12190+t12231+t12255+t12608+t12876+t12880+t12966+t12971+t13094+t13095+t13193+t13348+t13359+t13373+t13425+t13432+t13655+t13727+t13733+t13850+t13969+t14140+t14511+t14512+t14630+t14634+t14766+t14774+t14834+t14836+t15139+t15144+t15377+t15379)+q1d.*(t2422.*1.92614005e-2-t2425.*1.0343993404e-2+t2468.*1.0343993404e-2+t2471.*1.92614005e-2+(t6767.*(t6460-t35.*(t2425-t2468)))./2.0-(t8711.*(t6460-t35.*(t2425-t2468)))./2.0-(t12508.*(-t1476-t1540+t2091+t2165+t2579+t8.*(t260+t468+t570+t2298)))./2.0-(t2087.*t5509)./2.0-(t4356.*t4436)./2.0+(t3350.*t7223)./2.0-(t3405.*t7236)./2.0+(t4916.*t6430)./2.0-(t4936.*t6447)./2.0+(t6430.*t6713)./2.0+(t4557.*t8794)./2.0+(t4611.*t8780)./2.0+(t6750.*t8166)./2.0-(t6190.*t8779)./2.0-(t8227.*t12503)./2.0-(t9744.*t12296)./2.0+(t10149.*t14297)./2.0+(t11470.*t14209)./2.0+(t14213.*(t3418-t3879+t4324-t5228+t5802+t9.*(t71-t391).*4.5305948634e-2+t17.*(t426-t581).*7.35522e-1))./2.0+(t14299.*(t1987-t2621+t3452-t4730+t5359+t9.*(t71-t391).*6.1597e-2+t17.*(t426-t581)))./2.0+(t12296.*(t1589-t2213+t3195-t4346+t4355+t4748.*7.35522e-1+t2772.*(t71-t391)+t2775.*(t71-t391)))./2.0-t18.*(t2425-t2468).*2.26100637e-3-t24.*(t2425-t2468).*2.26100637e-3-(t7039.*(t6806-t8574))./2.0+(t7822.*(t6801-t8594))./2.0-(t9236.*(t6452-t8229))./2.0+(t9967.*(t6452-t8229))./2.0+(t12500.*(t249-t391.*(1.1e+1./1.25e+2)-t1912.*4.252e-3+t3505+t5357+t693.*(t71-t391)+t784.*(t71-t391)))./2.0+(t7226.*(t85+t338+t362+t375+t408+t5.*t12.*(7.9e+1./2.5e+2)))./2.0-(t12307.*(-t3045-t3218+t3458+t3539+t3878+t8.*(t260+t468+t570+t2298).*1.666555))./2.0-(t10577.*(t921+t1317-t5853))./2.0-(t10164.*(t2810+t2988-t7937))./2.0-t12.*t3318.*(t2425-t2468).*1.614302-(t12.*t4908.*(t2425-t2468))./2.0),q3d.*(-t5538-t5554-t5559-t5562-t6273-t6622-t7385-t7398-t7789-t7837-t7839-t7964-t8207+t8336+t8356+t8364+t8391+t8402+t8473-t8490-t8514+t8790+t8826+t9057+t9063+t9281+t9377+t9431+t9465-t9494-t9503-t9504-t9911-t9921+t10336+t10508+t11155+t11220+t11238+t11531+t11569-t11571+t11769-t11838+t11920-t12287-t12289+t12306-t12334+t12577+t13081+t13089+t13239+t13255+t13308-t13388-t13612+t13626+t13691-t13914-t13973-t13999+t14000-t14248-t14732+t14775+t14791-t14984+t15027+t15038-t15169+t15172-t15393+t15395+((t6853-t6864).*(t921+t1317-t5853))./4.0+(t11356.*(-t1476-t1540+t2091+t2165+t2579+t8.*(t260+t468+t570+t2298)))./4.0+(t13178.*(t3418-t3879+t4324-t5228+t5802+t9.*(t71-t391).*4.5305948634e-2+t17.*(t426-t581).*7.35522e-1))./4.0+(t13377.*(t1987-t2621+t3452-t4730+t5359+t9.*(t71-t391).*6.1597e-2+t17.*(t426-t581)))./4.0+(t5860.*(t6806-t8574))./4.0+(t6970.*(t6801-t8594))./4.0+(t8310.*(t6452-t8229))./4.0+(t9525.*(t6452-t8229))./4.0+(t8227.*(t6847-t9563))./4.0+(t9744.*(t6472-t9256))./4.0+(t8794.*(t263-t283-t310+t1265))./4.0+(t10942.*(-t3045-t3218+t3458+t3539+t3878+t8.*(t260+t468+t570+t2298).*1.666555))./4.0)+phid.*t16479-q7d.*t16225+q6d.*t16324+q4d.*t16410-q2d.*t16422+q5d.*(t7309+t7314+t8781+t8789+t10202+t10562+t11032+t11043-t12176-t12438+t12441+t12496+t12509+t12592+t12598-t12703+t12766+t12779-t12852-t12972+t13074+t13505-t13584+t13693+t13958+t14215+t14447+t14453+t14492+t14501-t14736-t14992+t15150+t15312+((t6806-t8574).*(t921+t1317-t5853))./4.0+((t6452-t8229).*(t2810+t2988-t7937))./4.0+(t14213.*(t2740+t3849+t3968+t3972-t5255+t17.*(t260+t468+t570+t2298).*7.35522e-1))./4.0+(t13189.*(t3418-t3879+t4324-t5228+t5802+t9.*(t71-t391).*4.5305948634e-2+t17.*(t426-t581).*7.35522e-1))./4.0+(t13391.*(t1987-t2621+t3452-t4730+t5359+t9.*(t71-t391).*6.1597e-2+t17.*(t426-t581)))./4.0+(t12508.*(t1492+t2158+t2696-t4727))./4.0+(t12307.*(t3063+t3528+t3966-t5230))./4.0+(t10577.*(t495+t572+t1838+t2069+t2107))./4.0+(t10164.*(t2437+t2648+t3129+t3384+t3574))./4.0+(t5853.*(t6806-t8574))./4.0+(t6535.*(t6801-t8594))./4.0+(t7937.*(t6452-t8229))./4.0+(t8791.*(t6452-t8229))./4.0+(t14299.*(t824+t2543+t2699+t2707-t4767+t17.*(t260+t468+t570+t2298)))./4.0+t16.*t8227.*(t6452-t8229).*4.1663875e-1+(t16.*t9744.*(t6452-t8229))./4.0)+q1d.*(t2422.*1.0343993404e-2+t2425.*1.92614005e-2-t2468.*1.92614005e-2+t2471.*1.0343993404e-2+(t4916.*(t4540+t5.*(t2425-t2468)))./2.0+(t6713.*(t4540+t5.*(t2425-t2468)))./2.0+((t10403+t9.*(t10158+t16.*(t4542-t6448)).*7.35522e-1).*(t1987-t2621+t3452-t4730+t5359+t9.*(t71-t391).*6.1597e-2+t17.*(t426-t581)))./2.0+t18.*t4436.*2.26100637e-3+t24.*t4436.*2.26100637e-3+(t2087.*t5515)./2.0+(t3405.*t7224)./2.0+(t4936.*t6431)./2.0-(t4557.*t8742)./2.0-(t6750.*t8077)./2.0-(t7039.*t10554)./2.0+(t7822.*t10561)./2.0-(t9236.*t10153)./2.0+(t9967.*t10153)./2.0+(t8227.*t12487)./2.0+(t9744.*t12279)./2.0-(t10149.*t14280)./2.0-(t11470.*t14185)./2.0+(t3350.*(t5117+t5.*(t2425-t2468).*3.228604))./2.0-(t12279.*(t1589-t2213+t3195-t4346+t4355+t4748.*7.35522e-1+t2772.*(t71-t391)+t2775.*(t71-t391)))./2.0-(t4356.*(t2425-t2468))./2.0+(t4611.*(t5124-t6795))./2.0+(t6767.*(t4542-t6448))./2.0-(t6190.*(t5110-t6808))./2.0-(t8711.*(t4542-t6448))./2.0-((t10384+t16.*(t4542-t6448).*1.666555).*(-t1476-t1540+t2091+t2165+t2579+t8.*(t260+t468+t570+t2298)))./2.0-((t10158+t16.*(t4542-t6448)).*(-t3045-t3218+t3458+t3539+t3878+t8.*(t260+t468+t570+t2298).*1.666555))./2.0-(t12484.*(t249-t391.*(1.1e+1./1.25e+2)-t1912.*4.252e-3+t3505+t5357+t693.*(t71-t391)+t784.*(t71-t391)))./2.0+((t10174+t9.*(t10158+t16.*(t4542-t6448))).*(t3418-t3879+t4324-t5228+t5802+t9.*(t71-t391).*4.5305948634e-2+t17.*(t426-t581).*7.35522e-1))./2.0+((t5122+t5.*(t2425-t2468).*3.587895).*(t85+t338+t362+t375+t408+t5.*t12.*(7.9e+1./2.5e+2)))./2.0+(t10546.*(t921+t1317-t5853))./2.0+(t10147.*(t2810+t2988-t7937))./2.0+t12.*t3318.*t4436.*1.614302+(t12.*t4436.*t4908)./2.0),-t16375-t16483+q3d.*(t3604-t3629+t3748-t4422-t4525+t4637+t4793+t4957-t5288-t5896+t5900+t5902+t5922+t5934+t5937+t6109+t6110-t6260+t6343+t6393-t6948+t7018-t7050-t7627+t7659+t7776-t7971+t7997+t8086+t8455+t8458+t8480+t8710+t8716-t8777-t8934-t9042+t9070-t9126-t9139+t9366-t9380-t9384+t9393-t9496-t9583-t9602+t9650+t9661-t9940+t9965+t9974-t10143+t10210+t10215+t10406+t10416-t10537+t11110+t11116+t11496+t11497+t11977+t11986+t12028+t12034+t12173+t12188+t12354+t12565+t12687+t12730-t13199+t13215-t13307+t13311-t13664+t13689+t13736+t13737-t13813+t13837-t13885-t13886+t13930+t13939+t13991-t14171-t14174+t14175-t14417-t14420-t14960-t14961+t14966+t14967+t15294+t15307+t15454+t15458+t15673+t15674+t15676+t15678+t15855+t15856+(t13627.*(-t1476-t1540+t2091+t2165+t2579+t8.*(t260+t468+t570+t2298)))./4.0+(t13313.*(t1589-t2213+t3195-t4346+t4355+t4748.*7.35522e-1+t2772.*(t71-t391)+t2775.*(t71-t391)))./4.0+(t6951.*(t71-t391))./2.0+(t539.*(t1912.*(-1.196e-3)-t1942+t2518+t3589+t696.*(t71-t391)+t891.*(t71-t391)))./2.0+(t8628.*(t1589-t2213-t4346+t4355+t9454+t11863+t2772.*(t71-t391)+t2775.*(t71-t391)))./4.0+(t9233.*(t3423+t3845+t3888+t3925+t4339+t9.*(t210+t2107+t7423+t9121).*7.35522e-1+t17.*(t9166-t11658).*7.35522e-1))./4.0+(t14035.*(t249-t391.*(1.1e+1./1.25e+2)-t1912.*4.252e-3+t3505+t5357+t693.*(t71-t391)+t784.*(t71-t391)))./4.0+(t10398.*(t249-t391.*(1.1e+1./1.25e+2)-t1912.*4.252e-3+t3505+t13496+t693.*(t71-t391)+t784.*(t71-t391)))./4.0+(t13038.*(-t3045-t3218+t3458+t3539+t3878+t8.*(t260+t468+t570+t2298).*1.666555))./4.0+(t10783.*(t2091+t2497+t2579+t2680+t3516+t9.*(t210+t2107+t7423+t9121)+t17.*(t9166-t11658)))./4.0+t5.*t12.*(-t3405+t4994+t5076).*2.01382560198e-1)-q6d.*t16385-q2d.*t16474-q4d.*(t4831+t5358+t5377+t5506+t5591+t5594+t5767+t5926+t5959+t6083+t6861+t6962+t7012+t7072+t7107+t7324+t7380+t7661+t7663+t7709+t7725+t8074+t8098+t8629+t8815+t8961+t8990+t9054+t9089+t9864+t9983+t10148+t10701-t11268+t11269+t11383+t11401+t11458-t11461+t11463-t11474+t11574+t11584+t11655-t11657+t11898+t12021-t12317-t12454-t12597+t12609-t12828+t12844+t13221+t13420+t13564+t13570-t13633+t13637+t13719+t13723-t13845+t13848+t13859+t14078+t14132+t14188-t14296+t14298-t14347+t14348-t14847-t14849-t14878-t14880+t15163+t15164+t15318+t15326-t15605-t15606+t15849+t15850+(t6190.*(-t1053-t3327+t5081.*1.225946+t7731+t15.*t223.*1.4653732538e-2))./4.0+(t14541.*(t3418-t3879+t4324-t5228+t5802+t9.*(t71-t391).*4.5305948634e-2+t17.*(t426-t581).*7.35522e-1))./4.0+(t9187.*(t3418-t3879+t4324+t11855+t9.*(t71-t391).*4.5305948634e-2+t17.*(t426-t581).*7.35522e-1+t9.*(t9166-t11658).*7.35522e-1))./4.0+(t14918.*(t1987-t2621+t3452-t4730+t5359+t9.*(t71-t391).*6.1597e-2+t17.*(t426-t581)))./4.0+(t13273.*(t1589-t2213+t3195-t4346+t4355+t4748.*7.35522e-1+t2772.*(t71-t391)+t2775.*(t71-t391)))./4.0+(t10501.*(t985+t3399-t13.*t42.*1.01140545e-1-t7.*t223.*5.034347249e-2))./4.0+(t8433.*(t1589-t2213-t4346+t4355+t9454+t11863+t2772.*(t71-t391)+t2775.*(t71-t391)))./4.0+(t13974.*(t249-t391.*(1.1e+1./1.25e+2)-t1912.*4.252e-3+t3505+t5357+t693.*(t71-t391)+t784.*(t71-t391)))./4.0+(t10096.*(t249-t391.*(1.1e+1./1.25e+2)-t1912.*4.252e-3+t3505+t13496+t693.*(t71-t391)+t784.*(t71-t391)))./4.0+(t10753.*(t1987-t2621+t3452+t11654+t9.*(t71-t391).*6.1597e-2+t17.*(t426-t581)+t9.*(t9166-t11658)))./4.0)+q7d.*(t7826+t8162+t8296+t9175+t9204+t11976+t12459-t13211+t13214+t15017+t15219+t15823+t15825+t15827+t15828+t15859+t15861+t15863+t15866+t9.*(t8963+t7.*(t5026+t5.*(t2959-t2967))).*3.867742437e-3+t17.*(t8963+t7.*(t5026+t5.*(t2959-t2967))).*1.563719772e-3)+q5d.*(t5882+t5909+t5994+t6543+t6782+t6854+t7120+t7165+t7889+t7975+t7991+t8042+t8045+t8246+t8535+t8621+t8894+t9066+t9109+t9364+t9383-t9580-t10145+t11824+t11834-t12218-t12604+t13210+t13216+t13321+t13323+t13464+t13483+t13613+t13614-t13817+t13833+t13834-t14019-t14020-t14105-t14106+t14637+t14692+t14806+t14903+t15020+t15022+t15067+t15071+t15367+t15396+t15650+t15666+t15836-t15838-t15844+t15845+(t9744.*(t1292+t2073+t2694+t11671))./4.0+((-t3045+t3539+t14113).*(t1492+t2158+t2696-t4727))./4.0+((-t1476+t2165+t13876).*(t3063+t3528+t3966-t5230))./4.0+((t2810+t2988-t12589).*(t495+t572+t1838+t2069+t2107))./4.0+((t921+t1317-t5853).*(t3129+t3384+t3574+t7846+t9332))./4.0+(t11470.*(-t2550+t2696+t2698+t11659+t8.*t11672+t147.*(t71-t391)))./4.0+(t10149.*(-t3823+t3970+t11861+t8.*t11864+t972.*(t71-t391)+t2777.*(t71-t391)))./4.0+(t12792.*(-t1476-t1540+t2091+t2165+t2579+t8.*(t260+t468+t570+t2298)))./4.0+(t12385.*(t2437+t2648+t3129+t3384+t3574))./4.0+(t12392.*(-t3045-t3218+t3458+t3539+t3878+t8.*(t260+t468+t570+t2298).*1.666555))./4.0+(t8227.*(t3116+t3486+t3963+t11671.*1.666555))./4.0)-q1d.*(t3.*(-1.409188914000009e-4)+t11.*6.90020411512e-3+(t4916.*(t5026+t5.*(t2959-t2967)))./2.0+(t6713.*(t5026+t5.*(t2959-t2967)))./2.0-(t13198.*(-t1476-t1540+t2091+t2165+t2579+t8.*(t260+t468+t570+t2298)))./2.0+t18.*t4959.*2.26100637e-3+t24.*t4959.*2.26100637e-3+(t2087.*t5795)./2.0+(t3405.*t7952)./2.0+(t4936.*t7108)./2.0-(t4557.*t9325)./2.0-(t6750.*t8931)./2.0+(t8227.*t13196)./2.0+(t9744.*t13005)./2.0+(t10149.*t14879)./2.0+(t11470.*t14752)./2.0+(t3350.*(t5462+t5.*(t2959-t2967).*3.228604))./2.0-(t13005.*(t1589-t2213+t3195-t4346+t4355+t4748.*7.35522e-1+t2772.*(t71-t391)+t2775.*(t71-t391)))./2.0+(t7822.*(t9125+t7.*(t5026+t5.*(t2959-t2967)).*1.666555))./2.0+((t13026+t17.*(t8963+t7.*(t5026+t5.*(t2959-t2967)))).*(t3418-t3879+t4324-t5228+t5802+t9.*(t71-t391).*4.5305948634e-2+t17.*(t426-t581).*7.35522e-1))./2.0-(t4356.*(t2959-t2967))./2.0+(t4611.*(t5454-t7513))./2.0+(t6767.*(t5027-t7134))./2.0-(t6190.*(t5457-t7520))./2.0-(t8711.*(t5027-t7134))./2.0-(t7039.*(t9128+t7.*(t5026+t5.*(t2959-t2967)).*1.225946))./2.0-(t13197.*(t249-t391.*(1.1e+1./1.25e+2)-t1912.*4.252e-3+t3505+t5357+t693.*(t71-t391)+t784.*(t71-t391)))./2.0-(t9236.*(t8963+t7.*(t5026+t5.*(t2959-t2967))))./2.0+(t9967.*(t8963+t7.*(t5026+t5.*(t2959-t2967))))./2.0-(t13013.*(-t3045-t3218+t3458+t3539+t3878+t8.*(t260+t468+t570+t2298).*1.666555))./2.0+((t13145+t17.*(t8963+t7.*(t5026+t5.*(t2959-t2967))).*7.35522e-1).*(t1987-t2621+t3452-t4730+t5359+t9.*(t71-t391).*6.1597e-2+t17.*(t426-t581)))./2.0+((t5453+t5.*(t2959-t2967).*3.587895).*(t85+t338+t362+t375+t408+t5.*t12.*(7.9e+1./2.5e+2)))./2.0+(t11344.*(t921+t1317-t5853))./2.0+(t10931.*(t2810+t2988-t7937))./2.0+t12.*t3318.*t4959.*1.614302+(t12.*t4908.*t4959)./2.0)+yd.*(-t3860+t3958-t4535-t4632-t5577-t5579-t6236-t6371-t6593+t7145+t7153+t7436+t7437+t7459+t7492+t7504+t7532+t7602+t7632+t7637+t7966+t8007+t8125+t8130+t8211+t8293+t8337-t8357+t8363-t8393+t8401+t8472+t8811+t8824+t9464+t9699+t9730+t10082+t10083+t10088+t10097+t10099+t10102+t10311+t10334+t10571+t10575+t10670+t10909+t10913+t11730+t11801+t11803+t11804+t11813+t11814+t11815-t12134+t12158+t12324+t12330-t12430+t12629-t12657+t12685+t12706+t12715-t13065+t13264-t13790+t13792+t13793+t13800+t13801+t13804+t13805+t13806-t14043+t14054+t14313+t14325+t14433+t14587+t14606+t14748+t15252+t15253+t15254+t15255+t15259+t15260+t15327-t15331+t15465-t15467+t15565+t15570+t15622+t15627+t15630+t15734+t15931+t15932+t15940+t15941+t16040+t16044+t16058+t16062+(t12279.*(t1589-t2213+t3195-t4346+t4355+t4748.*7.35522e-1+t2772.*(t71-t391)+t2775.*(t71-t391)))./4.0+(t4356.*(t2425-t2468))./4.0+(t6190.*(t5110-t6808))./4.0+(t8711.*(t4542-t6448))./4.0+(t12484.*(t249-t391.*(1.1e+1./1.25e+2)-t1912.*4.252e-3+t3505+t5357+t693.*(t71-t391)+t784.*(t71-t391)))./4.0),-q6d.*t16170-q5d.*t16206-q4d.*t16228-q3d.*t16247-q2d.*t16252-q7d.*(t7842+t8174+t8286+t9182+t9210+t11967+t12455+t13269+t13460+(t9292.*(t3418-t3879+t4324-t5228+t5802+t9.*(t71-t391).*4.5305948634e-2+t17.*(t426-t581).*7.35522e-1))./2.0+(t10446.*(t1987-t2621+t3452-t4730+t5359+t9.*(t71-t391).*6.1597e-2+t17.*(t426-t581)))./2.0),t16253+t16420+t16424+t16475+q5d.*(t3806+t3818+t3974+t3983+t4108+t4155+t4171+t4184+t4245+t4316+t4343+t4431+t4439+t4766+t4803+t5368+t5520+t5548+t5627+t5717+t5768+t5770+t5792+t5799+t6059+t6157+t6266+t6389+t6426+t6429+t6557+t6564+t6945+t7035+t7143+t7203+t7211+t7375+t7592+t7616+t7706+t7711+t7812+t7816+t7843+t7906+t7924+t8200+t8257+t8359+t8409+t8611+t8625+t8664+t8726+t8901+t8924+t8965+t9004+t9192+t9308-t9352+t9672+t9676+t9883+t9900+t9927+t9937+t9938-t9969+t9990+t10015+t10281+t10347+t10366+t10516+t10717-t10751+t10788-t10805+t11029-t11060+t11104-t11133+t11302+t11310+t11411+t12001+t12003-t12356+t12404-t12460+t12490+t12812+t12813+t12938+t12940+(t8979.*(t2740+t3849+t3968+t3972-t5255+t17.*(t260+t468+t570+t2298).*7.35522e-1))./4.0+(t7646.*(-t1476-t1540+t2091+t2165+t2579+t8.*(t260+t468+t570+t2298)))./4.0+(t8981.*(-t3823+t3970+t5243+t9.*(t260+t468+t570+t2298).*7.35522e-1+t972.*(t71-t391)+t2777.*(t71-t391)))./4.0+(t9112.*(t1492+t2158+t2696-t4727))./4.0+(t7116.*(t3063+t3528+t3966-t5230))./4.0+(t6014.*(-t3045-t3218+t3458+t3539+t3878+t8.*(t260+t468+t570+t2298).*1.666555))./4.0+(t10468.*(t824+t2543+t2699+t2707-t4767+t17.*(t260+t468+t570+t2298)))./4.0+(t10469.*(-t2550+t2696+t2698+t4771+t9.*(t260+t468+t570+t2298)+t147.*(t71-t391)))./4.0)-q7d.*(t4484+t4576+t4580+t4749+t4773+t4786+t5002+t5030+t5643+t5658+t6384+t6387-t6965+t7258-t7472-t7744-t8540-t8593+t9003-t11218+t11611-t11933+t12178-t12640+t12643+t12748-t12895+t12899+t12984+(t6276.*(t1918+t9.*(t71-t391)))./4.0+(t8622.*(t395+t9.*(t48-t349)))./4.0+(t7949.*(t3418-t3879+t4324-t5228+t5802+t9.*(t71-t391).*4.5305948634e-2+t17.*(t426-t581).*7.35522e-1))./4.0+(t9361.*(t1987-t2621+t3452-t4730+t5359+t9.*(t71-t391).*6.1597e-2+t17.*(t426-t581)))./4.0+(t1907.*(t1912.*(-1.0027e-2)+t2709+t3492+t751.*(t71-t391)))./4.0)+q6d.*t16266+q4d.*t16357+q3d.*t16398,t16248+t16414+t16418+t16460-q7d.*t16172-q6d.*t16250+q5d.*t16317+q4d.*t16341-q2d.*t16398,t16229-t16412-q7d.*t16164-q6d.*t16245+q5d.*t16294-q3d.*t16341-q2d.*t16357+phid.*(t4831+t5358+t5377+t5506+t5611+t5616+t5767+t5926+t5959+t6083+t6861+t6962+t7012+t7072+t7107+t7324+t7380+t7648+t7675+t7709+t7725+t8074+t8098+t8629+t8815+t8961+t8990+t9054+t9089+t9864+t9975+t10146+t10701-t11268+t11269+t11391+t11393+t11458-t11461+t11463-t11474+t11575+t11583+t11655-t11657+t11895+t12016-t12317-t12454-t12597+t12609-t12828+t12844+t13221+t13420+t13568+t13573-t13633+t13637+t13720+t13728-t13845+t13848+t13864+t14078+t14136+t14188-t14296+t14298-t14347+t14348-t14847-t14849-t14878-t14880+t15161+t15162+t15314+t15323-t15605-t15606+t15849+t15850+(t6190.*(-t1053-t3327+t5081.*1.225946+t7731+t15.*t223.*1.4653732538e-2))./4.0+(t14541.*(t3418-t3879+t4324-t5228+t5802+t9.*(t71-t391).*4.5305948634e-2+t17.*(t426-t581).*7.35522e-1))./4.0+(t9187.*(t3418-t3879+t4324+t11855+t9.*(t71-t391).*4.5305948634e-2+t17.*(t426-t581).*7.35522e-1+t9.*(t9166-t11658).*7.35522e-1))./4.0+(t14918.*(t1987-t2621+t3452-t4730+t5359+t9.*(t71-t391).*6.1597e-2+t17.*(t426-t581)))./4.0+(t13273.*(t1589-t2213+t3195-t4346+t4355+t4748.*7.35522e-1+t2772.*(t71-t391)+t2775.*(t71-t391)))./4.0+(t10501.*(t985+t3399-t13.*t42.*1.01140545e-1-t7.*t223.*5.034347249e-2))./4.0+(t8433.*(t1589-t2213-t4346+t4355+t9454+t11863+t2772.*(t71-t391)+t2775.*(t71-t391)))./4.0+(t13974.*(t249-t391.*(1.1e+1./1.25e+2)-t1912.*4.252e-3+t3505+t5357+t693.*(t71-t391)+t784.*(t71-t391)))./4.0+(t10096.*(t249-t391.*(1.1e+1./1.25e+2)-t1912.*4.252e-3+t3505+t13496+t693.*(t71-t391)+t784.*(t71-t391)))./4.0+(t10753.*(t1987-t2621+t3452+t11654+t9.*(t71-t391).*6.1597e-2+t17.*(t426-t581)+t9.*(t9166-t11658)))./4.0)+xd.*(t5283+t5287+t7042+t7055+t9480-t9620+t9626+t9629+t9718-t10012+t10034-t10138+t10317-t10448+t10621+t10643+t10682+t10838+t10843+t10972+t11138-t11241+t11325+t11687-t11873-t11885+t12119+t12184-t12231-t12255+t12605+t12876+t12880-t12966+t12968+t13094+t13095+t13193+t13342-t13359-t13425+t13655-t13727-t13850-t14140+t14508+t14630+t14634+t14771+t14834+t14836+t15143+t15378+(t5598.*(t4540+t5.*(t2425-t2468)))./4.0+(t8713.*(t10158+t16.*(t4542-t6448)))./4.0+(t9187.*(t10403+t9.*(t10158+t16.*(t4542-t6448)).*7.35522e-1))./4.0+(t12689.*(t3418-t3879+t4324-t5228+t5802+t9.*(t71-t391).*4.5305948634e-2+t17.*(t426-t581).*7.35522e-1))./4.0+(t12945.*(t1987-t2621+t3452-t4730+t5359+t9.*(t71-t391).*6.1597e-2+t17.*(t426-t581)))./4.0+(t10936.*(t1589-t2213+t3195-t4346+t4355+t4748.*7.35522e-1+t2772.*(t71-t391)+t2775.*(t71-t391)))./4.0+(t2701.*(t5122+t5.*(t2425-t2468).*3.587895))./4.0+(t4557.*(t5124-t6795))./4.0+(t4774.*(t5110-t6808))./4.0+(t6750.*(t4542-t6448))./4.0+(t6744.*(t10384+t16.*(t4542-t6448).*1.666555))./4.0+(t11340.*(t249-t391.*(1.1e+1./1.25e+2)-t1912.*4.252e-3+t3505+t5357+t693.*(t71-t391)+t784.*(t71-t391)))./4.0+(t10753.*(t10174+t9.*(t10158+t16.*(t4542-t6448))))./4.0+t15.*t7039.*(t4542-t6448).*3.064865e-1+(t15.*t9236.*(t4542-t6448))./4.0),t16207+t16368+t16370+t16433-q2d.*(t3806+t3818+t3974+t3983+t4108+t4155+t4171+t4184+t4245+t4316+t4343+t4431+t4439+t4766+t4803+t5368+t5520+t5548+t5627+t5717+t5768+t5770+t5792+t5799+t6059+t6157+t6266+t6389+t6426+t6429+t6557+t6564+t6945+t7035+t7143+t7203+t7211+t7375+t7592+t7616+t7706+t7711+t7812+t7816+t7843+t7906+t7924+t8200+t8257+t8359+t8409+t8611+t8625+t8664+t8726+t8901+t8924+t8965+t9004+t9192+t9308-t9352+t9672+t9676+t9883+t9900+t9927+t9937+t9938-t9969+t9990+t10015+t10281+t10347+t10366+t10516+t10717-t10751+t10788-t10805+t11029-t11060+t11104-t11133+t11302+t11310+t11411+t12001+t12003-t12356+t12404-t12460+t12490+t12812+t12813+t12938+t12940+(t8979.*(t2740+t3849+t3968+t3972-t5255+t17.*(t260+t468+t570+t2298).*7.35522e-1))./4.0+(t7646.*(-t1476-t1540+t2091+t2165+t2579+t8.*(t260+t468+t570+t2298)))./4.0+(t8981.*(-t3823+t3970+t5243+t9.*(t260+t468+t570+t2298).*7.35522e-1+t972.*(t71-t391)+t2777.*(t71-t391)))./4.0+(t9112.*(t1492+t2158+t2696-t4727))./4.0+(t7116.*(t3063+t3528+t3966-t5230))./4.0+(t6014.*(-t3045-t3218+t3458+t3539+t3878+t8.*(t260+t468+t570+t2298).*1.666555))./4.0+(t10468.*(t824+t2543+t2699+t2707-t4767+t17.*(t260+t468+t570+t2298)))./4.0+(t10469.*(-t2550+t2696+t2698+t4771+t9.*(t260+t468+t570+t2298)+t147.*(t71-t391)))./4.0)-q4d.*t16294-q3d.*t16317-q7d.*(-t4652-t4658+t4757+t4840+t5267+t5296+t5687-t5698+t5773+t5803+t7148+t7195+t7207+t8626+t8682+t8881+t9257+t10321+t10578+t10599+t10855+t10857+t10965+t10979+t11452+t11827+t11828+t9.*(t260+t468+t570+t2298).*3.867742437e-3+t17.*(t260+t468+t570+t2298).*1.563719772e-3+t2963.*(t71-t391)+t3167.*(t71-t391)+t4080.*(t71-t391)+t4130.*(t71-t391))+q6d.*(-t4238+t4295-t4456+t4713+t4744+t4783+t4797+t4947+t5325+t5330+t5336+t5390-t5666+t5675+t5749+t5814+t6360+t6396+t7007+t7031+t7103+t7491+t7572+t7583+t7859+t7884+t8090+t8624+t8648+t8676+t8721+t8929+t8935+t8936+t8947+t9148+t9180+t9653+t9689-t10006+t10009+t10011+t10121+t10130+t10329+t10497+t10518+t10522+t10756-t10808+t11280+t11285+t11454+t11992+t11996+(t9.*(t578.*4.28e-4+t2566-t2597+t905.*(t71-t391)+t1021.*(t71-t391)))./4.0+t17.*(-t3823+t3970+t5243+t9.*(t260+t468+t570+t2298).*7.35522e-1+t972.*(t71-t391)+t2777.*(t71-t391)).*1.539925e-2+t8.*(t71-t391).*5.187945860934245e-5+t16.*(t71-t391).*4.67845486573025e-5+(t2522.*(t689-t740))./4.0+t17.*(-t2550+t2696+t2698+t4771+t9.*(t260+t468+t570+t2298)+t147.*(t71-t391)).*1.13264871585e-2+(t16.*t3286.*(t71-t391))./4.0),t16171+t16323+t16387+xd.*(-t8850-t8864-t10622+t10627+t11928+t12142-t12808-t12904+t13461+t13472+t13649+t13660+t13669+t13797+t13799+t13856+t14045+t14051+t14065+t14233+t14240-t14301-t14305-t14353-t14354+t14371+t14563+t14564+t15034+t15048+t15185+t15192)+q4d.*t16245+q3d.*t16250-q2d.*t16266+q7d.*(-t4446-t4631-t4668-t4758+t4796+t5014+t5186+t5242+t5249+t5260-t6377+t6390+t7125+t7190+t8614+t8666+t9074+t9268+t9882+t9885+t10307+t10601+t10606+t10707+t10708+t11438+t11702+t11703+t9.*(t348-t525).*8.36241330891889e-4)-q5d.*(-t4238+t4295-t4456+t4713+t4744+t4783+t4797+t4947+t5325+t5330+t5336+t5390-t5666+t5675+t5749+t5814+t6360+t6396+t7007+t7031+t7103+t7491+t7572+t7583+t7859+t7884+t8090+t8624+t8648+t8676+t8721+t8929+t8935+t8936+t8947+t9148+t9180+t9653+t9689-t10006+t10009+t10011+t10121+t10130+t10329+t10497+t10518+t10522+t10756-t10808+t11280+t11285+t11454+t11992+t11996+(t9.*(t578.*4.28e-4+t2566-t2597+t905.*(t71-t391)+t1021.*(t71-t391)))./4.0+t17.*(-t3823+t3970+t5243+t9.*(t260+t468+t570+t2298).*7.35522e-1+t972.*(t71-t391)+t2777.*(t71-t391)).*1.539925e-2+t8.*(t71-t391).*5.187945860934245e-5+t16.*(t71-t391).*4.67845486573025e-5+(t2522.*(t689-t740))./4.0+t17.*(-t2550+t2696+t2698+t4771+t9.*(t260+t468+t570+t2298)+t147.*(t71-t391)).*1.13264871585e-2+(t16.*t3286.*(t71-t391))./4.0),t16220+t16227+q2d.*(t4484+t4576+t4580+t4749+t4773+t4786+t5002+t5030+t5643+t5658+t6384+t6387-t6965+t7258-t7472-t7744-t8540-t8593+t9003-t11218+t11611-t11933+t12178-t12640+t12643+t12748-t12895+t12899+t12984+(t6276.*(t1918+t9.*(t71-t391)))./4.0+(t8622.*(t395+t9.*(t48-t349)))./4.0+(t7949.*(t3418-t3879+t4324-t5228+t5802+t9.*(t71-t391).*4.5305948634e-2+t17.*(t426-t581).*7.35522e-1))./4.0+(t9361.*(t1987-t2621+t3452-t4730+t5359+t9.*(t71-t391).*6.1597e-2+t17.*(t426-t581)))./4.0+(t1907.*(t1912.*(-1.0027e-2)+t2709+t3492+t751.*(t71-t391)))./4.0)+q4d.*t16164+q3d.*t16172+q5d.*(-t4652-t4658+t4757+t4840+t5267+t5296+t5687-t5698+t5773+t5803+t7148+t7195+t7207+t8626+t8682+t8881+t9257+t10321+t10578+t10599+t10855+t10857+t10965+t10979+t11452+t11827+t11828+t9.*(t260+t468+t570+t2298).*3.867742437e-3+t17.*(t260+t468+t570+t2298).*1.563719772e-3+t2963.*(t71-t391)+t3167.*(t71-t391)+t4080.*(t71-t391)+t4130.*(t71-t391))-q6d.*(-t4446-t4631-t4668-t4758+t4796+t5014+t5186+t5242+t5249+t5260-t6377+t6390+t7125+t7190+t8614+t8666+t9074+t9268+t9882+t9885+t10307+t10601+t10606+t10707+t10708+t11438+t11702+t11703+t9.*(t348-t525).*8.36241330891889e-4)+phid.*(t7842+t8174+t8286+t9182+t9210+t11968+t12456-t13211+t13214+t15013+t15216+t15822+t15824+t15826+t15829+t15860+t15862+t15864+t15865+t9.*(t8963+t7.*(t5026+t5.*(t2959-t2967))).*3.867742437e-3+t17.*(t8963+t7.*(t5026+t5.*(t2959-t2967))).*1.563719772e-3)+q1d.*(t7842+t8174+t8286+t9182+t9210+t11967+t12455+t13269+t13460+(t9292.*(t3418-t3879+t4324-t5228+t5802+t9.*(t71-t391).*4.5305948634e-2+t17.*(t426-t581).*7.35522e-1))./2.0+(t10446.*(t1987-t2621+t3452-t4730+t5359+t9.*(t71-t391).*6.1597e-2+t17.*(t426-t581)))./2.0),-phid.*t16469-q7d.*t16208-q6d.*t16302+q4d.*t16362-q1d.*t16421+q5d.*(t5581+t5592-t7358-t7366+t9411+t9440+t10019+t10409+t10660+t10693+t10828+t10837+t11089+t11096+t11471+t11489+t11697+t11733+t11737+t11939+t11962+t12056+t12061+t12070+t12242+t12244+t12264+t12412+t12612+t12613+t12716+t12851+t12868+t12950+t12967+t13153+t13222+t13240+t13424+t13431+t13598+t14014+t14414+t14415+t14701+t14706+t14912+t14915+t15118+t15119)-q3d.*(t5536+t5542+t5619+t6181+t6510+t6560+t7339+t7363+t7803+t7804+t7877+t7944+t7945+t8283+t8381+t8421+t8968+t8974-t9339+t9372+t9674+t9678-t9826+t9854+t10056+t10076+t10230+t10273+t10969-t10986+t11015+t11067+t11434+t11553+t11563+t11663-t11669-t11711-t11741+t11906+t11913+t11989+t12078-t12234-t12245+t12311+t12463-t12632-t12641+t12741-t12977-t13131-t13133+t13480+t13493-t13499-t13587-t13744-t13889+t13986+t13989-t14143+t14423+t14424+t14714+t14718-t15084-t15283+(t4841.*(t4540+t5.*(t2425-t2468)))./4.0+(t9106.*(t10158+t16.*(t4542-t6448)))./4.0+(t8999.*(t10403+t9.*(t10158+t16.*(t4542-t6448)).*7.35522e-1))./4.0+(t1490.*(t5122+t5.*(t2425-t2468).*3.587895))./4.0+(t7105.*(t10384+t16.*(t4542-t6448).*1.666555))./4.0+(t10480.*(t10174+t9.*(t10158+t16.*(t4542-t6448))))./4.0+t14.*t5713.*(t4540+t5.*(t2425-t2468)).*3.064865e-1+(t14.*t8437.*(t4540+t5.*(t2425-t2468)))./4.0)-q2d.*(t4.*t4436.*2.031994566e-3-t12.*t4436.*1.857971472e-2-(t3270.*t7247)./2.0+(t3275.*t7259)./2.0-(t5740.*t6442)./2.0+(t5750.*t6455)./2.0+(t5713.*t7246)./2.0+(t5634.*t8802)./2.0+(t6442.*t8437)./2.0+(t8050.*t8177)./2.0+(t8054.*t8213)./2.0+(t8213.*t9278)./2.0-(t7079.*t10607)./2.0+(t7116.*t10597)./2.0-(t8191.*t10612)./2.0+(t9112.*t10182)./2.0-(t9110.*t10199)./2.0-(t10141.*t10199)./2.0+(t8979.*t12520)./2.0+(t10468.*t12339)./2.0-(t5628.*(t5150-t6911))./2.0-(t6589.*(t5144-t6902))./2.0+(t8981.*(t8610-t10439))./2.0+(t10469.*(t8266-t10204))./2.0-t12.*t19.*t4436.*8.055302407919999e-1-t12.*t25.*t4436.*8.055302407919999e-1-t12.*t1572.*t4507.*1.7939475-t4.*t3261.*t4436.*1.614302-(t4.*t4436.*t4873)./2.0-(t12.*t4507.*t4843)./2.0),q6d.*(t8957+t8962+t11170+t11346+t11723+t12027+t12567+t12569+t12682+t12690+t13257+t13258+t13361+t13443+t13450+t13547+t13549+t13581+t13820+t13917+t13922+t13929+t13938+t14183+t14256+t14259+t14875+t14876+t15011+t15015-t8.*(t30.*(t2425-t2468)+t68.*(t2425-t2468)).*5.01208083475e-2-t16.*(t30.*(t2425-t2468)+t68.*(t2425-t2468)).*1.17633784675e-2)-q7d.*(t8350.*3.867742437e-3+t10735+t13312+t13522+t14948+t14954+t15093+t15095+t15099+t15109+t15295+t15304+t9.*(t16.*(t30.*(t2425-t2468)+t68.*(t2425-t2468))+t8.*(t7.*(t4650+t34.*(t2425-t2468))+t47.*(t2425-t2468))).*1.563719772e-3+t17.*(t4654+t15.*(t4650+t34.*(t2425-t2468))).*1.563719772e-3)-phid.*t16472-q1d.*t16422+q4d.*(t5297+t7682+t7739-t9159+t9258+t9265+t9399+t9438+t9529+t9541-t9573+t9662+t9873+t9899+t9993+t9994+t9995+t10251+t10477+t10887+t10897+t11090+t11279+t11442+t11447+t11620+t11767+t11783+t11785+t11851+t11929+t12437+t12445+t12644+t12647+t12986+t13136+t13144+t13190+t13259+t13265+t13556+t13580+t13589+t13592+t13599+t14003+t14229+t14239+t14486+t14491+t14957+t14959+t15190+t15195+(t7796.*(t9.*(t16.*(t30.*(t2425-t2468)+t68.*(t2425-t2468))+t8.*(t7.*(t4650+t34.*(t2425-t2468))+t47.*(t2425-t2468)))+t17.*(t4654+t15.*(t4650+t34.*(t2425-t2468)))))./4.0+(t5331.*(t30.*(t2425-t2468)+t68.*(t2425-t2468)))./4.0+(t6046.*(t16.*(t30.*(t2425-t2468)+t68.*(t2425-t2468))+t8.*(t7.*(t4650+t34.*(t2425-t2468))+t47.*(t2425-t2468))))./4.0+(t4024.*(t16.*(t30.*(t2425-t2468)+t68.*(t2425-t2468)).*1.666555+t8.*(t7.*(t4650+t34.*(t2425-t2468))+t47.*(t2425-t2468)).*1.666555))./4.0+t7.*(t7.*(t4650+t34.*(t2425-t2468)).*1.225946+t47.*(t2425-t2468).*1.225946).*8.639075e-2+t30.*(t2425-t2468).*9.5384188575e-2+t34.*(t2425-t2468).*1.8732399795e-1+t68.*(t2425-t2468).*9.5384188575e-2+(t3424.*(t30.*(t2425-t2468).*1.225946+t68.*(t2425-t2468).*1.225946))./4.0+t15.*(t4654+t15.*(t4650+t34.*(t2425-t2468))).*1.059103943995e-1+(t5443.*(t4654+t15.*(t4650+t34.*(t2425-t2468))))./4.0+t7.*(t7.*(t4650+t34.*(t2425-t2468))+t47.*(t2425-t2468)).*1.059103943995e-1+(t5329.*(t9.*(t16.*(t30.*(t2425-t2468)+t68.*(t2425-t2468))+t8.*(t7.*(t4650+t34.*(t2425-t2468))+t47.*(t2425-t2468))).*7.35522e-1+t17.*(t4654+t15.*(t4650+t34.*(t2425-t2468))).*7.35522e-1))./4.0)-q2d.*((t5750.*(t4650+t34.*(t2425-t2468)))./2.0+(t10468.*(t9.*(t16.*(t30.*(t2425-t2468)+t68.*(t2425-t2468))+t8.*(t7.*(t4650+t34.*(t2425-t2468))+t47.*(t2425-t2468)))+t17.*(t4654+t15.*(t4650+t34.*(t2425-t2468)))))./2.0-(t5740.*(t30.*(t2425-t2468)+t68.*(t2425-t2468)))./2.0+(t8437.*(t30.*(t2425-t2468)+t68.*(t2425-t2468)))./2.0+(t9112.*(t16.*(t30.*(t2425-t2468)+t68.*(t2425-t2468))+t8.*(t7.*(t4650+t34.*(t2425-t2468))+t47.*(t2425-t2468))))./2.0+(t8191.*(t8643-t8.*(t30.*(t2425-t2468)+t68.*(t2425-t2468)).*7.35522e-1))./2.0-(t3275.*t7320)./2.0-(t5628.*t8922)./2.0-(t6589.*t8927)./2.0+(t8981.*t12563)./2.0+(t7116.*(t16.*(t30.*(t2425-t2468)+t68.*(t2425-t2468)).*1.666555+t8.*(t7.*(t4650+t34.*(t2425-t2468))+t47.*(t2425-t2468)).*1.666555))./2.0+(t5634.*(t7.*(t4650+t34.*(t2425-t2468)).*1.225946+t47.*(t2425-t2468).*1.225946))./2.0+(t7079.*(t8646-t8.*(t30.*(t2425-t2468)+t68.*(t2425-t2468)).*1.666555))./2.0+t4.*(t2425-t2468).*2.031994566e-3-t12.*(t2425-t2468).*1.857971472e-2+(t5713.*(t30.*(t2425-t2468).*1.225946+t68.*(t2425-t2468).*1.225946))./2.0-(t3270.*(t30.*(t2425-t2468).*3.587895+t68.*(t2425-t2468).*3.587895))./2.0+(t8054.*(t4654+t15.*(t4650+t34.*(t2425-t2468))))./2.0+(t9278.*(t4654+t15.*(t4650+t34.*(t2425-t2468))))./2.0+(t8050.*(t7.*(t4650+t34.*(t2425-t2468))+t47.*(t2425-t2468)))./2.0-(t9110.*(t8315+t8.*(t30.*(t2425-t2468)+t68.*(t2425-t2468))))./2.0-(t10141.*(t8315+t8.*(t30.*(t2425-t2468)+t68.*(t2425-t2468))))./2.0-(t10469.*(t8329+t17.*(t16.*(t30.*(t2425-t2468)+t68.*(t2425-t2468))+t8.*(t7.*(t4650+t34.*(t2425-t2468))+t47.*(t2425-t2468)))))./2.0+(t8979.*(t9.*(t16.*(t30.*(t2425-t2468)+t68.*(t2425-t2468))+t8.*(t7.*(t4650+t34.*(t2425-t2468))+t47.*(t2425-t2468))).*7.35522e-1+t17.*(t4654+t15.*(t4650+t34.*(t2425-t2468))).*7.35522e-1))./2.0-t12.*t19.*(t2425-t2468).*8.055302407919999e-1-t12.*t25.*(t2425-t2468).*8.055302407919999e-1-t4.*t3261.*(t2425-t2468).*1.614302-(t4.*t4873.*(t2425-t2468))./2.0-t12.*t13.*t1572.*(t2425-t2468).*1.7939475-(t12.*t13.*t4843.*(t2425-t2468))./2.0)-q3d.*(t5593+t5599+t5638+t6519+t7392+t7427+t7852-t7874+t7879+t7896+t7917+t7918-t8279+t8307+t8428+t8450+t8946+t8954-t9082-t9403+t9422+t9687+t9700+t9876-t9888+t10108+t10129+t10245+t10302-t10308+t10970+t11041+t11077+t11435+t11629+t11634+t11664-t11670-t11743+t11948+t11966+t12031+t12091-t12258+t12312+t12476-t12633+t12760-t13122-t13540-t13550+t13563+t13566-t13762-t13912-t13921+t14004+t14008-t14158+t14416+t14418+t14711+t14713-t15113-t15114-t15308-t15310+(t5634.*(t6853-t6864))./4.0+(t5648.*(t6806-t8574))./4.0+(t8053.*(t6452-t8229))./4.0+(t7079.*(t6847-t9563))./4.0+(t8191.*(t6834-t9565))./4.0+(t9110.*(t6472-t9256))./4.0+(t10141.*(t6472-t9256))./4.0+t12.*t3243.*(t2425-t2468).*8.07151e-1+(t12.*t4860.*(t2425-t2468))./4.0)-q5d.*(t5624+t5630+t7408+t7426+t9491+t9500+t10037+t10422+t10741+t10752+t10866+t10874+t11146+t11167-t11488+t11503+t11719+t11754-t11960+t11981+t12064+t12263+t12280+t12728+t12906+t12914+t13015+t13029-t13245-t13272-t13439-t13452-t13602-t14026+t14428+t14430+t14717+t14721+t14931-t14936+t15125-t15129+(t5634.*(t6806-t8574))./4.0+(t8050.*(t6452-t8229))./4.0+t16.*t7079.*(t6452-t8229).*4.1663875e-1+t8.*t7116.*(t6452-t8229).*4.1663875e-1+t16.*t8191.*(t6452-t8229).*1.838805e-1+(t8.*t9112.*(t6452-t8229))./4.0+(t16.*t9110.*(t6452-t8229))./4.0+(t16.*t10141.*(t6452-t8229))./4.0),-t16394-t16468+t16471-q6d.*(t4232+t4409+t4413+t4417+t4698+t4715+t4813+t5184+t5238+t6375-t6485-t6572+t6608+t7114-t7243-t7432+t7549-t7640+t7911+t7925-t8134+t8165+t8268+t8528+t8542+t8579+t8659+t8758+t8801+t8885-t10120+t10287+t10300-t10856+t13634+t13698+t14009+t14077+t14644+t14646-t14650-t14652+t14672+t14675-t14742-t14743+t14759+t14765+t14947+t14962+t14965+t15131-t15197-t15199-t15267-t15268+t15769-t15776+t15787-t15792+(t6041.*(t1918+t9.*(t71-t391)))./4.0+(t10141.*(t3625+t3660+t9166-t11658))./4.0+(t8191.*(t4401+t4424+t9457-t11860))./4.0+(t5586.*(t71-t391))./4.0+(t5582.*(t348-t525))./4.0+(t6720.*(t348-t525))./4.0+((t348-t525).*(t1254+t1943+t9.*t439.*1.196e-3+t439.*t1083))./4.0)+q7d.*t16283-q5d.*t16440-q4d.*t16455-q1d.*t16474+q3d.*(-t2886-t3335+t3442+t3518+t3568+t3602+t3605+t3679+t3707+t3892+t4100+t4115+t4126+t4224+t4264+t4293+t4497+t4606+t4626+t4665+t4736+t4742+t4834+t4898+t4901+t4972+t5018+t5237+t5278+t5873+t5890+t5892+t5953+t5963+t5998+t6065+t6071+t6072+t6088+t6118+t6120+t6153+t6186+t6192+t6231+t6291+t6584+t6596+t6678+t6741+t6745+t6894+t6946+t7015+t7059+t7179+t7184+t7208+t7239+t7349+t7403+t7410+t7465+t7499+t7593+t7712+t7757+t7801+t7811+t7878+t7923+t7946+t7953+t8035+t8079+t8157+t8197+t8322+t8345+t8441+t8456+t8493+t8503+t8550+t8577+t8607+t8703+t8732+t8832+t8858+t8928+t8940+t9006+t9030+t9055+t9061+t9116+t9178+t9184+t9200+t9455+t9577+t9586+t9616+t9909+t9914+t9917+t9919+t10313+t10322+t10478+t10500+t11078+t11079+t11465+t11469+t11506+t11893+t11905+t12100+t12106+t12472+t12480+t12530+t12630+t12869+t12882+t12887+t12891+t12931+t13155+t13604+t13607+t13631+t13640+t13657+t13680+t13730+t13753+t13878+t13883+t14124+t14126+t14247+t14274+t14275+t14284+t14285+t14340+t14709+t14710+t14917+t14920+t14922+t14923+t15286+t15292+t15320+t15321+t15332+t15333+t15589+t15590+t15591+t15592+t15830+t15831+t15832+t15833)+q2d.*(t3281+t3383+t3407+t3601+t4209+t4319+t4513+t4553+t4625+t4876+t5256+t5883+t5925+t6134+t6135+t6242+t6788+t6827+t6912+t7115+t7445+t7470+t7779+t7915+t7978+t8208+t8504+t8590+t8759+t9008+t9029+(t5750.*(-t262+t1056+t1250+t5078+t5282+t4.*t13.*1.0442e-1))./2.0+t5.*t6205.*4.02765120396e-1+t13.*t6216.*4.02765120396e-1+t5.*t7422.*1.24749e-1-(t1572.*t8995)./2.0+(t3261.*t7386)./2.0+(t4873.*t6155)./2.0-(t4843.*t6353)./2.0-(t3270.*t10094)./2.0-(t5740.*t8697)./2.0+(t5713.*t11023)./2.0-(t5634.*t12042)./2.0+(t5628.*t12050)./2.0+(t8437.*t9499)./2.0-(t8050.*t10850)./2.0+(t8054.*t10858)./2.0+(t6589.*t12464)./2.0+(t7079.*t13326)./2.0-(t7116.*t13333)./2.0+(t9278.*t11266)./2.0+(t9110.*t12667)./2.0-(t9112.*t12696)./2.0+(t8191.*t13915)./2.0+(t10141.*t13150)./2.0+(t8979.*(t3543+t3820+t3911+t3949+t4360+t12067+t17.*(t258+t2289+t5392+t7559).*7.35522e-1))./2.0+(t8981.*(t3471+t3796+t3914+t3942+t4358+t9.*(t258+t2289+t5392+t7559).*7.35522e-1+t17.*(t7693+t9904).*7.35522e-1))./2.0-t13.*(-t2715+t3105+t5080.*3.228604).*1.24749e-1+t4.*(t2959-t2967).*2.031994566e-3-t1700.*(t2959-t2967)+(t10469.*(t2189+t2495+t2635+t2646+t3580+t9.*(t258+t2289+t5392+t7559)+t17.*(t7693+t9904)))./2.0+(t3275.*(-t1785+t2869+t2960+t5489+t5720+t4.*t13.*3.746479959e-1))./2.0+(t10468.*(t2148+t2513+t2649+t2661+t3582+t11950+t17.*(t258+t2289+t5392+t7559)))./2.0),-t16253-t16420-t16475+q7d.*t16177-q5d.*t16328-q4d.*t16358-q6d.*(t4225+t4232+t4268+t4409+t4413+t4417+t4698+t4715+t4813+t5184+t5238+t5651+t5684+t6375-t6485-t6572+t6608+t7114-t7243-t7432+t7549-t7640+t7911+t7925-t8134+t8165+t8268+t8579+t8659+t8758+t8801+t8885-t10120+t10421+t10482+t10638+t10645+t10732-t10749+t10789-t10856+t11049-t11054+t11109+t11126+t11423+t11487+t11691+t11718+t11725+t12090+t12248-t12431-t12432-t12572-t12585-t12594-t12599-t12815-t12821+(t6041.*(t1918+t9.*(t71-t391)))./4.0+(t7613.*(-t1476-t1540+t2091+t2165+t2579+t8.*(t260+t468+t570+t2298)))./4.0+(t5586.*(t71-t391))./4.0+(t5582.*(t348-t525))./4.0+(t6720.*(t348-t525))./4.0+((t348-t525).*(t1254+t1943+t9.*t439.*1.196e-3+t439.*t1083))./4.0+(t5923.*(-t3045-t3218+t3458+t3539+t3878+t8.*(t260+t468+t570+t2298).*1.666555))./4.0)-q3d.*(t2886+t3335+t3393+t3451+t3491+t3553-t3602+t3642-t3707+t3844+t4095-t4100+t4148-t4224+t4241-t4293-t4294-t4296+t4472+t4570-t4626-t4665-t4736-t4742-t4834+t4886+t4911+t4963+t4998+t5070-t5093+t5222+t5268+t5458-t5469-t5525-t5526+t5667+t5669-t5873+t5881-t5998+t6026+t6035+t6036+t6050-t6072-t6088+t6099-t6118+t6129+t6163-t6186-t6231+t6305+t6585+t6594+t6669+t6728+t6755+t6870+t6921-t6992-t6993-t7001-t7015-t7059-t7184-t7208+t7225+t7238+t7302+t7317-t7349+t7390+t7393+t7421+t7453+t7456-t7478+t7487+t7607+t7692+t7747+t7787+t7793+t7888+t7898-t7923-t7930+t7931+t8087+t8145-t8197+t8311-t8345-t8456+t8481+t8695+t8727-t8832+t8840+t9002+t9025+t9311+t9381+t9428-t9860-t9872-t9898-t9902+t10086-t10109-t10110+t10116+t10183+t10184-t10385+t10417+t10420+t10456-t10605+t10641+t10814+t10819+t10860-t11206-t11213+t11224-t11249-t11250-t11273-t11274-t11600-t11606+t11616+t11619+t11631+t11637+t11912+t12140-t12418-t12419+t12650+t12658+t12660+t12661-t12871-t12872-t12878-t12884+t13298+t13300+(t7469.*(t1918+t9.*(t71-t391)))./4.0+(t8999.*(t3418-t3879+t4324-t5228+t5802+t9.*(t71-t391).*4.5305948634e-2+t17.*(t426-t581).*7.35522e-1))./4.0+(t10480.*(t1987-t2621+t3452-t4730+t5359+t9.*(t71-t391).*6.1597e-2+t17.*(t426-t581)))./4.0+(t1907.*(t618.*4.28e-4-t1841-t2389+t2400-t2414+t17.*(t113-t409).*1.0027e-2))./4.0+(t8063.*(t1589-t2213+t3195-t4346+t4355+t4748.*7.35522e-1+t2772.*(t71-t391)+t2775.*(t71-t391)))./4.0+(t5723.*(t71-t391))./4.0+(t6709.*(t71-t391))./4.0+(t7497.*(t60-t394))./4.0+(t3261.*(t2798-t2848))./4.0+(t10111.*(t249-t391.*(1.1e+1./1.25e+2)-t1912.*4.252e-3+t3505+t5357+t693.*(t71-t391)+t784.*(t71-t391)))./4.0+(t5750.*(t263-t283-t310+t1265))./4.0-(t5.*t6.*t5783)./4.0)+q2d.*(t3281+t3383+t3407+t3601+t4209+t4319+t4513+t4553+t4625+t4876+t5256+t5883+t5925+t6134+t6135+t6242+t6788+t6827+t6912+t7115+t7445+t7470+t7779+t7915+t7978+t8208+t8504+t8590+t8759+t9008+t9029+t5.*t3356.*4.02765120396e-1+t13.*t3396.*4.02765120396e-1+t5.*t4922.*1.24749e-1+t13.*t4930.*1.24749e-1+(t3261.*t4906)./2.0+(t3316.*t4873)./2.0-(t1572.*t6693)./2.0-(t3720.*t4843)./2.0-(t3270.*t6763)./2.0+(t3275.*t6762)./2.0+(t4569.*t5750)./2.0-(t4604.*t5740)./2.0+(t5713.*t8689)./2.0+(t6114.*t8437)./2.0+(t5634.*t9209)./2.0+(t5628.*t9216)./2.0+(t6967.*t8050)./2.0+(t6988.*t8054)./2.0+(t6589.*t9992)./2.0+(t7079.*t9717)./2.0-(t7116.*t9743)./2.0+(t7875.*t9278)./2.0+(t8178.*t9110)./2.0-(t8253.*t9112)./2.0+(t8191.*t10863)./2.0+(t9196.*t10141)./2.0+(t8979.*t11483)./2.0+(t8981.*t11484)./2.0+(t10170.*t10468)./2.0+(t10180.*t10469)./2.0)+yd.*(t5229+t5533+t6212+t6293+t6300+t6319+t6357+t6437+t6577+t6643+t6647+t7330+t7388+t7791+t7823+t7908+t8313+t8353-t8367-t8392+t8400+t8447-t8452+t8849+t9346+t9356-t9417+t9526+t9623-t9756+t9757+t9836+t9846+t10236+t10350-t10364+t10451+t10535+t10867+t11076-t11235+t11244+t11724+t11736+t11784+t12057-t12155+t12235+t12247-t12544+t12545-t12679+t12721-t12996+t13010+t13024+t13506+t13542+t13603+t13776-t13814-t13836+t13892+t13906-t14052-t14060-t14075+t14163-t14310+t14312-t14365+t14604+t15072+t15080+t15275+t15281+t15368-t15371-t15479+t15483+((t7.*(t4650+t34.*(t2425-t2468)).*1.225946+t47.*(t2425-t2468).*1.225946).*(t921+t1317-t5853))./4.0+(t6767.*(t30.*(t2425-t2468)+t68.*(t2425-t2468)))./4.0+((t7.*(t4650+t34.*(t2425-t2468))+t47.*(t2425-t2468)).*(t2810+t2988-t7937))./4.0+(t6988.*(t6806-t8574))./4.0+(t7875.*(t6801-t8594))./4.0+(t9216.*(t6452-t8229))./4.0+(t9992.*(t6452-t8229))./4.0+(t4611.*(t30.*(t2425-t2468).*3.587895+t68.*(t2425-t2468).*3.587895))./4.0+(t9967.*(t4654+t15.*(t4650+t34.*(t2425-t2468))))./4.0+(t11470.*(t8329+t17.*(t16.*(t30.*(t2425-t2468)+t68.*(t2425-t2468))+t8.*(t7.*(t4650+t34.*(t2425-t2468))+t47.*(t2425-t2468)))))./4.0+t4.*t3318.*(t2425-t2468).*8.07151e-1+t12.*t3316.*(t2425-t2468).*8.07151e-1+(t4.*t4908.*(t2425-t2468))./4.0+(t12.*t4906.*(t2425-t2468))./4.0),q6d.*t16148+q5d.*t16175-q3d.*t16214-q7d.*(t6828+t6939+t8127-t12109+t12110+t12391-t12394+(t7475.*(t395+t9.*(t48-t349)))./2.0+(t439.*(-t2182+t2241+t696.*(t48-t349)+t891.*(t48-t349)))./2.0+(t10141.*(-t2149+t2205+t693.*(t48-t349)+t784.*(t48-t349)))./2.0+(t8191.*(t3479-t3544+t2772.*(t48-t349)+t2775.*(t48-t349)))./2.0)-q4d.*(-t2608+t3719+t3727+t4078+t4686+t4845+t4894+t4923+t4929+t5319+t5818+t5901+t5984+t6284+t6298+t6303+t6445+t6473+t6626+t6627+t6830+t7097+t7117+t7264+t7522+t7608+t7774+t7893+t7990+t8674+t8978+t8988+t9262+t9272+t9303+t10462+t10470+t10496+t10683+t10687+t10849+t11810+t11938+t12401+t12402+t12403+t12405),t16215-t16383-t16399-t16477+q6d.*(-t4065-t4081-t4136-t4175+t4180-t4234-t4376-t4419-t4974+t4990+t5545+t5691+t5718+t5745+t5865+t5867+t5941+t6282+t6348+t6352+t6388+t6398+t6412+t6464+t7033+t7076+t7086+t7122+t7167+t7455-t7537+t7669+t7698+t7782+t9221+t9235+t9243+t9246+t9286+t9295+t9329-t9486-t9489-t9612+t9660+t9807+t10027+t10035+t10077+t10126+t10458+t10492-t10680-t10745-t10748+t10935+t10958+t11034+t11313+t11318+t11337+t11357+t11680+t11684+(t1837.*(t689-t740))./4.0+(t3286.*(t60-t394))./4.0+(t3239.*(t357-t519))./4.0)+q7d.*t16162+q5d.*t16284-q4d.*t16325+yd.*(t5572+t5576+t5657+t6529+t7405+t7415+t7864+t7865-t7874+t7896+t7917+t7918-t8279+t8307+t8423+t8444+t8946+t8954-t9082-t9403+t9422+t9690+t9693+t9876-t9888+t10114+t10123+t10245+t10304-t10308+t10970+t11046+t11077+t11435+t11624+t11627+t11664-t11670-t11743+t11943+t11956+t12030+t12091-t12258+t12312+t12473-t12633+t12760-t13122-t13540-t13550+t13560+t13571-t13762-t13912-t13921+t14005+t14007-t14158+t14416+t14418+t14711+t14713-t15113-t15114-t15308-t15310+(t5634.*(t6853-t6864))./4.0+(t5648.*(t6806-t8574))./4.0+(t8053.*(t6452-t8229))./4.0+(t7079.*(t6847-t9563))./4.0+(t8191.*(t6834-t9565))./4.0+(t9110.*(t6472-t9256))./4.0+(t10141.*(t6472-t9256))./4.0+t12.*t3243.*(t2425-t2468).*8.07151e-1+(t12.*t4860.*(t2425-t2468))./4.0),t16190-t16359+t16361+t16457+q7d.*(-t3995-t4013-t4190-t4197+t4291+t4306+t4448+t4462+t4520+t4539+t5127+t5140-t5688+t5906+t6001-t6439+t6487+t6491+t7633+t7758-t10457-t10565+t10573+t10755-t10760-t10844+t10845-t11160+t11236-t11240+(t5837.*(t395+t9.*(t48-t349)))./4.0+(t8477.*(-t2149+t2205+t693.*(t48-t349)+t784.*(t48-t349)))./4.0+(t5696.*(t3479-t3544+t2772.*(t48-t349)+t2775.*(t48-t349)))./4.0+(t15.*t16.*(-t2182+t2241+t696.*(t48-t349)+t891.*(t48-t349)))./4.0)-q6d.*t16217+q5d.*t16261+q3d.*t16325+yd.*(t5297+t7666+t7719-t9159+t9267+t9274+t9418+t9421+t9542+t9551-t9573+t9651+t9886+t9889+t9988+t10000+t10002+t10262+t10479+t10891+t10902+t11093+t11279+t11443+t11446+t11620+t11771+t11776+t11790+t11851+t11931+t12439+t12445+t12639+t12649+t12982+t13139+t13141+t13190+t13253+t13260+t13552+t13575+t13583+t13592+t13596+t14002+t14232+t14234+t14487+t14489+t14956+t14958+t15189+t15193+(t7796.*(t9.*(t16.*(t30.*(t2425-t2468)+t68.*(t2425-t2468))+t8.*(t7.*(t4650+t34.*(t2425-t2468))+t47.*(t2425-t2468)))+t17.*(t4654+t15.*(t4650+t34.*(t2425-t2468)))))./4.0+(t5331.*(t30.*(t2425-t2468)+t68.*(t2425-t2468)))./4.0+(t6046.*(t16.*(t30.*(t2425-t2468)+t68.*(t2425-t2468))+t8.*(t7.*(t4650+t34.*(t2425-t2468))+t47.*(t2425-t2468))))./4.0+(t4024.*(t16.*(t30.*(t2425-t2468)+t68.*(t2425-t2468)).*1.666555+t8.*(t7.*(t4650+t34.*(t2425-t2468))+t47.*(t2425-t2468)).*1.666555))./4.0+t7.*(t7.*(t4650+t34.*(t2425-t2468)).*1.225946+t47.*(t2425-t2468).*1.225946).*8.639075e-2+t30.*(t2425-t2468).*9.5384188575e-2+t34.*(t2425-t2468).*1.8732399795e-1+t68.*(t2425-t2468).*9.5384188575e-2+(t3424.*(t30.*(t2425-t2468).*1.225946+t68.*(t2425-t2468).*1.225946))./4.0+t15.*(t4654+t15.*(t4650+t34.*(t2425-t2468))).*1.059103943995e-1+(t5443.*(t4654+t15.*(t4650+t34.*(t2425-t2468))))./4.0+t7.*(t7.*(t4650+t34.*(t2425-t2468))+t47.*(t2425-t2468)).*1.059103943995e-1+(t5329.*(t9.*(t16.*(t30.*(t2425-t2468)+t68.*(t2425-t2468))+t8.*(t7.*(t4650+t34.*(t2425-t2468))+t47.*(t2425-t2468))).*7.35522e-1+t17.*(t4654+t15.*(t4650+t34.*(t2425-t2468))).*7.35522e-1))./4.0),-t16176+t16330-t16442+yd.*(t5642+t5652+t7414+t7417+t9495+t9508+t10037+t10422+t10746+t10750+t10869+t10870+t11140+t11154-t11488+t11503+t11719+t11754-t11960+t11981+t12064+t12263+t12280+t12728+t12910+t12911+t13017+t13022-t13245-t13272-t13439-t13452-t13602-t14026+t14428+t14430+t14717+t14721+t14931-t14936+t15125-t15129+(t5634.*(t6806-t8574))./4.0+(t8050.*(t6452-t8229))./4.0+t16.*t7079.*(t6452-t8229).*4.1663875e-1+t8.*t7116.*(t6452-t8229).*4.1663875e-1+t16.*t8191.*(t6452-t8229).*1.838805e-1+(t8.*t9112.*(t6452-t8229))./4.0+(t16.*t9110.*(t6452-t8229))./4.0+(t16.*t10141.*(t6452-t8229))./4.0)+q7d.*(-t3674-t3725+t4277+t4347+t4353+t4442-t4449+t4817+t4823-t5008+t5022-t5031-t5053+t5313+t5380+t6316+t6414+t6419+t7516+t7587+t8265+t8818+t9453+t9582+t9596+t9758+t9762+t10065+t10069+t10721+t10803+t10811-t16.*t321.*2.454825983680473e-3)-q6d.*t16197-q4d.*t16261-q3d.*t16284+xd.*(-t5605-t5612+t7342+t7377+t9411+t9440+t10010+t10405+t10660+t10693+t10828+t10837+t11089+t11096-t11471+t11485+t11690+t11728-t11733-t11939+t11954+t12055-t12061-t12070+t12238-t12244+t12259-t12412-t12612-t12613+t12713+t12851+t12868+t12950+t12967-t13153-t13222-t13424-t13598-t14014+t14410+t14412+t14699+t14703+t14910+t15116+(t7646.*(t10158+t16.*(t4542-t6448)))./4.0+(t7799.*(t10403+t9.*(t10158+t16.*(t4542-t6448)).*7.35522e-1))./4.0+(t6014.*(t10384+t16.*(t4542-t6448).*1.666555))./4.0+(t9537.*(t10174+t9.*(t10158+t16.*(t4542-t6448))))./4.0),-t16149-t16267-t16304+t16307-t16396-q3d.*(-t4065-t4081-t4136-t4175+t4180-t4234-t4376-t4419-t4974+t4990+t5545+t5691+t5718+t5745+t5865+t5867+t5941+t6282+t6348+t6352+t6388+t6398+t6412+t6464+t7033+t7076+t7086+t7122+t7167+t7455-t7537+t7669+t7698+t7782+t9221+t9235+t9243+t9246+t9286+t9295+t9329-t9486-t9489-t9612+t9660+t9807+t10027+t10035+t10077+t10126+t10458+t10492-t10680-t10745-t10748+t10935+t10958+t11034+t11313+t11318+t11337+t11357+t11680+t11684+(t1837.*(t689-t740))./4.0+(t3286.*(t60-t394))./4.0+(t3239.*(t357-t519))./4.0)+q5d.*t16197+q4d.*t16217+q7d.*(t4230+t4248-t4443-t4577+t4593+t4639+t4676+t4717+t4806-t5568+t5585+t6288+t6364+t7479+t7557+t8596+t8696+t8702+t8843+t9424+t9447+t9460+t9673+t9675+t10705+t10733+t10734+t9.*(t208-t427).*3.867742437e-3+t17.*(t208-t427).*1.563719772e-3),-t16210+t16212+q1d.*(t4484+t4576+t4580+t4749+t4773+t4786+t5002+t5030+t5643+t5658+t6384+t6387-t6965+t7258-t7472-t7744-t8540-t8593+t9003-t11218+t11611-t11933+t12178-t12640+t12643+t12748-t12895+t12899+t12984+(t6276.*(t1918+t9.*(t71-t391)))./4.0+(t8622.*(t395+t9.*(t48-t349)))./4.0+(t7949.*(t3418-t3879+t4324-t5228+t5802+t9.*(t71-t391).*4.5305948634e-2+t17.*(t426-t581).*7.35522e-1))./4.0+(t9361.*(t1987-t2621+t3452-t4730+t5359+t9.*(t71-t391).*6.1597e-2+t17.*(t426-t581)))./4.0+(t1907.*(t1912.*(-1.0027e-2)+t2709+t3492+t751.*(t71-t391)))./4.0)-q4d.*(-t3995-t4013-t4190-t4197+t4291+t4306+t4448+t4462+t4520+t4539+t5127+t5140-t5688+t5906+t6001-t6439+t6487+t6491+t7633+t7758-t10457-t10565+t10573+t10755-t10760-t10844+t10845-t11160+t11236-t11240+(t5837.*(t395+t9.*(t48-t349)))./4.0+(t8477.*(-t2149+t2205+t693.*(t48-t349)+t784.*(t48-t349)))./4.0+(t5696.*(t3479-t3544+t2772.*(t48-t349)+t2775.*(t48-t349)))./4.0+(t15.*t16.*(-t2182+t2241+t696.*(t48-t349)+t891.*(t48-t349)))./4.0)-q5d.*(-t3674-t3725+t4277+t4347+t4353+t4442-t4449+t4817+t4823-t5008+t5022-t5031-t5053+t5313+t5380+t6316+t6414+t6419+t7516+t7587+t8265+t8818+t9453+t9582+t9596+t9758+t9762+t10065+t10069+t10721+t10803+t10811-t16.*t321.*2.454825983680473e-3)-q3d.*t16162-q6d.*(t4230+t4248-t4443-t4577+t4593+t4639+t4676+t4717+t4806-t5568+t5585+t6288+t6364+t7479+t7557+t8596+t8696+t8702+t8843+t9424+t9447+t9460+t9673+t9675+t10705+t10733+t10734+t9.*(t208-t427).*3.867742437e-3+t17.*(t208-t427).*1.563719772e-3)+q2d.*(t6828+t6939+t8127-t12109+t12110+t12391-t12394+(t7475.*(t395+t9.*(t48-t349)))./2.0+(t439.*(-t2182+t2241+t696.*(t48-t349)+t891.*(t48-t349)))./2.0+(t10141.*(-t2149+t2205+t693.*(t48-t349)+t784.*(t48-t349)))./2.0+(t8191.*(t3479-t3544+t2772.*(t48-t349)+t2775.*(t48-t349)))./2.0)+phid.*(t4484+t4576+t4580+t4749+t4773+t4786+t5002+t5030-t6965+t7258-t7472-t7744-t8540-t8593+t9003+t10285+t10292-t11218-t11933+t12219+t12221+t14924+t15122+t15777+t15779+t15794+t15796+(t6276.*(t1918+t9.*(t71-t391)))./4.0+(t8622.*(t395+t9.*(t48-t349)))./4.0+(t7949.*(t3418-t3879+t4324+t11855+t9.*(t71-t391).*4.5305948634e-2+t17.*(t426-t581).*7.35522e-1+t9.*(t9166-t11658).*7.35522e-1))./4.0+(t1907.*(t1912.*(-1.0027e-2)+t2709+t3492+t751.*(t71-t391)))./4.0+(t7940.*(t3423+t3845+t3888+t3925+t4339+t9.*(t210+t2107+t7423+t9121).*7.35522e-1+t17.*(t9166-t11658).*7.35522e-1))./4.0+(t9362.*(t2091+t2497+t2579+t2680+t3516+t9.*(t210+t2107+t7423+t9121)+t17.*(t9166-t11658)))./4.0+(t9361.*(t1987-t2621+t3452+t11654+t9.*(t71-t391).*6.1597e-2+t17.*(t426-t581)+t9.*(t9166-t11658)))./4.0),-phid.*(-t5514-t5527-t5571-t5575-t6249+t6613+t7763+t8161+t8861+t8902+t9085+t9088+t9406+t9476+t10324+t10356+t10401+t10512+t10538+t10559+t10594+t10651+t10900+t10919+t10934+t11246+t11267+t11359+t11365+t11539+t11540+t11566+t11601+t11706+t11713+t11715+t11800+t12043+t12084+t12309+t12313+t12336+t12555+t12845+t13104+t13112+t13270+t13282+t13316+t13708+t13918+t13933+t14059+t14102+t14109+t14118+t14133+t14236+t14356+t14358+t14378+t14551+t14811+t14829+t15051+t15060+t15246+t15261+t15399+t15423+t15425+t15433+t15438+t15509+t15510+t15514+t15524+t15613+t15947+t15954+t15988+t15990+t16002+t16003+t16022+t16024)-q7d.*t16200-q6d.*t16287-q5d.*t16331+q4d.*t16348-q1d.*t16416-q3d.*(t4536.*(-8.8844724872e-2)-t20.*(t4540+t5.*(t2425-t2468)).*9.850206933e-2-t26.*(t4540+t5.*(t2425-t2468)).*9.850206933e-2+t2720.*t4507+(t583.*t7227)./2.0+(t4681.*t6431)./2.0+(t4255.*t9746)./2.0+(t4286.*t9732)./2.0+(t6175.*t9225)./2.0+(t6196.*t9212)./2.0-(t5699.*t9727)./2.0-(t5235.*t11372)./2.0+(t5234.*t11380)./2.0-(t8256.*t9212)./2.0+(t6302.*t11377)./2.0+(t6884.*t10973)./2.0+(t8640.*t10973)./2.0-(t6761.*t13382)./2.0-(t6811.*t13386)./2.0-(t9185.*t13177)./2.0-(t9194.*t13181)./2.0+t2716.*(t2425-t2468)+t2721.*(t2425-t2468)-(t6872.*(t9253-t44.*(t4540+t5.*(t2425-t2468))))./2.0+t14.*(t4540+t5.*(t2425-t2468)).*(t943-t1091).*6.12973e-1+(t14.*(t4540+t5.*(t2425-t2468)).*(t2821-t2864))./2.0)-q2d.*(t5536+t5542+t5619+t6181+t6510+t6560+t7339+t7363+t7803+t7804+t7877+t7944+t7945+t8283+t8381+t8421+t8968+t8974-t9339+t9372+t9674+t9678-t9826+t9854+t10056+t10076+t10230+t10273+t10969-t10986+t11015+t11067+t11434+t11553+t11563+t11663-t11669-t11711-t11741+t11906+t11913+t11989+t12078-t12234-t12245+t12311+t12463-t12632-t12641+t12741-t12977-t13131-t13133+t13480+t13493-t13499-t13587-t13744-t13889+t13986+t13989-t14143+t14423+t14424+t14714+t14718-t15084-t15283+(t4841.*(t4540+t5.*(t2425-t2468)))./4.0+(t9106.*(t10158+t16.*(t4542-t6448)))./4.0+(t8999.*(t10403+t9.*(t10158+t16.*(t4542-t6448)).*7.35522e-1))./4.0+(t1490.*(t5122+t5.*(t2425-t2468).*3.587895))./4.0+(t7105.*(t10384+t16.*(t4542-t6448).*1.666555))./4.0+(t10480.*(t10174+t9.*(t10158+t16.*(t4542-t6448))))./4.0+t14.*t5713.*(t4540+t5.*(t2425-t2468)).*3.064865e-1+(t14.*t8437.*(t4540+t5.*(t2425-t2468)))./4.0),q1d.*(-t5538-t5554-t5559-t5562-t6273-t6622-t7385-t7398-t7789-t7837-t7839-t7964-t8207+t8336+t8356+t8364+t8391+t8402+t8473-t8490-t8514+t8790+t8826+t9057+t9063+t9281+t9377+t9431+t9465-t9494-t9503-t9504-t9911-t9921+t10336+t10508+t11155+t11220+t11238+t11531+t11569-t11571+t11769-t11838+t11920-t12287-t12289+t12306-t12334+t12577+t13081+t13089+t13239+t13255+t13308-t13388-t13612+t13626+t13691-t13914-t13973-t13999+t14000-t14248-t14732+t14775+t14791-t14984+t15027+t15038-t15169+t15172-t15393+t15395+((t6853-t6864).*(t921+t1317-t5853))./4.0+(t11356.*(-t1476-t1540+t2091+t2165+t2579+t8.*(t260+t468+t570+t2298)))./4.0+(t13178.*(t3418-t3879+t4324-t5228+t5802+t9.*(t71-t391).*4.5305948634e-2+t17.*(t426-t581).*7.35522e-1))./4.0+(t13377.*(t1987-t2621+t3452-t4730+t5359+t9.*(t71-t391).*6.1597e-2+t17.*(t426-t581)))./4.0+(t5860.*(t6806-t8574))./4.0+(t6970.*(t6801-t8594))./4.0+(t8310.*(t6452-t8229))./4.0+(t9525.*(t6452-t8229))./4.0+(t8227.*(t6847-t9563))./4.0+(t9744.*(t6472-t9256))./4.0+(t8794.*(t263-t283-t310+t1265))./4.0+(t10942.*(-t3045-t3218+t3458+t3539+t3878+t8.*(t260+t468+t570+t2298).*1.666555))./4.0)+q5d.*(t7300-t7310-t7313-t7315+t9405+t9475+t10265+t10291+t11036+t11045+t11172+t11183+t11259+t11260+t11330-t11394+t11405+t11413-t11559+t11588+t11595+t11681+t11789+t11845+t11914+t11918+t12318+t12470+t12949+t12957+t13059+t13062+t13289+t13658+t13668+t13672+t13757+t13764+t14117+t14127+t14392+t14406+t14704+t14705+t14906+t14911+t16.*(t6472-t9256).*4.38178973375e-3+t16.*(t6847-t9563).*2.62925e-3+(t3421.*(t6834-t9565))./4.0+((t2904-t2927).*(t6472-t9256))./4.0)+q6d.*(t7311+t7321+t9797+t9809+t11884+t11990-t12944+t12959-t13045-t13054+t13064+t13106-t13110-t13147+t13274-t13280-t13319+t13352-t13367+t13389+t13397+t13498+t13509-t13713+t13972-t13977-t14671+t14680-t14846+t14848+(t5275.*(t6801-t8594))./4.0+(t6969.*(t6452-t8229))./4.0)-q7d.*t16203+q4d.*t16351+q3d.*(t20.*t6430.*(-9.850206933e-2)-t26.*t6430.*9.850206933e-2+t2716.*t4436+t2721.*t4436-(t583.*t7241)./2.0-(t4681.*t6447)./2.0-(t4286.*t9733)./2.0-(t6175.*t9226)./2.0-(t6196.*t9213)./2.0+(t5699.*t9728)./2.0+(t5235.*t11356)./2.0+(t8256.*t9213)./2.0+(t6872.*t10942)./2.0+(t6761.*t13371)./2.0+(t6811.*t13377)./2.0+(t9185.*t13175)./2.0+(t9194.*t13178)./2.0+(t4255.*(t6853-t6864))./2.0+(t5234.*(t6847-t9563))./2.0+(t6884.*(t6472-t9256))./2.0+(t6302.*(t6834-t9565))./2.0+(t8640.*(t6472-t9256))./2.0-t4.*t13.*(t2425-t2468).*1.26729164208e-1+t5.*t2712.*(t2425-t2468)+t14.*t6430.*(t943-t1091).*6.12973e-1+(t14.*t6430.*(t2821-t2864))./2.0)+phid.*(-t5538-t5554-t5559-t5562-t6273-t6622-t7789+t8193+t8790+t8826+t9057+t9063+t9377+t9431-t10331+t10339+t10373+t10519-t10526+t10558+t10574+t10650+t10898+t10905+t10908+t11220+t11238-t11392-t11526-t11527+t11531+t11569+t11722-t11732+t11769+t12051+t12072-t12297-t12302+t12306+t12559+t12832+t13081+t13089+t13239+t13255+t13308+t13691-t13936-t14110-t14129+t14231-t14357-t14359+t14548+t14775+t14791+t15027+t15038-t15264+t15265-t15402+t15420-t15441+t15442+t15503-t15513-t15527-t15612-t15956+t15959-t15991+t15992+t15998+t16017+(t8794.*(t263+t1265-t7252-t5.*t12.*1.0442e-1))./4.0+(t13178.*(t3418-t3879+t4324+t11855+t9.*(t71-t391).*4.5305948634e-2+t17.*(t426-t581).*7.35522e-1+t9.*(t9166-t11658).*7.35522e-1))./4.0+(t12385.*(t6853-t6864))./4.0+(t11247.*(t6806-t8574))./4.0+(t12185.*(t6452-t8229))./4.0+(t11720.*(t6801-t8594))./4.0+(t12669.*(t6452-t8229))./4.0+(t14380.*(t6472-t9256))./4.0+(t14057.*(t6847-t9563))./4.0+(t8166.*(t1786+t2973-t7703-t5.*t12.*3.746479959e-1))./4.0+(t13377.*(t1987-t2621+t3452+t11654+t9.*(t71-t391).*6.1597e-2+t17.*(t426-t581)+t9.*(t9166-t11658)))./4.0)-q2d.*(t5593+t5599+t5638+t6519+t7392+t7427+t7852-t7874+t7879+t7896+t7917+t7918-t8279+t8307+t8428+t8450+t8946+t8954-t9082-t9403+t9422+t9687+t9700+t9876-t9888+t10108+t10129+t10245+t10302-t10308+t10970+t11041+t11077+t11435+t11629+t11634+t11664-t11670-t11743+t11948+t11966+t12031+t12091-t12258+t12312+t12476-t12633+t12760-t13122-t13540-t13550+t13563+t13566-t13762-t13912-t13921+t14004+t14008-t14158+t14416+t14418+t14711+t14713-t15113-t15114-t15308-t15310+(t5634.*(t6853-t6864))./4.0+(t5648.*(t6806-t8574))./4.0+(t8053.*(t6452-t8229))./4.0+(t7079.*(t6847-t9563))./4.0+(t8191.*(t6834-t9565))./4.0+(t9110.*(t6472-t9256))./4.0+(t10141.*(t6472-t9256))./4.0+t12.*t3243.*(t2425-t2468).*8.07151e-1+(t12.*t4860.*(t2425-t2468))./4.0),-t16392-t16466+yd.*(t5538+t5554+t5559+t5562-t6622+t7789+t8207+t8776+t8806+t9051+t9058+t9390+t9445-t10331+t10339+t10373+t10519-t10526+t10558+t10574+t10650+t10898+t10905+t10908+t11226+t11229-t11392-t11526-t11527+t11537+t11557+t11722-t11732+t11777+t12051+t12072-t12297-t12302+t12310+t12559+t12832+t13086+t13093+t13246+t13261+t13309+t13696-t13936-t14110-t14129+t14231-t14357-t14359+t14548+t14778+t14788+t15029+t15035-t15264+t15265-t15402+t15420-t15441+t15442+t15503-t15513-t15527-t15612-t15956+t15959-t15991+t15992+t15998+t16017+(t8794.*(t263+t1265-t7252-t5.*t12.*1.0442e-1))./4.0+(t13178.*(t3418-t3879+t4324+t11855+t9.*(t71-t391).*4.5305948634e-2+t17.*(t426-t581).*7.35522e-1+t9.*(t9166-t11658).*7.35522e-1))./4.0+(t12385.*(t6853-t6864))./4.0+(t11247.*(t6806-t8574))./4.0+(t12185.*(t6452-t8229))./4.0+(t11720.*(t6801-t8594))./4.0+(t12669.*(t6452-t8229))./4.0+(t14380.*(t6472-t9256))./4.0+(t14057.*(t6847-t9563))./4.0+(t8166.*(t1786+t2973-t7703-t5.*t12.*3.746479959e-1))./4.0+(t13377.*(t1987-t2621+t3452+t11654+t9.*(t71-t391).*6.1597e-2+t17.*(t426-t581)+t9.*(t9166-t11658)))./4.0+t12.*(t881-t912).*(t2425-t2468).*8.07151e-1)+q1d.*(t3604-t3629+t3748-t4422-t4525+t4637+t4793+t4957-t5288-t5896+t5900+t5902+t5922+t5934+t5937+t6109+t6110-t6260+t6343+t6393-t6948+t7018-t7050-t7627+t7659+t7776-t7971+t7997+t8086+t8455+t8458+t8480+t8710+t8716-t8777-t8934-t9042+t9070-t9126-t9139+t9366-t9380-t9384+t9393-t9496-t9583-t9602+t9650+t9661-t9940+t9965+t9974-t10143+t10210+t10215+t10406+t10416-t10537+t11110+t11116+t11496+t11497+t11977+t11986+t12028+t12034+t12173+t12188+t12354+t12565+t12687+t12730-t13199+t13215-t13307+t13311-t13664+t13689+t13736+t13737-t13813+t13837-t13885-t13886+t13930+t13939+t13991-t14171-t14174+t14175-t14417-t14420-t14960-t14961+t14966+t14967+t15294+t15307+t15454+t15458+t15673+t15674+t15676+t15678+t15855+t15856+(t13627.*(-t1476-t1540+t2091+t2165+t2579+t8.*(t260+t468+t570+t2298)))./4.0+(t13313.*(t1589-t2213+t3195-t4346+t4355+t4748.*7.35522e-1+t2772.*(t71-t391)+t2775.*(t71-t391)))./4.0+(t6951.*(t71-t391))./2.0+(t539.*(t1912.*(-1.196e-3)-t1942+t2518+t3589+t696.*(t71-t391)+t891.*(t71-t391)))./2.0+(t8628.*(t1589-t2213-t4346+t4355+t9454+t11863+t2772.*(t71-t391)+t2775.*(t71-t391)))./4.0+(t9233.*(t3423+t3845+t3888+t3925+t4339+t9.*(t210+t2107+t7423+t9121).*7.35522e-1+t17.*(t9166-t11658).*7.35522e-1))./4.0+(t14035.*(t249-t391.*(1.1e+1./1.25e+2)-t1912.*4.252e-3+t3505+t5357+t693.*(t71-t391)+t784.*(t71-t391)))./4.0+(t10398.*(t249-t391.*(1.1e+1./1.25e+2)-t1912.*4.252e-3+t3505+t13496+t693.*(t71-t391)+t784.*(t71-t391)))./4.0+(t13038.*(-t3045-t3218+t3458+t3539+t3878+t8.*(t260+t468+t570+t2298).*1.666555))./4.0+(t10783.*(t2091+t2497+t2579+t2680+t3516+t9.*(t210+t2107+t7423+t9121)+t17.*(t9166-t11658)))./4.0+t5.*t12.*(-t3405+t4994+t5076).*2.01382560198e-1)+q7d.*t16270-q6d.*t16379-q5d.*t16428-q4d.*t16446+q2d.*(-t2886-t3335+t3442+t3518+t3568+t3602+t3605+t3679+t3707+t3892+t4100+t4115+t4126+t4224+t4264+t4293+t4497+t4606+t4626+t4665+t4736+t4742+t4834+t4898+t4901+t4972+t5018+t5237+t5278+t5873+t5890+t5892+t5953+t5963+t5998+t6065+t6071+t6072+t6088+t6118+t6120+t6153+t6186+t6192+t6231+t6291+t6584+t6596+t6678+t6741+t6745+t6894+t6946+t7015+t7059+t7179+t7184+t7208+t7239+t7349+t7403+t7410+t7465+t7499+t7593+t7712+t7757+t7801+t7811+t7878+t7923+t7946+t7953+t8035+t8079+t8157+t8197+t8322+t8345+t8441+t8456+t8493+t8503+t8550+t8577+t8607+t8703+t8732+t8832+t8858+t8928+t8940+t9006+t9030+t9055+t9061+t9116+t9178+t9184+t9200+t9455+t9577+t9586+t9616+t9909+t9914+t9917+t9919+t10313+t10322+t10478+t10500+t11078+t11079+t11465+t11469+t11506+t11893+t11905+t12100+t12106+t12472+t12480+t12530+t12630+t12869+t12882+t12887+t12891+t12931+t13155+t13604+t13607+t13631+t13640+t13657+t13680+t13730+t13753+t13878+t13883+t14124+t14126+t14247+t14274+t14275+t14284+t14285+t14340+t14709+t14710+t14917+t14920+t14922+t14923+t15286+t15292+t15320+t15321+t15332+t15333+t15589+t15590+t15591+t15592+t15830+t15831+t15832+t15833)-q3d.*(t2523+t3641+t3689+t4072+t4121+t4159+t4776+t4801+t4890+t4907+t5076.*8.8844724872e-2+t5979+t6060+t6087+t6229+t6410+t6441+t7065+t7159+t7192+t7219+t7462+t7536+t8052+t8175+t8298+t6.*(t263+t1265-t7252-t5.*t12.*1.0442e-1).*4.9251034665e-2+t2716.*t4959+t2721.*t4959+t2720.*t5016-t14.*t8272.*4.9251034665e-2-t14.*t9263.*1.3727e-2-(t583.*t9215)./2.0-(t4681.*t7734)./2.0+(t4255.*t12163)./2.0-(t4286.*t12185)./2.0+(t6175.*t11228)./2.0-(t6196.*t11247)./2.0+(t5699.*t12669)./2.0-(t5235.*t13627)./2.0+(t6884.*t13019)./2.0-(t6872.*t13038)./2.0+(t8256.*t11720)./2.0+(t6302.*t14035)./2.0+(t6761.*t15156)./2.0+(t8640.*t13313)./2.0+(t6811.*t15155)./2.0+(t9185.*t14823)./2.0+(t9194.*t14821)./2.0+(t5234.*(t3098+t3211-t3221+t3678+t8102+t10798))./2.0-(t10769.*(t943-t1091))./2.0-(t9285.*(t2821-t2864))./2.0+t6.*(t1786+t2973-t7703-t5.*t12.*3.746479959e-1).*1.3727e-2),-t16248-t16418-t16460+yd.*(t5538+t5554+t5559+t5562-t6622+t7372+t7789+t7820+t7954+t8207+t8336+t8356+t8364+t8391+t8402+t8473-t8490-t8514+t8776+t8806+t9051+t9058+t9281+t9390+t9445+t9465-t9494-t9503-t9504-t9911-t9921+t10336+t10508+t11155+t11226+t11229+t11537+t11557-t11571+t11777-t11838+t11920-t12287-t12289+t12310-t12334+t12577+t13086+t13093+t13246+t13261+t13309-t13388-t13612+t13626+t13696-t13914-t13973-t13999+t14000-t14248-t14732+t14778+t14788-t14984+t15029+t15035-t15169+t15172-t15393+t15395+((t6853-t6864).*(t921+t1317-t5853))./4.0+(t11356.*(-t1476-t1540+t2091+t2165+t2579+t8.*(t260+t468+t570+t2298)))./4.0+(t13178.*(t3418-t3879+t4324-t5228+t5802+t9.*(t71-t391).*4.5305948634e-2+t17.*(t426-t581).*7.35522e-1))./4.0+(t13377.*(t1987-t2621+t3452-t4730+t5359+t9.*(t71-t391).*6.1597e-2+t17.*(t426-t581)))./4.0+(t5860.*(t6806-t8574))./4.0+(t6970.*(t6801-t8594))./4.0+(t8310.*(t6452-t8229))./4.0+(t9525.*(t6452-t8229))./4.0+(t8227.*(t6847-t9563))./4.0+(t9744.*(t6472-t9256))./4.0+(t8794.*(t263-t283-t310+t1265))./4.0+(t10942.*(-t3045-t3218+t3458+t3539+t3878+t8.*(t260+t468+t570+t2298).*1.666555))./4.0+t12.*(t881-t912).*(t2425-t2468).*8.07151e-1-t5.*t12.*t6447.*2.01382560198e-1-t5.*t12.*t7236.*6.23745e-2)-q3d.*(t2523+t3641+t3689+t4072+t4121+t4159+t4776+t4801+t4890+t4907+t5979+t6060+t6087+t6229+t6410+t6441+t7065+t7159+t7192+t7219+t7462+t7536+t8052+t8175+t8298-t14.*t3643.*4.9251034665e-2-(t583.*t4905)./2.0-t14.*t5826.*1.3727e-2-t6.*t5843.*1.3727e-2-(t1920.*t4681)./2.0+(t5806.*t6175)./2.0-(t5860.*t6196)./2.0+(t4255.*t8285)./2.0-(t4286.*t8310)./2.0+(t6884.*t7402)./2.0-(t6872.*t7434)./2.0-(t5235.*t9269)./2.0+(t5699.*t9525)./2.0+(t6970.*t8256)./2.0+(t6302.*t10398)./2.0+(t8628.*t8640)./2.0+(t6761.*t10783)./2.0+(t6811.*t10787)./2.0+(t9185.*t9233)./2.0+(t9194.*t9252)./2.0+(t5234.*(t3098+t3199+t3211-t3221+t3678+t4612))./2.0-(t8609.*(t943-t1091))./2.0-(t5884.*(t2821-t2864))./2.0+t6.*(t263-t283-t310+t1265).*4.9251034665e-2)+q7d.*t16173-q6d.*t16249-q5d.*t16316-q4d.*t16340-q2d.*(t2886+t3335+t3393+t3451+t3491+t3553-t3602+t3642-t3707+t3844+t4095-t4100+t4148-t4224+t4241-t4293-t4294-t4296+t4472+t4570-t4626-t4665-t4736-t4742-t4834+t4886+t4911+t4963+t4998+t5070-t5093+t5222+t5268+t5458-t5469-t5525-t5526+t5667+t5669-t5873+t5881-t5998+t6026+t6035+t6036+t6050-t6072-t6088+t6099-t6118+t6129+t6163-t6186-t6231+t6305+t6585+t6594+t6669+t6728+t6755+t6870+t6921-t6992-t6993-t7001-t7015-t7059-t7184-t7208+t7225+t7238+t7302+t7317-t7349+t7390+t7393+t7421+t7453+t7456-t7478+t7487+t7607+t7692+t7747+t7787+t7793+t7888+t7898-t7923-t7930+t7931+t8087+t8145-t8197+t8311-t8345-t8456+t8481+t8695+t8727-t8832+t8840+t9002+t9025+t9311+t9381+t9428-t9860-t9872-t9898-t9902+t10086-t10109-t10110+t10116+t10183+t10184-t10385+t10417+t10420+t10456-t10605+t10641+t10814+t10819+t10860-t11206-t11213+t11224-t11249-t11250-t11273-t11274-t11600-t11606+t11616+t11619+t11631+t11637+t11912+t12140-t12418-t12419+t12650+t12658+t12660+t12661-t12871-t12872-t12878-t12884+t13298+t13300+(t7469.*(t1918+t9.*(t71-t391)))./4.0+(t8999.*(t3418-t3879+t4324-t5228+t5802+t9.*(t71-t391).*4.5305948634e-2+t17.*(t426-t581).*7.35522e-1))./4.0+(t10480.*(t1987-t2621+t3452-t4730+t5359+t9.*(t71-t391).*6.1597e-2+t17.*(t426-t581)))./4.0+(t1907.*(t618.*4.28e-4-t1841-t2389+t2400-t2414+t17.*(t113-t409).*1.0027e-2))./4.0+(t8063.*(t1589-t2213+t3195-t4346+t4355+t4748.*7.35522e-1+t2772.*(t71-t391)+t2775.*(t71-t391)))./4.0+(t5723.*(t71-t391))./4.0+(t6709.*(t71-t391))./4.0+(t7497.*(t60-t394))./4.0+(t3261.*(t2798-t2848))./4.0+(t10111.*(t249-t391.*(1.1e+1./1.25e+2)-t1912.*4.252e-3+t3505+t5357+t693.*(t71-t391)+t784.*(t71-t391)))./4.0+(t5750.*(t263-t283-t310+t1265))./4.0-(t5.*t6.*t5783)./4.0),-t16215+t16383+t16390+t16399+t16477+q6d.*t16241+q5d.*t16285+q4d.*t16327+q3d.*(t5.*(-3.356258116611425e-2)+t13.*4.442367301156758e-2-t6.*t3254.*4.9251034665e-2+(t13.*t3279)./2.0+t14.*t3292.*4.9251034665e-2+t5.*t3431+(t6.*t3861)./2.0-(t14.*t4473)./2.0+(t226.*t4415)./2.0+t5.*t4646-(t322.*t4471)./2.0+(t583.*t4841)./2.0-t6.*t5739.*1.3727e-2+t14.*t5755.*1.3727e-2-(t6.*t5831)./2.0-(t226.*t5847)./2.0+(t1490.*t4681)./2.0-(t483.*t5879)./2.0-(t227.*t6756)./2.0+(t323.*t6784)./2.0+(t323.*t7440)./2.0-(t440.*t7396)./2.0-(t1837.*t6687)./2.0+(t5613.*t6175)./2.0-(t5648.*t6196)./2.0+(t4255.*t8047)./2.0-(t4286.*t8053)./2.0+(t6884.*t7066)./2.0+(t6872.*t7105)./2.0+(t5234.*t9098)./2.0+(t5235.*t9106)./2.0-(t6654.*t8256)./2.0-(t5699.*t9333)./2.0+(t6302.*t10111)./2.0+(t8063.*t8640)./2.0+(t6761.*t10485)./2.0-(t6811.*t10480)./2.0+(t9001.*t9185)./2.0-(t8999.*t9194)./2.0-(t5866.*(t60-t394))./2.0-(t6653.*(t60-t394))./2.0+(t6615.*(t357-t519))./2.0+(t7469.*(t79-t358))./2.0-(t8438.*(t943-t1091))./2.0-(t5716.*(t2821-t2864))./2.0-(t5.*t14.*t2111)./2.0+(t14.*t15.*t5723)./2.0+(t7.*t14.*t5776)./2.0+(t14.*t15.*t6709)./2.0)+q7d.*(t1625.*1.563719772e-3+t4270-t4348-t4354-t4488+t4648-t4659+t5032+t5054-t5558+t5570+t5995+t6268+t6327+t6534+t6544+t6612+t7319+t7451+t7855+t7900+t9960+t10359+t10553+t11202+t11223+t11275+t11297+t11309+t11555+t11594+t11632+t11638+t9.*(t236-t451).*3.867742437e-3),-q7d.*t16104-q6d.*t16130-q4d.*t16159+q5d.*(t3633+t3726-t3746+t4595-t4642+t4830-t4966+t4993-t5977+t6037-t6056-t6130-t6131+t6269-t6334-t6679+t6697+t6774+t6978-t7060-t7170+t7175-t8168+t8180-t8511+t8521-t8809-t9232+t10278+t10279+t10520-t10540+t10771-t10776+(t5990.*(t79-t358))./2.0),t16160+t16326-t16342-t16448+yd.*(t6999+t7020-t7671+t7995+t8667+t9389-t9402-t9415-t9444-t9473-t9484+t9776+t9814+t10023+t10040+t10044+t10049-t10060+t10372+t10529+t10992+t11198+t11379+t11729+t11936+t11940+t12114+t12131+t12154-t12180+t12363-t12436+t12822-t13053-t13066-t13220-t13227-t13301-t13678+t13900+t13944+t13946+t14128+t14134+t14194+t14745-t14749+t15007-t15014+(t6430.*(t1748-t1821))./4.0+(t4064.*(t6806-t8574))./4.0+(t5646.*(t6452-t8229))./4.0+(t5234.*(t8589-t8592))./4.0+(t6884.*(t8219-t8226))./4.0+(t6302.*(t8582-t8586))./4.0+(t8640.*(t8219-t8226))./4.0+(t6761.*(t8583-t11188))./4.0+(t9185.*(t8221-t11008))./4.0)-q7d.*t16138+q5d.*t16237+xd.*(t7036+t7056-t7658+t8022+t8678-t9347+t9360-t9412+t9775+t9813+t10020+t10022+t10025+t10043+t10371+t10528+t10968+t11177-t11186+t11351-t11367+t11698+t11946+t11949+t12105-t12129-t12135+t12144+t12165+t12370-t12408-t12416-t12471+t12830-t12870-t13041-t13200-t13283-t13653-t13873+t13877+t13950+t13951+t14135+t14141+t14176-t14177+t14738+t14995+(t6677.*(t10158+t16.*(t4542-t6448)))./4.0+(t6540.*(t10403+t9.*(t10158+t16.*(t4542-t6448)).*7.35522e-1))./4.0+(t536.*(t5122+t5.*(t2425-t2468).*3.587895))./4.0+((t923-t1076).*(t5110-t6808))./4.0+((t2812-t2860).*(t4542-t6448))./4.0+(t5050.*(t10384+t16.*(t4542-t6448).*1.666555))./4.0+(t9048.*(t10174+t9.*(t10158+t16.*(t4542-t6448))))./4.0+t15.*t4286.*(t4542-t6448).*3.064865e-1+(t15.*t6196.*(t4542-t6448))./4.0)+q6d.*(t3775+t3786+t3787+t3920+t4029+t4037+t4091+t4106+t4132+t4182+t4207+t4240+t4247-t4891-t4926+t4961+t5036+t5146-t5372-t5398+t5421-t5678-t5816-t5817+t6004+t6023-t6086+t6705+t6722+t6754+t6842+t6882+t7285-t7298-t7325-t7333+t7431+t7447+t7678-t7716-t7729+t7762-t7766-t7770-t8247+t8489-t8744+t9018+t9027+t9191+t9282+t9287+t9461+t9479+t9493-t9516-t9517-t9646-t9671-t9683+t10135+t10136-(t9.*t323.*t5763)./4.0-(t17.*t323.*t5837)./4.0),t16144-t16286-t16318-t16336-t16430+q7d.*t16128-q6d.*t16167-q4d.*t16237+xd.*(-t7281-t7284+t7345+t9363+t9413+t10264+t10290+t11012+t11019+t11131+t11145+t11222+t11225+t11291+t11368+t11375-t11412-t11428+t11541+t11545-t11581-t11591+t11641+t11768+t11831-t11869-t11883+t11900+t11903+t12300+t12449+t12918+t12930+t13044+t13050+t13267+t13646+t13677+t13681+t13763+t13777+t14111+t14115+t14370+t14386+t14691+t14693+t14886+t14890+t6.*t15.*(t4540+t5.*(t2425-t2468)).*7.326866269e-3),t16131+t16240+t16251+t16289+t16292+t16381-q7d.*(t3825+t3853-t3990-t4067+t4099+t4153+t4160+t4186+t4273+t4372+t4423-t5547+t5671+t6595+t6623-t6671-t6773-t7738-t7781+t7992-t8214+t8334+t8354+t8404-t9519-t9530+(t3239.*(t79-t358))./4.0+(t3280.*(t79-t358))./4.0+(t8640.*(t701-t775))./4.0)+q5d.*t16167-q4d.*(t3775+t3786+t3787+t3920+t4029+t4037+t4091+t4106+t4132+t4182+t4207+t4240+t4247-t4891-t4926+t4961+t5036+t5146-t5372-t5398+t5421-t5678-t5816-t5817+t6004+t6023-t6086+t6705+t6722+t6754+t6842+t6882+t7285-t7298-t7325-t7333+t7431+t7447+t7678-t7716-t7729+t7762-t7766-t7770-t8247+t8489-t8744+t9018+t9027+t9191+t9282+t9287+t9461+t9479+t9493-t9516-t9517-t9646-t9671-t9683+t10135+t10136-(t9.*t323.*t5763)./4.0-(t17.*t323.*t5837)./4.0),t16105-t16163+t16174-t16202-t16205+t16271+q6d.*(t3825+t3853-t3990-t4067+t4099+t4153+t4160+t4186+t4273+t4372+t4423-t5547+t5671+t6595+t6623-t6671-t6773-t7738-t7781+t7992-t8214+t8334+t8354+t8404-t9519-t9530+(t3239.*(t79-t358))./4.0+(t3280.*(t79-t358))./4.0+(t8640.*(t701-t775))./4.0)-q5d.*t16128+q4d.*t16138,q5d.*(t8804+t8829+t9145+t9354-t10997-t10998+t11097+t11101+t11270+t11284+t11370+t11376-t11511-t11517+t11533+t11535-t11550+t11836+t11844-t12393-t12803-t12903-t13160+t13243+t13244+t13328+t13331-t13538+t13926+t13928+t14116+t14121+t14584+t14754+(t5441.*(t10158+t16.*(t4542-t6448)))./4.0+(t5213.*(t10403+t9.*(t10158+t16.*(t4542-t6448)).*7.35522e-1))./4.0+(t3266.*(t5110-t6808))./4.0+(t4879.*(t4542-t6448))./4.0+(t3780.*(t10384+t16.*(t4542-t6448).*1.666555))./4.0+(t7538.*(t10174+t9.*(t10158+t16.*(t4542-t6448))))./4.0)-q7d.*(t8863+t8883+t11354+t11371-t13105-t13266+t14530+t14539-t14599+t14684+t14687-t14797+(t5345.*(t10403+t9.*(t10158+t16.*(t4542-t6448)).*7.35522e-1))./4.0+(t7797.*(t10174+t9.*(t10158+t16.*(t4542-t6448))))./4.0)+q4d.*(t4542.*3.746479959e-1-t4544.*1.9076837715e-1-t1744.*t6431-t1827.*t6431-(t3424.*t8741)./2.0-(t5331.*t8077)./2.0+(t4021.*t11341)./2.0-(t4024.*t11338)./2.0-(t6046.*t10920)./2.0+(t6069.*t10936)./2.0+(t5696.*t11340)./2.0-(t5329.*t12945)./2.0+(t5345.*t12953)./2.0+(t8477.*t10936)./2.0-(t7796.*t12689)./2.0+(t7797.*t12705)./2.0+t21.*(t4542-t6448).*4.23641577598e-1+t27.*(t4542-t6448).*4.23641577598e-1+t15.*t3752.*(t4542-t6448).*8.332775e-1+(t15.*t5443.*(t4542-t6448))./2.0)-phid.*(t5292+t5293+t7037+t7057+t9488+t9635+t10632+t10663+t10834+t10839+t11128+t11316-t12230+t12246+t12314-t12541+t12547-t12593-t12625+t12700+t12873+t12885+t13092+t13097+t13192-t13254-t13453-t13465+t13652+t13721+t13739-t13754-t13765+t13953+t14036+t14149+t14306+t14631+t14632+t14832+t14840-t15211-t15339-t15390-t15410-t15412-t15492-t15493-t15497+t15901+t15949+(t5598.*(t4540+t5.*(t2425-t2468)))./4.0+(t13380.*(t10158+t16.*(t4542-t6448)))./4.0+(t14541.*(t10403+t9.*(t10158+t16.*(t4542-t6448)).*7.35522e-1))./4.0+(t12689.*(t3418-t3879+t4324+t11855+t9.*(t71-t391).*4.5305948634e-2+t17.*(t426-t581).*7.35522e-1+t9.*(t9166-t11658).*7.35522e-1))./4.0+(t2701.*(t5122+t5.*(t2425-t2468).*3.587895))./4.0+(t9830.*(t5124-t6795))./4.0+(t9884.*(t5110-t6808))./4.0+(t10964.*(t4542-t6448))./4.0+(t10936.*(t1589-t2213-t4346+t4355+t9454+t11863+t2772.*(t71-t391)+t2775.*(t71-t391)))./4.0+(t12705.*(t3423+t3845+t3888+t3925+t4339+t9.*(t210+t2107+t7423+t9121).*7.35522e-1+t17.*(t9166-t11658).*7.35522e-1))./4.0+(t12867.*(t10384+t16.*(t4542-t6448).*1.666555))./4.0+(t11340.*(t249-t391.*(1.1e+1./1.25e+2)-t1912.*4.252e-3+t3505+t13496+t693.*(t71-t391)+t784.*(t71-t391)))./4.0+(t14918.*(t10174+t9.*(t10158+t16.*(t4542-t6448))))./4.0+(t12953.*(t2091+t2497+t2579+t2680+t3516+t9.*(t210+t2107+t7423+t9121)+t17.*(t9166-t11658)))./4.0+(t12945.*(t1987-t2621+t3452+t11654+t9.*(t71-t391).*6.1597e-2+t17.*(t426-t581)+t9.*(t9166-t11658)))./4.0+t15.*t12396.*(t4542-t6448).*3.064865e-1+(t15.*t13140.*(t4542-t6448))./4.0)+q6d.*t16274+q3d.*t16348+q2d.*t16362+q1d.*(-t5292-t5293-t7037-t7057+t8240+t8799+t9480+t9620+t9626+t9636+t9708+t9729+t9780+t10012+t10046+t10138+t10325+t10326+t10448+t10631+t10643+t10668+t10682+t10838+t10843+t10983+t11138+t11241+t11325+t11692+t11701+t11873+t11885+t12122+t12190+t12231+t12255+t12608+t12876+t12880+t12966+t12971+t13094+t13095+t13193+t13348+t13359+t13373+t13425+t13432+t13655+t13727+t13733+t13850+t13969+t14140+t14511+t14512+t14630+t14634+t14766+t14774+t14834+t14836+t15139+t15144+t15377+t15379),phid.*t16452+q7d.*t16194-q5d.*t16312+q3d.*t16351+q1d.*t16410-q4d.*(t4664.*1.9076837715e-1+t6460.*3.746479959e-1+t6475.*1.9076837715e-1+t21.*(t6460-t35.*(t2425-t2468)).*4.23641577598e-1+t27.*(t6460-t35.*(t2425-t2468)).*4.23641577598e-1+(t3424.*t8792)./2.0+(t5331.*t8166)./2.0+(t4024.*t11390)./2.0+(t6046.*t10974)./2.0+(t5329.*t12987)./2.0+(t7796.*t12738)./2.0-t35.*(t2425-t2468).*3.746479959e-1+(t4021.*(t8589-t8592))./2.0+(t6069.*(t8219-t8226))./2.0+(t5696.*(t8582-t8586))./2.0+(t8477.*(t8219-t8226))./2.0+(t5345.*(t8583-t11188))./2.0+(t7797.*(t8221-t11008))./2.0+t15.*t3752.*(t6460-t35.*(t2425-t2468)).*8.332775e-1+(t15.*t5443.*(t6460-t35.*(t2425-t2468)))./2.0)+q2d.*(t5297+t7682+t7739-t9159+t9258+t9265+t9399+t9438+t9529+t9541-t9573+t9662+t9873+t9899+t9993+t9994+t9995+t10251+t10477+t10887+t10897+t11090+t11279+t11442+t11447+t11620+t11767+t11783+t11785+t11851+t11929+t12437+t12445+t12644+t12647+t12986+t13136+t13144+t13190+t13259+t13265+t13556+t13580+t13589+t13592+t13599+t14003+t14229+t14239+t14486+t14491+t14957+t14959+t15190+t15195+(t7796.*(t9.*(t16.*(t30.*(t2425-t2468)+t68.*(t2425-t2468))+t8.*(t7.*(t4650+t34.*(t2425-t2468))+t47.*(t2425-t2468)))+t17.*(t4654+t15.*(t4650+t34.*(t2425-t2468)))))./4.0+(t5331.*(t30.*(t2425-t2468)+t68.*(t2425-t2468)))./4.0+(t6046.*(t16.*(t30.*(t2425-t2468)+t68.*(t2425-t2468))+t8.*(t7.*(t4650+t34.*(t2425-t2468))+t47.*(t2425-t2468))))./4.0+(t4024.*(t16.*(t30.*(t2425-t2468)+t68.*(t2425-t2468)).*1.666555+t8.*(t7.*(t4650+t34.*(t2425-t2468))+t47.*(t2425-t2468)).*1.666555))./4.0+t7.*(t7.*(t4650+t34.*(t2425-t2468)).*1.225946+t47.*(t2425-t2468).*1.225946).*8.639075e-2+t30.*(t2425-t2468).*9.5384188575e-2+t34.*(t2425-t2468).*1.8732399795e-1+t68.*(t2425-t2468).*9.5384188575e-2+(t3424.*(t30.*(t2425-t2468).*1.225946+t68.*(t2425-t2468).*1.225946))./4.0+t15.*(t4654+t15.*(t4650+t34.*(t2425-t2468))).*1.059103943995e-1+(t5443.*(t4654+t15.*(t4650+t34.*(t2425-t2468))))./4.0+t7.*(t7.*(t4650+t34.*(t2425-t2468))+t47.*(t2425-t2468)).*1.059103943995e-1+(t5329.*(t9.*(t16.*(t30.*(t2425-t2468)+t68.*(t2425-t2468))+t8.*(t7.*(t4650+t34.*(t2425-t2468))+t47.*(t2425-t2468))).*7.35522e-1+t17.*(t4654+t15.*(t4650+t34.*(t2425-t2468))).*7.35522e-1))./4.0)-q6d.*(t8890-t8893-t8900-t8911+t11074+t11085+t12723+t12726+t12820+t12829+t12874+t12877+t12896-t13006+t13021+t13034+t13084+t13099+t13103-t13132+t13194+t13495+t13502+t13659+t14528+t14538+t14638+t14639+t17.*(t8221-t11008).*1.13264871585e-2+t17.*(t8583-t11188).*1.539925e-2+(t3489.*(t8582-t8586))./4.0+(t5365.*(t8219-t8226))./4.0),-t16373+t16450+t16454+q7d.*t16265-q6d.*t16378-q5d.*t16425-q3d.*t16446-q2d.*t16455-q1d.*(t4831+t5358+t5377+t5506+t5591+t5594+t5767+t5926+t5959+t6083+t6861+t6962+t7012+t7072+t7107+t7324+t7380+t7661+t7663+t7709+t7725+t8074+t8098+t8629+t8815+t8961+t8990+t9054+t9089+t9864+t9983+t10148+t10701-t11268+t11269+t11383+t11401+t11458-t11461+t11463-t11474+t11574+t11584+t11655-t11657+t11898+t12021-t12317-t12454-t12597+t12609-t12828+t12844+t13221+t13420+t13564+t13570-t13633+t13637+t13719+t13723-t13845+t13848+t13859+t14078+t14132+t14188-t14296+t14298-t14347+t14348-t14847-t14849-t14878-t14880+t15163+t15164+t15318+t15326-t15605-t15606+t15849+t15850+(t6190.*(-t1053-t3327+t5081.*1.225946+t7731+t15.*t223.*1.4653732538e-2))./4.0+(t14541.*(t3418-t3879+t4324-t5228+t5802+t9.*(t71-t391).*4.5305948634e-2+t17.*(t426-t581).*7.35522e-1))./4.0+(t9187.*(t3418-t3879+t4324+t11855+t9.*(t71-t391).*4.5305948634e-2+t17.*(t426-t581).*7.35522e-1+t9.*(t9166-t11658).*7.35522e-1))./4.0+(t14918.*(t1987-t2621+t3452-t4730+t5359+t9.*(t71-t391).*6.1597e-2+t17.*(t426-t581)))./4.0+(t13273.*(t1589-t2213+t3195-t4346+t4355+t4748.*7.35522e-1+t2772.*(t71-t391)+t2775.*(t71-t391)))./4.0+(t10501.*(t985+t3399-t13.*t42.*1.01140545e-1-t7.*t223.*5.034347249e-2))./4.0+(t8433.*(t1589-t2213-t4346+t4355+t9454+t11863+t2772.*(t71-t391)+t2775.*(t71-t391)))./4.0+(t13974.*(t249-t391.*(1.1e+1./1.25e+2)-t1912.*4.252e-3+t3505+t5357+t693.*(t71-t391)+t784.*(t71-t391)))./4.0+(t10096.*(t249-t391.*(1.1e+1./1.25e+2)-t1912.*4.252e-3+t3505+t13496+t693.*(t71-t391)+t784.*(t71-t391)))./4.0+(t10753.*(t1987-t2621+t3452+t11654+t9.*(t71-t391).*6.1597e-2+t17.*(t426-t581)+t9.*(t9166-t11658)))./4.0)+q4d.*(t3271+t3297+t3326+t3353+t3802+t3910+t3985+t4882-t5079.*3.746479959e-1+t5081.*1.9076837715e-1+t5261+t5276+t5573+t5623+t6440+t6631+t6672+t6688+t6739+t6751+t7275.*1.9076837715e-1+t7278.*3.746479959e-1+t8140+t8209+t8318+(t3424.*(-t1053-t3327+t5081.*1.225946+t7731+t15.*t223.*1.4653732538e-2))./2.0+t13.*t35.*3.090845966175e-2-t13.*t42.*1.5738391114875e-2+t7.*t10408.*2.11820788799e-1+t15.*t10441.*2.11820788799e-1+t7.*t11336.*1.727815e-1+t15.*t11343.*1.727815e-1-(t5331.*t9884)./2.0-(t3752.*t11969)./2.0-(t5443.*t10871)./2.0+(t4021.*t13376)./2.0-(t4024.*t13380)./2.0-(t6046.*t12867)./2.0+(t6069.*t12860)./2.0+(t5696.*t13974)./2.0-(t5329.*t14918)./2.0-(t5345.*t14919)./2.0+(t8477.*t13273)./2.0-(t7796.*t14541)./2.0-(t7797.*t14542)./2.0),